simulink library "outp"  (R2021b)
(part 9 of 10)

  VOUTP_EDriveSysErrShifterErr_flg : Outport  Port=497
  VOUTP_LVSysErrPwrOutErr_flg : Outport  Port=498
  VOUTP_HVRlyOpFail_flg : Outport  Port=499
  VOUTP_MCUActDisFail_flg : Outport  Port=500
  VOUTP_VCUBrkSWSta_enum : Outport  Port=501
  VOUTP_VCUFLDoorSta_flg : Outport  Port=502
  VOUTP_VCUFRDoorSta_flg : Outport  Port=503
  VOUTP_VCURLDoorSta_flg : Outport  Port=504
  VOUTP_VCURRDoorSta_flg : Outport  Port=505
  VOUTP_SysAllowReadySta_flg : Outport  Port=506
  VOUTP_VCUHoodSWSta_flg : Outport  Port=507
  VOUTP_VCUTailgateSWSta_flg : Outport  Port=508
  VOUTP_CAN1BusErrorDTC_raw32 : Outport  Port=509
  VOUTP_CAN2BusErrorDTC_raw32 : Outport  Port=510
  VOUTP_CAN3BusErrorDTC_raw32 : Outport  Port=511
  VOUTP_CAN4BusErrorDTC_raw32 : Outport  Port=512
  VOUTP_CAN5BusErrorDTC_raw32 : Outport  Port=513
  VOUTP_CAN6BusErrorDTC_raw32 : Outport  Port=514
  VOUTP_ActAPSPosn_pct : Outport  Port=515
  VOUTP_EAPS1MIN_pct : Outport  Port=516
  VOUTP_EAPS2MIN_pct : Outport  Port=517
  VOUTP_ResetPedalZeroPosStart_flg : Outport  Port=518
  VOUTP_EAPS1NRM_pct : Outport  Port=519
  VOUTP_EAPS2NRM_pct : Outport  Port=520
  VOUTP_DKCTimeSN_cnt : Outport  Port=521
  VOUTP_DKCAuthSta_enum : Outport  Port=522
  VOUTP_TimeSNDKCFbk_cnt : Outport  Port=523
  VOUTP_KeyMissSta_flg : Outport  Port=524
  VOUTP_KeyModeSta_enum : Outport  Port=525
  VOUTP_DkeyShowIVISta_enum : Outport  Port=526
  VOUTP_KeyAreaPS_enum : Outport  Port=527
  VOUTP_KeyAreaLockUnlock_enum : Outport  Port=528
  VOUTP_PCommandToBCM_enum : Outport  Port=529
  VOUTP_DKeyWelcomeSta_enum : Outport  Port=530
  VOUTP_KeyAreaPTG_enum : Outport  Port=531
  VOUTP_KeyAreaSPTGSta_enum : Outport  Port=532
  VOUTP_UIDLowPowerSta_enum : Outport  Port=533
  VOUTP_DkeyAreaRAPSSta_enum : Outport  Port=534
  VOUTP_ParkingModeCmd_enum : Outport  Port=535
  VOUTP_KeyNumSta_enum : Outport  Port=536
  VOUTP_KeyTypeSta_enum : Outport  Port=537
  VOUTP_FDCDKCAllowSleep_flg : Outport  Port=538
  VOUTP_DISCTurn_flg : Outport  Port=539
  VOUTP_DISCTargetSpd_kph : Outport  Port=540
  VOUTP_DISCSta_enum : Outport  Port=541
  VOUTP_DISCButtSta_flg : Outport  Port=542
  VOUTP_AllCANTxReq_flg : Outport  Port=543
  VOUTP_NMmTxReq_flg : Outport  Port=544
  VOUTP_Awake_enum : Outport  Port=545
  VOUTP_CSB_flg : Outport  Port=546
  VOUTP_ErrorState_enum : Outport  Port=547
  VOUTP_NodeID_enum : Outport  Port=548
  VOUTP_PNI_flg : Outport  Port=549
  VOUTP_RptMsgReq_flg : Outport  Port=550
  VOUTP_WakeUp_enum : Outport  Port=551
  VOUTP_ActiveWU_flg : Outport  Port=552
  VOUTP_SysNMmSta_enum : Outport  Port=553
  VOUTP_NetworkReq_flg : Outport  Port=554
  VOUTP_PowerUpState_enum : Outport  Port=555
  VOUTP_PowerDownState_enum : Outport  Port=556
  VOUTP_PowerUpFault_enum : Outport  Port=557
  VOUTP_PowerDownFault_enum : Outport  Port=558
  VOUTP_ActiveDischargeReq_flg : Outport  Port=559
  VOUTP_DCDCEnaReq_flg : Outport  Port=560
  VOUTP_DCDCVoltSetpoint_V : Outport  Port=561
  VOUTP_HVBatCnctReq_flg : Outport  Port=562
  VOUTP_HVSysReadyToCharge_enum : Outport  Port=563
  VOUTP_PowerSta_enum : Outport  Port=564
  VOUTP_LVPwrSta_flg : Outport  Port=565
  VOUTP_HVPwrSta_flg : Outport  Port=566
  VOUTP_SysPowerMode_enum : Outport  Port=567
  VOUTP_FrMCUEnaReq_flg : Outport  Port=568
  VOUTP_RrMCUEnaReq_flg : Outport  Port=569
  VOUTP_DrivetrainSelect_enum : Outport  Port=570
  VOUTP_DrSeatSta_enum : Outport  Port=571
  VOUTP_PwrStaSelect_enum : Outport  Port=572
  VOUTP_PwrStaConstraint_enum : Outport  Port=573
  VOUTP_TCountSta_enum : Outport  Port=574
  VOUTP_PwrUpReq_enum : Outport  Port=575
  VOUTP_PwrDownReq_enum : Outport  Port=576
  VOUTP_LowSOCWarn_enum : Outport  Port=577
  VOUTP_ReVehThdChkSta_enum : Outport  Port=578
  VOUTP_EvccAplusPwrUpReq_flg : Outport  Port=579
  VOUTP_PwrStaONTOPopReq_flg : Outport  Port=580
  VOUTP_IVIPwrStaONTOPopT_s : Outport  Port=581
  VOUTP_LVChrgHoldTtimer_s : Outport  Port=582
  VOUTP_LVBattChrgTimeCnt_s : Outport  Port=583
  VOUTP_SilentChkAllowSleep_flg : Outport  Port=584
  VOUTP_TimerAllowSleep_flg : Outport  Port=585
  VOUTP_FDADC12VDetAvg_mV : Outport  Port=586
  VOUTP_PMMAllowECUSleep_flg : Outport  Port=587
  VOUTP_LVSilentChrgSta_enum : Outport  Port=588
  VOUTP_LVSilentChrgReq_flg : Outport  Port=589
  VOUTP_LVSilentChrgLv_enum : Outport  Port=590
  VOUTP_CtrlFrPwrStbA1P_flg : Outport  Port=591
  VOUTP_CtrlFrRC1_flg : Outport  Port=592
  VOUTP_CtrlFrBMSCCUCIR_flg : Outport  Port=593
  VOUTP_CtrlFrEDUINVERTER_flg : Outport  Port=594
  VOUTP_HWResetSta_enum : Outport  Port=595
  VOUTP_CtrlDrPwrStbA2_flg : Outport  Port=596
  VOUTP_PwrStaTOSta_enum : Outport  Port=597
  VOUTP_Sched_ChgTOSta_enum : Outport  Port=598
  VOUTP_PwrReq_OTA_enum : Outport  Port=599
  VOUTP_OTAPwrReqOFFChkSta_enum : Outport  Port=600
  VOUTP_OTAPwrReqStdChkSta_enum : Outport  Port=601
  VOUTP_PwrReqRAPSAvail_flg : Outport  Port=602
  VOUTP_HWVer1_cnt : Outport  Port=603
  VOUTP_HWVer2_cnt : Outport  Port=604
  VOUTP_HWVer3_cnt : Outport  Port=605
  VOUTP_CarModel1_cnt : Outport  Port=606
  VOUTP_CarModel2_cnt : Outport  Port=607
  VOUTP_CarModel3_cnt : Outport  Port=608
  VOUTP_ECU1_cnt : Outport  Port=609
  VOUTP_ECU2_cnt : Outport  Port=610
  VOUTP_Major1_cnt : Outport  Port=611
  VOUTP_Major2_cnt : Outport  Port=612
  VOUTP_Minor1_cnt : Outport  Port=613
  VOUTP_Minor2_cnt : Outport  Port=614
  VOUTP_Patch1_cnt : Outport  Port=615
  VOUTP_Patch2_cnt : Outport  Port=616
  VOUTP_Country1_cnt : Outport  Port=617
  VOUTP_Country2_cnt : Outport  Port=618
  VOUTP_Variation_cnt : Outport  Port=619
  VOUTP_Dash1_cnt : Outport  Port=620
  VOUTP_Change1_cnt : Outport  Port=621
  VOUTP_Change2_cnt : Outport  Port=622
  VOUTP_Dash2_cnt : Outport  Port=623
  VOUTP_SHA1_cnt : Outport  Port=624
  VOUTP_SHA2_cnt : Outport  Port=625
  VOUTP_SHA3_cnt : Outport  Port=626
  VOUTP_SHA4_cnt : Outport  Port=627
  VOUTP_SHA5_cnt : Outport  Port=628
  VOUTP_SHA6_cnt : Outport  Port=629
  VOUTP_SHA7_cnt : Outport  Port=630
  VOUTP_SHA8_cnt : Outport  Port=631
  VOUTP_NvWriteReqRisingEdge_flg : Outport  Port=632
  VOUTP_FdcSlpReqRisingEdge_flg : Outport  Port=633
  VOUTP_FdcSlpTime_sec : Outport  Port=634
  VOUTP_PmicBootReason_enum : Outport  Port=635
  VOUTP_WisrBootReason_raw32 : Outport  Port=636
  VOUTP_AcoreRebootCmdACK_flg : Outport  Port=637
  VOUTP_CurrentNmState_enum : Outport  Port=638
  VOUTP_ECUGen1_cnt : Outport  Port=639
  VOUTP_ECUGen2_cnt : Outport  Port=640
  VOUTP_PmicBootPath_raw32 : Outport  Port=641
  VOUTP_DrivingMode_cnt : Outport  Port=642
  VOUTP_ModelYear_cnt : Outport  Port=643
  VOUTP_Var4_cnt : Outport  Port=644
  VOUTP_Var5_cnt : Outport  Port=645
  VOUTP_FDCompCmd_rpm : Outport  Port=646
  VOUTP_FDSOV1Cmd_flg : Outport  Port=647
  VOUTP_FDSOV2Cmd_flg : Outport  Port=648
  VOUTP_FDSOV3Cmd_flg : Outport  Port=649
  VOUTP_FDEXV1Cmd_step : Outport  Port=650
  VOUTP_FDEXV2Cmd_step : Outport  Port=651
  VOUTP_FDSOTXVCmd_flg : Outport  Port=652
  VOUTP_FDFWVCmd_flg : Outport  Port=653
  VOUTP_FDTWVCmd_pct : Outport  Port=654
  VOUTP_FDFrWPTCHeatPwrCmd_W : Outport  Port=655
  VOUTP_CoolgFanActDuty_pct : Outport  Port=656
  VOUTP_FDAGSCmd_enum : Outport  Port=657
  VOUTP_FDEWP1Cmd_enum : Outport  Port=658
  VOUTP_FDEWP2Cmd_enum : Outport  Port=659
  VOUTP_FDEWP3Cmd_enum : Outport  Port=660
  VOUTP_FDFrLeAPTCHeatPwrCmd_W : Outport  Port=661
  VOUTP_FDFrRiAPTCHeatPwrCmd_W : Outport  Port=662
  VOUTP_FDRrAPTCHeatPwrCmd_W : Outport  Port=663
  VOUTP_FDBlowerCmd_pct : Outport  Port=664
  VOUTP_BatteryMode_enum : Outport  Port=665
  VOUTP_EDriveMode_enum : Outport  Port=666
  VOUTP_CabinMode_enum : Outport  Port=667
  VOUTP_CCUACLampSts_flg : Outport  Port=668
  VOUTP_CCUAutoLampSts_flg : Outport  Port=669
  VOUTP_CCUACMaxLampSts_flg : Outport  Port=670
  VOUTP_CCUSyncLampSts_flg : Outport  Port=671
  VOUTP_sigAirIntenZon1St_enum : Outport  Port=672
  VOUTP_sigWindDirZon1St_enum : Outport  Port=673
  VOUTP_sigRecircSt_flg : Outport  Port=674
  VOUTP_sigSetTempZon1St_C : Outport  Port=675
  VOUTP_sigSetTempZon2St_C : Outport  Port=676
  VOUTP_sigClntTHvBattOut_C : Outport  Port=677
  VOUTP_sigCbnSolarLeft_W : Outport  Port=678
  VOUTP_sigClntTHvBattIn_C : Outport  Port=679
  VOUTP_sigCbnSolarRight_W : Outport  Port=680
  VOUTP_sigAmbAirT_C : Outport  Port=681
  VOUTP_sigCbnAirT_C : Outport  Port=682
  VOUTP_ACSubMode_enum : Outport  Port=683
  VOUTP_FDRecyAutoCmd_enum : Outport  Port=684
  VOUTP_ACModeMem_enum : Outport  Port=685
  VOUTP_Face_flg : Outport  Port=686
  VOUTP_Foot_flg : Outport  Port=687
  VOUTP_Frost_flg : Outport  Port=688
  VOUTP_FaceM_flg : Outport  Port=689
  VOUTP_FootM_flg : Outport  Port=690
  VOUTP_CCUSyncSts_flg : Outport  Port=691
  VOUTP_ACForceOFF_flg : Outport  Port=692
  VOUTP_RecAutoFlg_flg : Outport  Port=693
  VOUTP_AirIntenZone1M_enum : Outport  Port=694
  VOUTP_fdefog_flg : Outport  Port=695
  VOUTP_sigSetTempZon2StM_C : Outport  Port=696
  VOUTP_sigDfrstSt_flg : Outport  Port=697
  VOUTP_FDCTHCAirIntZ3Sta_enum : Outport  Port=698
  VOUTP_FDCTHCDrEVentModeSta_enum : Outport  Port=699
  VOUTP_FDCTHCPsEVentModeSta_enum : Outport  Port=700
  VOUTP_FDCTHCDrEVentZSta_enum : Outport  Port=701
  VOUTP_FDCTHCCLEVentZSta_enum : Outport  Port=702
  VOUTP_FDCTHCPsEVentZSta_enum : Outport  Port=703
  VOUTP_FDCTHCCREVentZSta_enum : Outport  Port=704
  VOUTP_FDCTHCDrEVentYSta_enum : Outport  Port=705
  VOUTP_FDCTHCDrVentENSta_flg : Outport  Port=706
  VOUTP_FDCTHCCLEVentYSta_enum : Outport  Port=707
  VOUTP_FDCTHCCLVentENSta_flg : Outport  Port=708
  VOUTP_FDCTHCPsEVentYSta_enum : Outport  Port=709
  VOUTP_FDCTHCPsVentENSta_flg : Outport  Port=710
  VOUTP_FDCTHCCREVentYSta_enum : Outport  Port=711
  VOUTP_FDCTHCCRVentENSta_flg : Outport  Port=712
  VOUTP_FDCTHCMAPTCForceOFFSta_flg : Outport  Port=713
  VOUTP_DrVentEN_flg : Outport  Port=714
  VOUTP_CLVentEN_flg : Outport  Port=715
  VOUTP_PsVentEN_flg : Outport  Port=716
  VOUTP_CRVentEN_flg : Outport  Port=717
  VOUTP_FDCFGSAirIntSta_enum : Outport  Port=718
  VOUTP_FDCFGSChSta_enum : Outport  Port=719
  VOUTP_FDCFGSAirIntCmd_enum : Outport  Port=720
  VOUTP_FDCFGSFuncSta_flg : Outport  Port=721
  VOUTP_FDCFGSChCmd_enum : Outport  Port=722
  VOUTP_FDCFGSIONSWSta_flg : Outport  Port=723
  VOUTP_FDCFGSIONCmd_flg : Outport  Port=724
  VOUTP_FDCFGSLearnCmd_enum : Outport  Port=725
  VOUTP_FDCTHCMPreWPTCHeatSta_enum : Outport  Port=726
  VOUTP_EWPBUflag1_flg : Outport  Port=727
  VOUTP_EWPBUflag2_flg : Outport  Port=728
  VOUTP_EWPBUflag3_flg : Outport  Port=729
  VOUTP_LFBatWarn_flg : Outport  Port=730
  VOUTP_RFBatWarn_flg : Outport  Port=731
  VOUTP_LRBatWarn_flg : Outport  Port=732
  VOUTP_RRBatWarn_flg : Outport  Port=733
  VOUTP_LFWheelPress_raw8 : Outport  Port=734
  VOUTP_RFWheelPress_raw8 : Outport  Port=735
  VOUTP_LRWheelPress_raw8 : Outport  Port=736
  VOUTP_RRWheelPress_raw8 : Outport  Port=737
  VOUTP_LFWheelTemp_C : Outport  Port=738
  VOUTP_RFWheelTemp_C : Outport  Port=739
  VOUTP_LRWheelTemp_C : Outport  Port=740
  VOUTP_RRWheelTemp_C : Outport  Port=741
  VOUTP_LFSensorFail_flg : Outport  Port=742
  VOUTP_RFSensorFail_flg : Outport  Port=743
  VOUTP_LRSensorFail_flg : Outport  Port=744
  VOUTP_RRSensorFail_flg : Outport  Port=745
  VOUTP_LFWheelDebug_flg : Outport  Port=746
  VOUTP_LRWheelDebug_flg : Outport  Port=747
  VOUTP_RFWheelDebug_flg : Outport  Port=748
  VOUTP_RRWheelDebug_flg : Outport  Port=749
  VOUTP_TPMSResButtAllow_flg : Outport  Port=750
  VOUTP_TPMSCaliButtAllow_flg : Outport  Port=751
  VOUTP_LFPressIndi_enum : Outport  Port=752
  VOUTP_RFPressIndi_enum : Outport  Port=753
  VOUTP_LRPressIndi_enum : Outport  Port=754
  VOUTP_RRPressIndi_enum : Outport  Port=755
  VOUTP_TPMSWarnIndi_enum : Outport  Port=756
  VOUTP_LFWheelTmpIndi_flg : Outport  Port=757
  VOUTP_RFWheelTmpIndi_flg : Outport  Port=758
  VOUTP_LRWheelTmpIndi_flg : Outport  Port=759
  VOUTP_RRWheelTmpIndi_flg : Outport  Port=760
  VOUTP_LFWheelPSW_raw8 : Outport  Port=761
  VOUTP_LRWheelPSW_raw8 : Outport  Port=762
  VOUTP_RFWheelPSW_raw8 : Outport  Port=763
  VOUTP_RRWheelPSW_raw8 : Outport  Port=764
  VOUTP_CWheelTips_enum : Outport  Port=765
  VOUTP_AutoLTips_enum : Outport  Port=766
  VOUTP_LFSensorMode_flg : Outport  Port=767
  VOUTP_RFSensorMode_flg : Outport  Port=768
  VOUTP_LRSensorMode_flg : Outport  Port=769
  VOUTP_RRSensorMode_flg : Outport  Port=770
  VOUTP_S1ID_raw32 : Outport  Port=771
  VOUTP_S2ID_raw32 : Outport  Port=772
  VOUTP_S3ID_raw32 : Outport  Port=773
  VOUTP_S4ID_raw32 : Outport  Port=774
  VOUTP_S1L_enum : Outport  Port=775
  VOUTP_S2L_enum : Outport  Port=776
  VOUTP_S3L_enum : Outport  Port=777
  VOUTP_S4L_enum : Outport  Port=778
  VOUTP_ALFin_flg : Outport  Port=779
  VOUTP_LFP20_raw8 : Outport  Port=780
  VOUTP_RFP20_raw8 : Outport  Port=781
  VOUTP_LRP20_raw8 : Outport  Port=782
  VOUTP_RRP20_raw8 : Outport  Port=783
  VOUTP_FAT_flg : Outport  Port=784
  VOUTP_IDin_raw32 : Outport  Port=785
  VOUTP_S1WheelDebugALTU_pct : Outport  Port=786
  VOUTP_S2WheelDebugALTU_pct : Outport  Port=787
  VOUTP_S3WheelDebugALTU_pct : Outport  Port=788
  VOUTP_S4WheelDebugALTU_pct : Outport  Port=789
  VOUTP_ID1messageALTU_raw8 : Outport  Port=790
  VOUTP_ID2messageALTU_raw8 : Outport  Port=791
  VOUTP_ID3messageALTU_raw8 : Outport  Port=792
  VOUTP_ID4messageALTU_raw8 : Outport  Port=793
  VOUTP_Chkfin_flg : Outport  Port=794
  VOUTP_SetIDLoc_flg : Outport  Port=795
  VOUTP_TPMSStorge_flg : Outport  Port=796
  VOUTP_ChkStorge_flg : Outport  Port=797
  VOUTP_TPMSResButt_flg : Outport  Port=798
  VOUTP_LFPindi_enum : Outport  Port=799
  VOUTP_RFPind_enum : Outport  Port=800
  VOUTP_LRPindi_enum : Outport  Port=801
  VOUTP_RRPindi_enum : Outport  Port=802
  VOUTP_WriteChkLFID_raw : Outport  Port=803
  VOUTP_WriteChkRFID_raw : Outport  Port=804
  VOUTP_WriteChkLRID_raw : Outport  Port=805
  VOUTP_WriteChkRRID_raw : Outport  Port=806
  VOUTP_WriteChkfinLFID_raw : Outport  Port=807
  VOUTP_WriteChkfinRFID_raw : Outport  Port=808
  VOUTP_WriteChkfinLRID_raw : Outport  Port=809
  VOUTP_WriteChkfinRRID_raw : Outport  Port=810
  VOUTP_Flashchkdatavalid_enum : Outport  Port=811
  VOUTP_Flashdatavalid_enum : Outport  Port=812
  VOUTP_unlearnSfali_flg : Outport  Port=813
  VOUTP_unlearnSfailvalid_enum : Outport  Port=814
  VOUTP_Prepresstempvalid_enum : Outport  Port=815
  VOUTP_FlashS1ID_raw : Outport  Port=816
  VOUTP_FlashS2ID_raw : Outport  Port=817
  VOUTP_FlashS3ID_raw : Outport  Port=818
  VOUTP_FlashS4ID_raw : Outport  Port=819
  VOUTP_FlashIDvalid_enum : Outport  Port=820
  VOUTP_WritingCnt_enum : Outport  Port=821
  VOUTP_TPMSTLCmd_flg : Outport  Port=822
  VOUTP_LProgress_enum : Outport  Port=823
  VOUTP_TPMSSensorIDRegStart_flg : Outport  Port=824
  VOUTP_ModelVersion_raw : Outport  Port=825
  VOUTP_ModelVersionChksum_raw : Outport  Port=826
  VOUTP_ParkRequest_flg : Outport  Port=827
  VOUTP_TqSourceFr_enum : Outport  Port=828
  VOUTP_TqSourceRr_enum : Outport  Port=829
  VOUTP_FrEDUAvailBrkRgnTq_Nm : Outport  Port=830
  VOUTP_RrEDUAvailBrkRgnTq_Nm : Outport  Port=831
  VOUTP_EVDriveMode_enum : Outport  Port=832
  VOUTP_ShiftGearPosn_enum : Outport  Port=833
  VOUTP_PButtonSta_enum : Outport  Port=834
  VOUTP_FrActvDmpDisabReq_flg : Outport  Port=835
  VOUTP_RrActvDmpDisabReq_flg : Outport  Port=836
  VOUTP_FrRgnDecrSta_flg : Outport  Port=837
  VOUTP_RrRgnDecrSta_flg : Outport  Port=838
  VOUTP_DriverWhlTqDemFr_Nm : Outport  Port=839
  VOUTP_DriverWhlTqDemRr_Nm : Outport  Port=840
  VOUTP_FrEDUActTq_Nm : Outport  Port=841
  VOUTP_RrEDUActTq_Nm : Outport  Port=842
  VOUTP_FrEDURolRgnTq_Nm : Outport  Port=843
  VOUTP_RrEDURolRgnTq_Nm : Outport  Port=844
  VOUTP_FrEDUSpd_rpm : Outport  Port=845
  VOUTP_RrEDUSpd_rpm : Outport  Port=846
  VOUTP_FrEDUSpdValid_flg : Outport  Port=847
  VOUTP_FrEDUAvailBrkRgnTqV_flg : Outport  Port=848
  VOUTP_RrEDUSpdValid_flg : Outport  Port=849
  VOUTP_RrEDUAvailBrkRgnTqV_flg : Outport  Port=850
  VOUTP_RgnAbnorSta_flg : Outport  Port=851
  VOUTP_PTCSPermSta_flg : Outport  Port=852
  VOUTP_FrRgnPermSta_flg : Outport  Port=853
  VOUTP_RrRgnPermSta_flg : Outport  Port=854
  VOUTP_ExternalTqAllow_flg : Outport  Port=855
  VOUTP_FrIdcMin_A : Outport  Port=856
  VOUTP_FrIdcMax_A : Outport  Port=857
  VOUTP_FrUdcMin_V : Outport  Port=858
  VOUTP_FrUdcMax_V : Outport  Port=859
  VOUTP_RrIdcMin_A : Outport  Port=860
  VOUTP_RrIdcMax_A : Outport  Port=861
  VOUTP_RrUdcMin_V : Outport  Port=862
  VOUTP_RrUdcMax_V : Outport  Port=863
  VOUTP_ReBrakeLPReq_flg : Outport  Port=864
  VOUTP_ExtShftAllow_flg : Outport  Port=865
  VOUTP_CreepON_flg : Outport  Port=866
  VOUTP_EquivAccPedalSWSta_flg : Outport  Port=867
  VOUTP_DriveProtEn_flg : Outport  Port=868
  VOUTP_ActParkRequest_flg : Outport  Port=869
  VOUTP_IVIPwrLockSta_enum : Outport  Port=870
  VOUTP_ExtDoorAllow_flg : Outport  Port=871
  VOUTP_OPDHoldLamp_flg : Outport  Port=872
  VOUTP_SaveRegenMode_enum : Outport  Port=873
  VOUTP_FDCVCURegenMode_enum : Outport  Port=874
  VOUTP_SpdCtrlMode_enum : Outport  Port=875
  VOUTP_SpdCtrlSta_flg : Outport  Port=876
  VOUTP_SetSpd_kph : Outport  Port=877
  VOUTP_VehActSpd_kph : Outport  Port=878
  VOUTP_RegenLimIndSta_flg : Outport  Port=879
  VOUTP_SetSpdLimWarn_flg : Outport  Port=880
  VOUTP_FrTMTqReq_Nm : Outport  Port=881
  VOUTP_RrTMTqReq_Nm : Outport  Port=882
  VOUTP_ReqOBCV2LEna_enum : Outport  Port=883
  VOUTP_ReqV2LIVIPopup_enum : Outport  Port=884
  VOUTP_ReqV2LIVIDisChrg_enum : Outport  Port=885
  VOUTP_ReqOBCExtrV2LEna_enum : Outport  Port=886
  VOUTP_ReqOBCIntrV2LEna_enum : Outport  Port=887
  VOUTP_HVPO120VGrpALDSt_enum : Outport  Port=888
  VOUTP_HVPO120VGrpBLDSt_enum : Outport  Port=889
  VOUTP_FeatSetSpdFinal_raw32 : Outport  Port=890
  VOUTP_VehicleSpeed_mph : Outport  Port=891
  VOUTP_VehicleSpeed_kph : Outport  Port=892
  VOUTP_MeterIndSpeed_raw32 : Outport  Port=893
  VOUTP_VMCAEBCtrlAvail_flg : Outport  Port=894
  VOUTP_VMCACCCtrlAvail_flg : Outport  Port=895
  VOUTP_VMCCCCtrlAvail_flg : Outport  Port=896
  VOUTP_VMCMSACtrlAvail_flg : Outport  Port=897
  VOUTP_FeatArbitrSta_enum : Outport  Port=898
  VOUTP_FeatReqSpd_kph : Outport  Port=899
  VOUTP_JerkPCT_pct : Outport  Port=900
  VOUTP_LimitPCT_pct : Outport  Port=901
  VOUTP_FrontRearSlipRatioCtrl_flg : Outport  Port=902
  VOUTP_RearWhlSlipRatioCtrl_flg : Outport  Port=903
  VOUTP_SingleWhlSlipRatioCtrl_flg : Outport  Port=904
  VOUTP_LatAccCtrl_flg : Outport  Port=905
  VOUTP_SafetyCtrl_flg : Outport  Port=906
  VOUTP_SPD2ACCAct_flg : Outport  Port=907
  VOUTP_AccCalcuPID_mps2 : Outport  Port=908
  VOUTP_ISOAccLimit_mps2 : Outport  Port=909
  VOUTP_ISODecLimit_mps2 : Outport  Port=910
  VOUTP_ISOJerkLimit_mps3 : Outport  Port=911
  VOUTP_ACCRequiredAccel_mps2 : Outport  Port=912
  VOUTP_DISCReqAcc_mps2 : Outport  Port=913
  VOUTP_FeatArbitrFinal_enum : Outport  Port=914
  VOUTP_ActACCRequiredAccel_mps2 : Outport  Port=915
  VOUTP_LateralCtrl_flg : Outport  Port=916
  VOUTP_ADASLKASta_enum : Outport  Port=917
  VOUTP_LKAStrToqReq_Nm : Outport  Port=918
  VOUTP_LKATOIFault_flg : Outport  Port=919
  VOUTP_LKATOIAct_enum : Outport  Port=920
  VOUTP_ADASAEBReq_enum : Outport  Port=921
  VOUTP_ADASFaultSta_flg : Outport  Port=922
  VOUTP_AEBVehHoldReq_flg : Outport  Port=923
  VOUTP_ACCVehHoldReq_flg : Outport  Port=924
  VOUTP_ADASDBSReq_enum : Outport  Port=925
  VOUTP_ADASACCSta_enum : Outport  Port=926
  VOUTP_ACCObjDist_m : Outport  Port=927
  VOUTP_ACCObjRelSpd_mps : Outport  Port=928
  VOUTP_TimeGapLevel_enum : Outport  Port=929
  VOUTP_ACCJerkUpperLimit_mps3 : Outport  Port=930
  VOUTP_ACCComfortBandUpper_mps2 : Outport  Port=931
  VOUTP_ACCJerkLowerLimit_mps3 : Outport  Port=932
  VOUTP_ACCComfortBandLower_mps2 : Outport  Port=933
  VOUTP_ADASVehSpdLim_raw32 : Outport  Port=934
  VOUTP_ADASShftPosnReqA_flg : Outport  Port=935
  VOUTP_ADASShftPosnReq_enum : Outport  Port=936
  VOUTP_ADASForceIdle_flg : Outport  Port=937
  VOUTP_HazardWarningReq_flg : Outport  Port=938
  VOUTP_RightTurnLightReq_flg : Outport  Port=939
  VOUTP_LeftTurnLightReq_flg : Outport  Port=940
  VOUTP_ADASFCWSta_enum : Outport  Port=941
  VOUTP_ADASLDWSta_enum : Outport  Port=942
  VOUTP_ADASFltWrnReq_flg : Outport  Port=943
  VOUTP_ACCObjDstLvl_enum : Outport  Port=944
  VOUTP_ForceLowBeam_enum : Outport  Port=945
  VOUTP_ACCTakeoverReq_flg : Outport  Port=946
  VOUTP_ADASWarningMsg_enum : Outport  Port=947
  VOUTP_ADASCAMSpdLim_enum : Outport  Port=948
  VOUTP_TargetType_enum : Outport  Port=949
  VOUTP_ADASSLIFSpdLim_enum : Outport  Port=950
  VOUTP_LKAHODDisplayWarning_flg : Outport  Port=951
  VOUTP_LKAHODSoundWarning_flg : Outport  Port=952
  VOUTP_ADASLFCSta_enum : Outport  Port=953
  VOUTP_ADASLaneModeL_enum : Outport  Port=954
  VOUTP_ADASLaneModeR_enum : Outport  Port=955
  VOUTP_ADASSLIFSta_enum : Outport  Port=956
  VOUTP_ADASISASta_enum : Outport  Port=957
  VOUTP_ADASLDWMute_flg : Outport  Port=958
  VOUTP_ADASFCWMute_flg : Outport  Port=959
  VOUTP_ADASLFCHandsOffWarning_enum : Outport  Port=960
  VOUTP_LVDADisabled_flg : Outport  Port=961
  VOUTP_LVDAMuteSta_enum : Outport  Port=962
  VOUTP_LVDAFailinfo_flg : Outport  Port=963
  VOUTP_LVDAWarning_flg : Outport  Port=964
  VOUTP_LVDAACCStatusInformation_flg : Outport  Port=965
  VOUTP_ADASLFCWarnSound_enum : Outport  Port=966
  VOUTP_FCMACCmode_enum : Outport  Port=967
  VOUTP_ADASLanetypeR_enum : Outport  Port=968
  VOUTP_ADASLanetypeL_enum : Outport  Port=969
  VOUTP_ADASLanecurveL_raw32 : Outport  Port=970
  VOUTP_ADASLanecurveR_raw32 : Outport  Port=971
  VOUTP_ADASAEBSta_enum : Outport  Port=972
  VOUTP_FCMLDWRequest_enum : Outport  Port=973
  VOUTP_FCMLDWFault_flg : Outport  Port=974
  VOUTP_ACCCtrlAvail_flg : Outport  Port=975
  VOUTP_ACCPedalOvrd_flg : Outport  Port=976
  VOUTP_TimeGapCalcu_s : Outport  Port=977
  VOUTP_CCCtrlSta_enum : Outport  Port=978
  VOUTP_MSACtrlSta_enum : Outport  Port=979
  VOUTP_APSCtrlAvail_flg : Outport  Port=980
  VOUTP_APSActive_flg : Outport  Port=981
  VOUTP_APSStaSys_enum : Outport  Port=982
  VOUTP_APSDecReqA_flg : Outport  Port=983
  VOUTP_APSDecReq_mps2 : Outport  Port=984
  VOUTP_APSReq_enum : Outport  Port=985
  VOUTP_LongAcc_Gps : Outport  Port=986
  VOUTP_CCMSASpdWar_flg : Outport  Port=987
  VOUTP_IMUEnaCmd_flg : Outport  Port=988
  VOUTP_CAASCtrlAvail_flg : Outport  Port=989
  VOUTP_CAASActive_flg : Outport  Port=990
  VOUTP_ExtraMSACtrlSta_enum : Outport  Port=991
  VOUTP_CalibratedAccX_G : Outport  Port=992
  VOUTP_CalibratedAccY_G : Outport  Port=993
  VOUTP_CalibratedAccZ_G : Outport  Port=994
  VOUTP_CalibratedGyroX_Dps : Outport  Port=995
  VOUTP_CalibratedGyroY_Dps : Outport  Port=996
  VOUTP_CalibratedGyroZ_Dps : Outport  Port=997
  VOUTP_FDCVMCAPSVRqEPSCtrl_flg : Outport  Port=998
  VOUTP_FDCVMCAPSAngleTarget_deg : Outport  Port=999
  VOUTP_FDCVMCAPSRqEPSCtrl_flg : Outport  Port=1000
  VOUTP_FDCVMCAngCtrlTqWtGn_pct : Outport  Port=1001
  VOUTP_FDCVMCDrInpTqBstAct_flg : Outport  Port=1002
  VOUTP_FDCVMCMaxAngCtrlOutTqLim_Nm : Outport  Port=1003
  VOUTP_FDCVMCDrInpTqBstGn_pct : Outport  Port=1004
  wires:
  VACC_HVTHCMSysAvail_enum/1 -> VACC_HVTHCMSysAvail_enum_Inproc/1  "VACC_HVTHCMSysAvail_enum"
  VACC_HVTHCMSysAvail_enum_Inproc/1 -> UnitConverter1/1
  UnitConverter1/1 -> VOUTP_HVTHCMSysAvail_enum/1  "VOUTP_HVTHCMSysAvail_enum"
  VACC_LVBattVoltSta_enum/1 -> VACC_LVBattVoltSta_enum_Inproc/1  "VACC_LVBattVoltSta_enum"
  VACC_LVBattVoltSta_enum_Inproc/1 -> UnitConverter2/1
  UnitConverter2/1 -> VOUTP_LVBattVoltSta_enum/1  "VOUTP_LVBattVoltSta_enum"
  VACC_VehHVPwrAvail4THCM_W/1 -> VACC_VehHVPwrAvail4THCM_W_Inproc/1  "VACC_VehHVPwrAvail4THCM_W"
  VACC_VehHVPwrAvail4THCM_W_Inproc/1 -> UnitConverter3/1
  UnitConverter3/1 -> VOUTP_VehHVPwrAvail4THCM_W/1  "VOUTP_VehHVPwrAvail4THCM_W"
  VAPM_VehSpeed_kph/1 -> VAPM_VehSpeed_kph_Inproc/1  "VAPM_VehSpeed_kph"
  VAPM_VehSpeed_kph_Inproc/1 -> UnitConverter4/1
  UnitConverter4/1 -> VOUTP_VehSpeed_kph/1  "VOUTP_VehSpeed_kph"
  VAPM_VehSpeedTimeOut_flg/1 -> VAPM_VehSpeedTimeOut_flg_Inproc/1  "VAPM_VehSpeedTimeOut_flg"
  VAPM_VehSpeedTimeOut_flg_Inproc/1 -> UnitConverter5/1
  UnitConverter5/1 -> VOUTP_VehSpeedTimeOut_flg/1  "VOUTP_VehSpeedTimeOut_flg"
  VAPM_FSOffSw_enum/1 -> VAPM_FSOffSw_enum_Inproc/1  "VAPM_FSOffSw_enum"
  VAPM_FSOffSw_enum_Inproc/1 -> UnitConverter6/1
  UnitConverter6/1 -> VOUTP_FSOffSw_enum/1  "VOUTP_FSOffSw_enum"
  VAPM_FSOffSwTimeOut_flg/1 -> VAPM_FSOffSwTimeOut_flg_Inproc/1  "VAPM_FSOffSwTimeOut_flg"
  VAPM_FSOffSwTimeOut_flg_Inproc/1 -> UnitConverter7/1
  UnitConverter7/1 -> VOUTP_FSOffSwTimeOut_flg/1  "VOUTP_FSOffSwTimeOut_flg"
  VAPM_ChrgPlugSta_enum/1 -> VAPM_ChrgPlugSta_enum_Inproc/1  "VAPM_ChrgPlugSta_enum"
  VAPM_ChrgPlugSta_enum_Inproc/1 -> UnitConverter8/1
  UnitConverter8/1 -> VOUTP_ChrgPlugSta_enum/1  "VOUTP_ChrgPlugSta_enum"
  VAPM_PASDRMR_cm/1 -> VAPM_PASDRMR_cm_Inproc/1  "VAPM_PASDRMR_cm"
  VAPM_PASDRMR_cm_Inproc/1 -> UnitConverter9/1
  UnitConverter9/1 -> VOUTP_PASDRMR_cm/1  "VOUTP_PASDRMR_cm"
  VAPM_PASDRML_cm/1 -> VAPM_PASDRML_cm_Inproc/1  "VAPM_PASDRML_cm"
  VAPM_PASDRML_cm_Inproc/1 -> UnitConverter10/1
  UnitConverter10/1 -> VOUTP_PASDRML_cm/1  "VOUTP_PASDRML_cm"
  VAPM_PASDRCR_cm/1 -> VAPM_PASDRCR_cm_Inproc/1  "VAPM_PASDRCR_cm"
  VAPM_PASDRCR_cm_Inproc/1 -> UnitConverter11/1
  UnitConverter11/1 -> VOUTP_PASDRCR_cm/1  "VOUTP_PASDRCR_cm"
  VAPM_PASDRCL_cm/1 -> VAPM_PASDRCL_cm_Inproc/1  "VAPM_PASDRCL_cm"
  VAPM_PASDRCL_cm_Inproc/1 -> UnitConverter12/1
  UnitConverter12/1 -> VOUTP_PASDRCL_cm/1  "VOUTP_PASDRCL_cm"
  VAPM_PASDFMR_cm/1 -> VAPM_PASDFMR_cm_Inproc/1  "VAPM_PASDFMR_cm"
  VAPM_PASDFMR_cm_Inproc/1 -> UnitConverter13/1
  UnitConverter13/1 -> VOUTP_PASDFMR_cm/1  "VOUTP_PASDFMR_cm"
  VAPM_PASDFML_cm/1 -> VAPM_PASDFML_cm_Inproc/1  "VAPM_PASDFML_cm"
  VAPM_PASDFML_cm_Inproc/1 -> UnitConverter14/1
  UnitConverter14/1 -> VOUTP_PASDFML_cm/1  "VOUTP_PASDFML_cm"
  VAPM_PASDFCR_cm/1 -> VAPM_PASDFCR_cm_Inproc/1  "VAPM_PASDFCR_cm"
  VAPM_PASDFCR_cm_Inproc/1 -> UnitConverter15/1
  UnitConverter15/1 -> VOUTP_PASDFCR_cm/1  "VOUTP_PASDFCR_cm"
  VAPM_PASDFCL_cm/1 -> VAPM_PASDFCL_cm_Inproc/1  "VAPM_PASDFCL_cm"
  VAPM_PASDFCL_cm_Inproc/1 -> UnitConverter16/1
  UnitConverter16/1 -> VOUTP_PASDFCL_cm/1  "VOUTP_PASDFCL_cm"
  VAPM_APSDRLR_cm/1 -> VAPM_APSDRLR_cm_Inproc/1  "VAPM_APSDRLR_cm"
  VAPM_APSDRLR_cm_Inproc/1 -> UnitConverter17/1
  UnitConverter17/1 -> VOUTP_APSDRLR_cm/1  "VOUTP_APSDRLR_cm"
  VAPM_APSDRLL_cm/1 -> VAPM_APSDRLL_cm_Inproc/1  "VAPM_APSDRLL_cm"
  VAPM_APSDRLL_cm_Inproc/1 -> UnitConverter18/1
  UnitConverter18/1 -> VOUTP_APSDRLL_cm/1  "VOUTP_APSDRLL_cm"
  VAPM_APSDFLR_cm/1 -> VAPM_APSDFLR_cm_Inproc/1  "VAPM_APSDFLR_cm"
  VAPM_APSDFLR_cm_Inproc/1 -> UnitConverter19/1
  UnitConverter19/1 -> VOUTP_APSDFLR_cm/1  "VOUTP_APSDFLR_cm"
  VAPM_APSDFLL_cm/1 -> VAPM_APSDFLL_cm_Inproc/1  "VAPM_APSDFLL_cm"
  VAPM_APSDFLL_cm_Inproc/1 -> UnitConverter20/1
  UnitConverter20/1 -> VOUTP_APSDFLL_cm/1  "VOUTP_APSDFLL_cm"
  VAPM_PASAFCL_enum/1 -> VAPM_PASAFCL_enum_Inproc/1  "VAPM_PASAFCL_enum"
  VAPM_PASAFCL_enum_Inproc/1 -> UnitConverter21/1
  UnitConverter21/1 -> VOUTP_PASAFCL_enum/1  "VOUTP_PASAFCL_enum"
  VAPM_PASARMR_enum/1 -> VAPM_PASARMR_enum_Inproc/1  "VAPM_PASARMR_enum"
  VAPM_PASARMR_enum_Inproc/1 -> UnitConverter22/1
  UnitConverter22/1 -> VOUTP_PASARMR_enum/1  "VOUTP_PASARMR_enum"
  VAPM_PASARML_enum/1 -> VAPM_PASARML_enum_Inproc/1  "VAPM_PASARML_enum"
  VAPM_PASARML_enum_Inproc/1 -> UnitConverter23/1
  UnitConverter23/1 -> VOUTP_PASARML_enum/1  "VOUTP_PASARML_enum"
  VAPM_PASARCR_enum/1 -> VAPM_PASARCR_enum_Inproc/1  "VAPM_PASARCR_enum"
  VAPM_PASARCR_enum_Inproc/1 -> UnitConverter24/1
  UnitConverter24/1 -> VOUTP_PASARCR_enum/1  "VOUTP_PASARCR_enum"
  VAPM_PASARCL_enum/1 -> VAPM_PASARCL_enum_Inproc/1  "VAPM_PASARCL_enum"
  VAPM_PASARCL_enum_Inproc/1 -> UnitConverter25/1
  UnitConverter25/1 -> VOUTP_PASARCL_enum/1  "VOUTP_PASARCL_enum"
  VAPM_PASAFMR_enum/1 -> VAPM_PASAFMR_enum_Inproc/1  "VAPM_PASAFMR_enum"
  VAPM_PASAFMR_enum_Inproc/1 -> UnitConverter26/1
  UnitConverter26/1 -> VOUTP_PASAFMR_enum/1  "VOUTP_PASAFMR_enum"
  VAPM_PASAFML_enum/1 -> VAPM_PASAFML_enum_Inproc/1  "VAPM_PASAFML_enum"
  VAPM_PASAFML_enum_Inproc/1 -> UnitConverter27/1
  UnitConverter27/1 -> VOUTP_PASAFML_enum/1  "VOUTP_PASAFML_enum"
  VAPM_PASAFCR_enum/1 -> VAPM_PASAFCR_enum_Inproc/1  "VAPM_PASAFCR_enum"
  VAPM_PASAFCR_enum_Inproc/1 -> UnitConverter28/1
  UnitConverter28/1 -> VOUTP_PASAFCR_enum/1  "VOUTP_PASAFCR_enum"
  VAPM_USSStaRMR_flg/1 -> VAPM_USSStaRMR_flg_Inproc/1  "VAPM_USSStaRMR_flg"
  VAPM_USSStaRMR_flg_Inproc/1 -> UnitConverter29/1
  UnitConverter29/1 -> VOUTP_USSStaRMR_flg/1  "VOUTP_USSStaRMR_flg"
  VAPM_USSStaRML_flg/1 -> VAPM_USSStaRML_flg_Inproc/1  "VAPM_USSStaRML_flg"
  VAPM_USSStaRML_flg_Inproc/1 -> UnitConverter30/1
  UnitConverter30/1 -> VOUTP_USSStaRML_flg/1  "VOUTP_USSStaRML_flg"
  VAPM_USSStaRLR_flg/1 -> VAPM_USSStaRLR_flg_Inproc/1  "VAPM_USSStaRLR_flg"
  VAPM_USSStaRLR_flg_Inproc/1 -> UnitConverter31/1
  UnitConverter31/1 -> VOUTP_USSStaRLR_flg/1  "VOUTP_USSStaRLR_flg"
  VAPM_USSStaRLL_flg/1 -> VAPM_USSStaRLL_flg_Inproc/1  "VAPM_USSStaRLL_flg"
  VAPM_USSStaRLL_flg_Inproc/1 -> UnitConverter32/1
  UnitConverter32/1 -> VOUTP_USSStaRLL_flg/1  "VOUTP_USSStaRLL_flg"
  VAPM_USSStaRCR_flg/1 -> VAPM_USSStaRCR_flg_Inproc/1  "VAPM_USSStaRCR_flg"
  VAPM_USSStaRCR_flg_Inproc/1 -> UnitConverter33/1
  UnitConverter33/1 -> VOUTP_USSStaRCR_flg/1  "VOUTP_USSStaRCR_flg"
  VAPM_USSStaRCL_flg/1 -> VAPM_USSStaRCL_flg_Inproc/1  "VAPM_USSStaRCL_flg"
  VAPM_USSStaRCL_flg_Inproc/1 -> UnitConverter34/1
  UnitConverter34/1 -> VOUTP_USSStaRCL_flg/1  "VOUTP_USSStaRCL_flg"
  VAPM_USSStaFMR_flg/1 -> VAPM_USSStaFMR_flg_Inproc/1  "VAPM_USSStaFMR_flg"
  VAPM_USSStaFMR_flg_Inproc/1 -> UnitConverter35/1
  UnitConverter35/1 -> VOUTP_USSStaFMR_flg/1  "VOUTP_USSStaFMR_flg"
  VAPM_USSStaFML_flg/1 -> VAPM_USSStaFML_flg_Inproc/1  "VAPM_USSStaFML_flg"
  VAPM_USSStaFML_flg_Inproc/1 -> UnitConverter36/1
  UnitConverter36/1 -> VOUTP_USSStaFML_flg/1  "VOUTP_USSStaFML_flg"
  VAPM_USSStaFLR_flg/1 -> VAPM_USSStaFLR_flg_Inproc/1  "VAPM_USSStaFLR_flg"
  VAPM_USSStaFLR_flg_Inproc/1 -> UnitConverter37/1
  UnitConverter37/1 -> VOUTP_USSStaFLR_flg/1  "VOUTP_USSStaFLR_flg"
  VAPM_USSStaFLL_flg/1 -> VAPM_USSStaFLL_flg_Inproc/1  "VAPM_USSStaFLL_flg"
  VAPM_USSStaFLL_flg_Inproc/1 -> UnitConverter38/1
  UnitConverter38/1 -> VOUTP_USSStaFLL_flg/1  "VOUTP_USSStaFLL_flg"
  VAPM_USSStaFCR_flg/1 -> VAPM_USSStaFCR_flg_Inproc/1  "VAPM_USSStaFCR_flg"
  VAPM_USSStaFCR_flg_Inproc/1 -> UnitConverter39/1
  UnitConverter39/1 -> VOUTP_USSStaFCR_flg/1  "VOUTP_USSStaFCR_flg"
  VAPM_USSStaFCL_flg/1 -> VAPM_USSStaFCL_flg_Inproc/1  "VAPM_USSStaFCL_flg"
  VAPM_USSStaFCL_flg_Inproc/1 -> UnitConverter40/1
  UnitConverter40/1 -> VOUTP_USSStaFCL_flg/1  "VOUTP_USSStaFCL_flg"
  VAPM_Chime_enum/1 -> VAPM_Chime_enum_Inproc/1  "VAPM_Chime_enum"
  VAPM_Chime_enum_Inproc/1 -> UnitConverter41/1
  UnitConverter41/1 -> VOUTP_Chime_enum/1  "VOUTP_Chime_enum"
  VAPM_SNSRLayout_enum/1 -> VAPM_SNSRLayout_enum_Inproc/1  "VAPM_SNSRLayout_enum"
  VAPM_SNSRLayout_enum_Inproc/1 -> UnitConverter42/1
  UnitConverter42/1 -> VOUTP_SNSRLayout_enum/1  "VOUTP_SNSRLayout_enum"
  VAPM_StaFSya_flg/1 -> VAPM_StaFSya_flg_Inproc/1  "VAPM_StaFSya_flg"
  VAPM_StaFSya_flg_Inproc/1 -> UnitConverter43/1
  UnitConverter43/1 -> VOUTP_StaFSya_flg/1  "VOUTP_StaFSya_flg"
  VAPM_ModOperation_enum/1 -> VAPM_ModOperation_enum_Inproc/1  "VAPM_ModOperation_enum"
  VAPM_ModOperation_enum_Inproc/1 -> UnitConverter44/1
  UnitConverter44/1 -> VOUTP_ModOperation_enum/1  "VOUTP_ModOperation_enum"
  VAPM_BrkPedalPos_pct/1 -> VAPM_BrkPedalPos_pct_Inproc/1  "VAPM_BrkPedalPos_pct"
  VAPM_BrkPedalPos_pct_Inproc/1 -> UnitConverter45/1
  UnitConverter45/1 -> VOUTP_BrkPedalPos_pct/1  "VOUTP_BrkPedalPos_pct"
  VAPM_BrkPedalPosTimeOut_flg/1 -> VAPM_BrkPedalPosTimeOut_flg_Inproc/1  "VAPM_BrkPedalPosTimeOut_flg"
  VAPM_BrkPedalPosTimeOut_flg_Inproc/1 -> UnitConverter46/1
  UnitConverter46/1 -> VOUTP_BrkPedalPosTimeOut_flg/1  "VOUTP_BrkPedalPosTimeOut_flg"
  VAPM_LFRawWhlSpeed_kph/1 -> VAPM_LFRawWhlSpeed_kph_Inproc/1  "VAPM_LFRawWhlSpeed_kph"
  VAPM_LFRawWhlSpeed_kph_Inproc/1 -> UnitConverter47/1
  UnitConverter47/1 -> VOUTP_LFRawWhlSpeed_kph/1  "VOUTP_LFRawWhlSpeed_kph"
  VAPM_LFRawWhlSpeedTimeOut_flg/1 -> VAPM_LFRawWhlSpeedTimeOut_flg_Inproc/1  "VAPM_LFRawWhlSpeedTimeOut_flg"
  VAPM_LFRawWhlSpeedTimeOut_flg_Inproc/1 -> UnitConverter48/1
  UnitConverter48/1 -> VOUTP_LFRawWhlSpeedTimeOut_flg/1  "VOUTP_LFRawWhlSpeedTimeOut_flg"
  VAPM_RFRawWhlSpeed_kph/1 -> VAPM_RFRawWhlSpeed_kph_Inproc/1  "VAPM_RFRawWhlSpeed_kph"
  VAPM_RFRawWhlSpeed_kph_Inproc/1 -> UnitConverter49/1
  UnitConverter49/1 -> VOUTP_RFRawWhlSpeed_kph/1  "VOUTP_RFRawWhlSpeed_kph"
  VAPM_RFRawWhlSpeedTimeOut_flg/1 -> VAPM_RFRawWhlSpeedTimeOut_flg_Inproc/1  "VAPM_RFRawWhlSpeedTimeOut_flg"
  VAPM_RFRawWhlSpeedTimeOut_flg_Inproc/1 -> UnitConverter50/1
  UnitConverter50/1 -> VOUTP_RFRawWhlSpeedTimeOut_flg/1  "VOUTP_RFRawWhlSpeedTimeOut_flg"
  VAPM_LRRawWhlSpeed_kph/1 -> VAPM_LRRawWhlSpeed_kph_Inproc/1  "VAPM_LRRawWhlSpeed_kph"
  VAPM_LRRawWhlSpeed_kph_Inproc/1 -> UnitConverter51/1
  UnitConverter51/1 -> VOUTP_LRRawWhlSpeed_kph/1  "VOUTP_LRRawWhlSpeed_kph"
  VAPM_LRRawWhlSpeedTimeOut_flg/1 -> VAPM_LRRawWhlSpeedTimeOut_flg_Inproc/1  "VAPM_LRRawWhlSpeedTimeOut_flg"
  VAPM_LRRawWhlSpeedTimeOut_flg_Inproc/1 -> UnitConverter52/1
  UnitConverter52/1 -> VOUTP_LRRawWhlSpeedTimeOut_flg/1  "VOUTP_LRRawWhlSpeedTimeOut_flg"
  VAPM_RRRawWhlSpeed_kph/1 -> VAPM_RRRawWhlSpeed_kph_Inproc/1  "VAPM_RRRawWhlSpeed_kph"
  VAPM_RRRawWhlSpeed_kph_Inproc/1 -> UnitConverter53/1
  UnitConverter53/1 -> VOUTP_RRRawWhlSpeed_kph/1  "VOUTP_RRRawWhlSpeed_kph"
  VAPM_RRRawWhlSpeedTimeOut_flg/1 -> VAPM_RRRawWhlSpeedTimeOut_flg_Inproc/1  "VAPM_RRRawWhlSpeedTimeOut_flg"
  VAPM_RRRawWhlSpeedTimeOut_flg_Inproc/1 -> UnitConverter54/1
  UnitConverter54/1 -> VOUTP_RRRawWhlSpeedTimeOut_flg/1  "VOUTP_RRRawWhlSpeedTimeOut_flg"
  VAPM_LFRawWhlSpeedV_flg/1 -> VAPM_LFRawWhlSpeedV_flg_Inproc/1  "VAPM_LFRawWhlSpeedV_flg"
  VAPM_LFRawWhlSpeedV_flg_Inproc/1 -> UnitConverter55/1
  UnitConverter55/1 -> VOUTP_LFRawWhlSpeedV_flg/1  "VOUTP_LFRawWhlSpeedV_flg"
  VAPM_LFRawWhlSpeedVTimeOut_flg/1 -> VAPM_LFRawWhlSpeedVTimeOut_flg_Inproc/1  "VAPM_LFRawWhlSpeedVTimeOut_flg"
  VAPM_LFRawWhlSpeedVTimeOut_flg_Inproc/1 -> UnitConverter56/1
  UnitConverter56/1 -> VOUTP_LFRawWhlSpeedVTimeOut_flg/1  "VOUTP_LFRawWhlSpeedVTimeOut_flg"
  VAPM_RFRawWhlSpeedV_flg/1 -> VAPM_RFRawWhlSpeedV_flg_Inproc/1  "VAPM_RFRawWhlSpeedV_flg"
  VAPM_RFRawWhlSpeedV_flg_Inproc/1 -> UnitConverter57/1
  UnitConverter57/1 -> VOUTP_RFRawWhlSpeedV_flg/1  "VOUTP_RFRawWhlSpeedV_flg"
  VAPM_RFRawWhlSpeedVTimeOut_flg/1 -> VAPM_RFRawWhlSpeedVTimeOut_flg_Inproc/1  "VAPM_RFRawWhlSpeedVTimeOut_flg"
  VAPM_RFRawWhlSpeedVTimeOut_flg_Inproc/1 -> UnitConverter58/1
  UnitConverter58/1 -> VOUTP_RFRawWhlSpeedVTimeOut_flg/1  "VOUTP_RFRawWhlSpeedVTimeOut_flg"
  VAPM_LRRawWhlSpeedV_flg/1 -> VAPM_LRRawWhlSpeedV_flg_Inproc/1  "VAPM_LRRawWhlSpeedV_flg"
  VAPM_LRRawWhlSpeedV_flg_Inproc/1 -> UnitConverter59/1
  UnitConverter59/1 -> VOUTP_LRRawWhlSpeedV_flg/1  "VOUTP_LRRawWhlSpeedV_flg"
  VAPM_LRRawWhlSpeedVTimeOut_flg/1 -> VAPM_LRRawWhlSpeedVTimeOut_flg_Inproc/1  "VAPM_LRRawWhlSpeedVTimeOut_flg"
  VAPM_LRRawWhlSpeedVTimeOut_flg_Inproc/1 -> UnitConverter60/1
  UnitConverter60/1 -> VOUTP_LRRawWhlSpeedVTimeOut_flg/1  "VOUTP_LRRawWhlSpeedVTimeOut_flg"
  VAPM_RRRawWhlSpeedV_flg/1 -> VAPM_RRRawWhlSpeedV_flg_Inproc/1  "VAPM_RRRawWhlSpeedV_flg"
  VAPM_RRRawWhlSpeedV_flg_Inproc/1 -> UnitConverter61/1
  UnitConverter61/1 -> VOUTP_RRRawWhlSpeedV_flg/1  "VOUTP_RRRawWhlSpeedV_flg"
  VAPM_RRRawWhlSpeedVTimeOut_flg/1 -> VAPM_RRRawWhlSpeedVTimeOut_flg_Inproc/1  "VAPM_RRRawWhlSpeedVTimeOut_flg"
  VAPM_RRRawWhlSpeedVTimeOut_flg_Inproc/1 -> UnitConverter62/1
  UnitConverter62/1 -> VOUTP_RRRawWhlSpeedVTimeOut_flg/1  "VOUTP_RRRawWhlSpeedVTimeOut_flg"
  VAPM_LFWhlRotDir_enum/1 -> VAPM_LFWhlRotDir_enum_Inproc/1  "VAPM_LFWhlRotDir_enum"
  VAPM_LFWhlRotDir_enum_Inproc/1 -> UnitConverter63/1
  UnitConverter63/1 -> VOUTP_LFWhlRotDir_enum/1  "VOUTP_LFWhlRotDir_enum"
  VAPM_LFWhlRotDirTimeOut_flg/1 -> VAPM_LFWhlRotDirTimeOut_flg_Inproc/1  "VAPM_LFWhlRotDirTimeOut_flg"
  VAPM_LFWhlRotDirTimeOut_flg_Inproc/1 -> UnitConverter64/1
  UnitConverter64/1 -> VOUTP_LFWhlRotDirTimeOut_flg/1  "VOUTP_LFWhlRotDirTimeOut_flg"
  VAPM_RFWhlRotDir_enum/1 -> VAPM_RFWhlRotDir_enum_Inproc/1  "VAPM_RFWhlRotDir_enum"
  VAPM_RFWhlRotDir_enum_Inproc/1 -> UnitConverter65/1
  UnitConverter65/1 -> VOUTP_RFWhlRotDir_enum/1  "VOUTP_RFWhlRotDir_enum"
  VAPM_RFWhlRotDirTimeOut_flg/1 -> VAPM_RFWhlRotDirTimeOut_flg_Inproc/1  "VAPM_RFWhlRotDirTimeOut_flg"
  VAPM_RFWhlRotDirTimeOut_flg_Inproc/1 -> UnitConverter66/1
  UnitConverter66/1 -> VOUTP_RFWhlRotDirTimeOut_flg/1  "VOUTP_RFWhlRotDirTimeOut_flg"
  VAPM_LRWhlRotDir_enum/1 -> VAPM_LRWhlRotDir_enum_Inproc/1  "VAPM_LRWhlRotDir_enum"
  VAPM_LRWhlRotDir_enum_Inproc/1 -> UnitConverter67/1
  UnitConverter67/1 -> VOUTP_LRWhlRotDir_enum/1  "VOUTP_LRWhlRotDir_enum"
  VAPM_LRWhlRotDirTimeOut_flg/1 -> VAPM_LRWhlRotDirTimeOut_flg_Inproc/1  "VAPM_LRWhlRotDirTimeOut_flg"
  VAPM_LRWhlRotDirTimeOut_flg_Inproc/1 -> UnitConverter68/1
  UnitConverter68/1 -> VOUTP_LRWhlRotDirTimeOut_flg/1  "VOUTP_LRWhlRotDirTimeOut_flg"
  VAPM_RRWhlRotDir_enum/1 -> VAPM_RRWhlRotDir_enum_Inproc/1  "VAPM_RRWhlRotDir_enum"
  VAPM_RRWhlRotDir_enum_Inproc/1 -> UnitConverter69/1
  UnitConverter69/1 -> VOUTP_RRWhlRotDir_enum/1  "VOUTP_RRWhlRotDir_enum"
  VAPM_RRWhlRotDirTimeOut_flg/1 -> VAPM_RRWhlRotDirTimeOut_flg_Inproc/1  "VAPM_RRWhlRotDirTimeOut_flg"
  VAPM_RRWhlRotDirTimeOut_flg_Inproc/1 -> UnitConverter70/1
  UnitConverter70/1 -> VOUTP_RRWhlRotDirTimeOut_flg/1  "VOUTP_RRWhlRotDirTimeOut_flg"
  VAPM_LFPulseCountV_flg/1 -> VAPM_LFPulseCountV_flg_Inproc/1  "VAPM_LFPulseCountV_flg"
  VAPM_LFPulseCountV_flg_Inproc/1 -> UnitConverter71/1
  UnitConverter71/1 -> VOUTP_LFPulseCountV_flg/1  "VOUTP_LFPulseCountV_flg"
  VAPM_LFPulseCountVTimeOut_flg/1 -> VAPM_LFPulseCountVTimeOut_flg_Inproc/1  "VAPM_LFPulseCountVTimeOut_flg"
  VAPM_LFPulseCountVTimeOut_flg_Inproc/1 -> UnitConverter72/1
  UnitConverter72/1 -> VOUTP_LFPulseCountVTimeOut_flg/1  "VOUTP_LFPulseCountVTimeOut_flg"
  VAPM_RFPulseCountV_flg/1 -> VAPM_RFPulseCountV_flg_Inproc/1  "VAPM_RFPulseCountV_flg"
  VAPM_RFPulseCountV_flg_Inproc/1 -> UnitConverter73/1
  UnitConverter73/1 -> VOUTP_RFPulseCountV_flg/1  "VOUTP_RFPulseCountV_flg"
  VAPM_RFPulseCountVTimeOut_flg/1 -> VAPM_RFPulseCountVTimeOut_flg_Inproc/1  "VAPM_RFPulseCountVTimeOut_flg"
  VAPM_RFPulseCountVTimeOut_flg_Inproc/1 -> UnitConverter74/1
  UnitConverter74/1 -> VOUTP_RFPulseCountVTimeOut_flg/1  "VOUTP_RFPulseCountVTimeOut_flg"
  VAPM_LRPulseCountV_flg/1 -> VAPM_LRPulseCountV_flg_Inproc/1  "VAPM_LRPulseCountV_flg"
  VAPM_LRPulseCountV_flg_Inproc/1 -> UnitConverter75/1
  UnitConverter75/1 -> VOUTP_LRPulseCountV_flg/1  "VOUTP_LRPulseCountV_flg"
  VAPM_LRPulseCountVTimeOut_flg/1 -> VAPM_LRPulseCountVTimeOut_flg_Inproc/1  "VAPM_LRPulseCountVTimeOut_flg"
  VAPM_LRPulseCountVTimeOut_flg_Inproc/1 -> UnitConverter76/1
  UnitConverter76/1 -> VOUTP_LRPulseCountVTimeOut_flg/1  "VOUTP_LRPulseCountVTimeOut_flg"
  VAPM_RRPulseCountV_flg/1 -> VAPM_RRPulseCountV_flg_Inproc/1  "VAPM_RRPulseCountV_flg"
  VAPM_RRPulseCountV_flg_Inproc/1 -> UnitConverter77/1
  UnitConverter77/1 -> VOUTP_RRPulseCountV_flg/1  "VOUTP_RRPulseCountV_flg"
  VAPM_RRPulseCountVTimeOut_flg/1 -> VAPM_RRPulseCountVTimeOut_flg_Inproc/1  "VAPM_RRPulseCountVTimeOut_flg"
  VAPM_RRPulseCountVTimeOut_flg_Inproc/1 -> UnitConverter78/1
  UnitConverter78/1 -> VOUTP_RRPulseCountVTimeOut_flg/1  "VOUTP_RRPulseCountVTimeOut_flg"
  VAPM_LFPulseCount_enum/1 -> VAPM_LFPulseCount_enum_Inproc/1  "VAPM_LFPulseCount_enum"
  VAPM_LFPulseCount_enum_Inproc/1 -> UnitConverter79/1
  UnitConverter79/1 -> VOUTP_LFPulseCount_enum/1  "VOUTP_LFPulseCount_enum"
  VAPM_LFPulseCountTimeOut_flg/1 -> VAPM_LFPulseCountTimeOut_flg_Inproc/1  "VAPM_LFPulseCountTimeOut_flg"
  VAPM_LFPulseCountTimeOut_flg_Inproc/1 -> UnitConverter80/1
  UnitConverter80/1 -> VOUTP_LFPulseCountTimeOut_flg/1  "VOUTP_LFPulseCountTimeOut_flg"
  VAPM_RFPulseCount_enum/1 -> VAPM_RFPulseCount_enum_Inproc/1  "VAPM_RFPulseCount_enum"
  VAPM_RFPulseCount_enum_Inproc/1 -> UnitConverter81/1
  UnitConverter81/1 -> VOUTP_RFPulseCount_enum/1  "VOUTP_RFPulseCount_enum"
  VAPM_RFPulseCountTimeOut_flg/1 -> VAPM_RFPulseCountTimeOut_flg_Inproc/1  "VAPM_RFPulseCountTimeOut_flg"
  VAPM_RFPulseCountTimeOut_flg_Inproc/1 -> UnitConverter82/1
  UnitConverter82/1 -> VOUTP_RFPulseCountTimeOut_flg/1  "VOUTP_RFPulseCountTimeOut_flg"
  VAPM_LRPulseCount_enum/1 -> VAPM_LRPulseCount_enum_Inproc/1  "VAPM_LRPulseCount_enum"
  VAPM_LRPulseCount_enum_Inproc/1 -> UnitConverter83/1
  UnitConverter83/1 -> VOUTP_LRPulseCount_enum/1  "VOUTP_LRPulseCount_enum"
  VAPM_LRPulseCountTimeOut_flg/1 -> VAPM_LRPulseCountTimeOut_flg_Inproc/1  "VAPM_LRPulseCountTimeOut_flg"
  VAPM_LRPulseCountTimeOut_flg_Inproc/1 -> UnitConverter84/1
  UnitConverter84/1 -> VOUTP_LRPulseCountTimeOut_flg/1  "VOUTP_LRPulseCountTimeOut_flg"
  VAPM_RRPulseCount_enum/1 -> VAPM_RRPulseCount_enum_Inproc/1  "VAPM_RRPulseCount_enum"
  VAPM_RRPulseCount_enum_Inproc/1 -> UnitConverter85/1
  UnitConverter85/1 -> VOUTP_RRPulseCount_enum/1  "VOUTP_RRPulseCount_enum"
  VAPM_RRPulseCountTimeOut_flg/1 -> VAPM_RRPulseCountTimeOut_flg_Inproc/1  "VAPM_RRPulseCountTimeOut_flg"
  VAPM_RRPulseCountTimeOut_flg_Inproc/1 -> UnitConverter86/1
  UnitConverter86/1 -> VOUTP_RRPulseCountTimeOut_flg/1  "VOUTP_RRPulseCountTimeOut_flg"
  VAPM_ShifterHandleCmd_enum/1 -> VAPM_ShifterHandleCmd_enum_Inproc/1  "VAPM_ShifterHandleCmd_enum"
  VAPM_ShifterHandleCmd_enum_Inproc/1 -> UnitConverter87/1
  UnitConverter87/1 -> VOUTP_ShifterHandleCmd_enum/1  "VOUTP_ShifterHandleCmd_enum"
  VAPM_ShifterHandleCmdTimeOut_flg/1 -> VAPM_ShifterHandleCmdTimeOut_flg_Inproc/1  "VAPM_ShifterHandleCmdTimeOut_flg"
  VAPM_ShifterHandleCmdTimeOut_flg_Inproc/1 -> UnitConverter88/1
  UnitConverter88/1 -> VOUTP_ShifterHandleCmdTimeOut_flg/1  "VOUTP_ShifterHandleCmdTimeOut_flg"
  VAPM_DriIntend_enum/1 -> VAPM_DriIntend_enum_Inproc/1  "VAPM_DriIntend_enum"
  VAPM_DriIntend_enum_Inproc/1 -> UnitConverter89/1
  UnitConverter89/1 -> VOUTP_DriIntend_enum/1  "VOUTP_DriIntend_enum"
  VAPM_DriIntendTimeOut_flg/1 -> VAPM_DriIntendTimeOut_flg_Inproc/1  "VAPM_DriIntendTimeOut_flg"
  VAPM_DriIntendTimeOut_flg_Inproc/1 -> UnitConverter90/1
  UnitConverter90/1 -> VOUTP_DriIntendTimeOut_flg/1  "VOUTP_DriIntendTimeOut_flg"
  VAPM_EPSAOIControl_enum/1 -> VAPM_EPSAOIControl_enum_Inproc/1  "VAPM_EPSAOIControl_enum"
  VAPM_EPSAOIControl_enum_Inproc/1 -> UnitConverter91/1
  UnitConverter91/1 -> VOUTP_EPSAOIControl_enum/1  "VOUTP_EPSAOIControl_enum"
  VAPM_EPSAOIControlTimeOut_flg/1 -> VAPM_EPSAOIControlTimeOut_flg_Inproc/1  "VAPM_EPSAOIControlTimeOut_flg"
  VAPM_EPSAOIControlTimeOut_flg_Inproc/1 -> UnitConverter92/1
  UnitConverter92/1 -> VOUTP_EPSAOIControlTimeOut_flg/1  "VOUTP_EPSAOIControlTimeOut_flg"
  VAPM_SASAngle_Deg/1 -> VAPM_SASAngle_Deg_Inproc/1  "VAPM_SASAngle_Deg"
  VAPM_SASAngle_Deg_Inproc/1 -> UnitConverter93/1
  UnitConverter93/1 -> VOUTP_SASAngle_Deg/1  "VOUTP_SASAngle_Deg"
  VAPM_SASAngleTimeOut_flg/1 -> VAPM_SASAngleTimeOut_flg_Inproc/1  "VAPM_SASAngleTimeOut_flg"
  VAPM_SASAngleTimeOut_flg_Inproc/1 -> UnitConverter94/1
  UnitConverter94/1 -> VOUTP_SASAngleTimeOut_flg/1  "VOUTP_SASAngleTimeOut_flg"
  VAPM_SASSpeed_degps/1 -> VAPM_SASSpeed_degps_Inproc/1  "VAPM_SASSpeed_degps"
  VAPM_SASSpeed_degps_Inproc/1 -> UnitConverter95/1
  UnitConverter95/1 -> VOUTP_SASSpeed_degps/1  "VOUTP_SASSpeed_degps"
  VAPM_SASSpeedTimeOut_flg/1 -> VAPM_SASSpeedTimeOut_flg_Inproc/1  "VAPM_SASSpeedTimeOut_flg"
  VAPM_SASSpeedTimeOut_flg_Inproc/1 -> UnitConverter96/1
  UnitConverter96/1 -> VOUTP_SASSpeedTimeOut_flg/1  "VOUTP_SASSpeedTimeOut_flg"
  VAPM_SASSpeedValid_flg/1 -> VAPM_SASSpeedValid_flg_Inproc/1  "VAPM_SASSpeedValid_flg"
  VAPM_SASSpeedValid_flg_Inproc/1 -> UnitConverter97/1
  UnitConverter97/1 -> VOUTP_SASSpeedValid_flg/1  "VOUTP_SASSpeedValid_flg"
  VAPM_SASSpeedValidTimeOut_flg/1 -> VAPM_SASSpeedValidTimeOut_flg_Inproc/1  "VAPM_SASSpeedValidTimeOut_flg"
  VAPM_SASSpeedValidTimeOut_flg_Inproc/1 -> UnitConverter98/1
  UnitConverter98/1 -> VOUTP_SASSpeedValidTimeOut_flg/1  "VOUTP_SASSpeedValidTimeOut_flg"
  VAPM_SASCAL_flg/1 -> VAPM_SASCAL_flg_Inproc/1  "VAPM_SASCAL_flg"
  VAPM_SASCAL_flg_Inproc/1 -> UnitConverter99/1
  UnitConverter99/1 -> VOUTP_SASCAL_flg/1  "VOUTP_SASCAL_flg"
  VAPM_SASCALTimeOut_flg/1 -> VAPM_SASCALTimeOut_flg_Inproc/1  "VAPM_SASCALTimeOut_flg"
  VAPM_SASCALTimeOut_flg_Inproc/1 -> UnitConverter100/1
  UnitConverter100/1 -> VOUTP_SASCALTimeOut_flg/1  "VOUTP_SASCALTimeOut_flg"
  VAPM_SASV_flg/1 -> VAPM_SASV_flg_Inproc/1  "VAPM_SASV_flg"
  VAPM_SASV_flg_Inproc/1 -> UnitConverter101/1
  UnitConverter101/1 -> VOUTP_SASV_flg/1  "VOUTP_SASV_flg"
  VAPM_SASVTimeOut_flg/1 -> VAPM_SASVTimeOut_flg_Inproc/1  "VAPM_SASVTimeOut_flg"
  VAPM_SASVTimeOut_flg_Inproc/1 -> UnitConverter102/1
  UnitConverter102/1 -> VOUTP_SASVTimeOut_flg/1  "VOUTP_SASVTimeOut_flg"
  VAPM_GRADE_Deg/1 -> VAPM_GRADE_Deg_Inproc/1  "VAPM_GRADE_Deg"
  VAPM_GRADE_Deg_Inproc/1 -> UnitConverter103/1
  UnitConverter103/1 -> VOUTP_GRADE_Deg/1  "VOUTP_GRADE_Deg"
  VAPM_GRADETimeOut_flg/1 -> VAPM_GRADETimeOut_flg_Inproc/1  "VAPM_GRADETimeOut_flg"
  VAPM_GRADETimeOut_flg_Inproc/1 -> UnitConverter104/1
  UnitConverter104/1 -> VOUTP_GRADETimeOut_flg/1  "VOUTP_GRADETimeOut_flg"
  VAPM_YawRate_degps/1 -> VAPM_YawRate_degps_Inproc/1  "VAPM_YawRate_degps"
  VAPM_YawRate_degps_Inproc/1 -> UnitConverter105/1
  UnitConverter105/1 -> VOUTP_YawRate_degps/1  "VOUTP_YawRate_degps"
  VAPM_YawRateTimeOut_flg/1 -> VAPM_YawRateTimeOut_flg_Inproc/1  "VAPM_YawRateTimeOut_flg"
  VAPM_YawRateTimeOut_flg_Inproc/1 -> UnitConverter106/1
  UnitConverter106/1 -> VOUTP_YawRateTimeOut_flg/1  "VOUTP_YawRateTimeOut_flg"
  VAPM_LatAccel_Gps/1 -> VAPM_LatAccel_Gps_Inproc/1  "VAPM_LatAccel_Gps"
  VAPM_LatAccel_Gps_Inproc/1 -> UnitConverter107/1
  UnitConverter107/1 -> VOUTP_LatAccel_Gps/1  "VOUTP_LatAccel_Gps"
  VAPM_LatAccelTimeOut_flg/1 -> VAPM_LatAccelTimeOut_flg_Inproc/1  "VAPM_LatAccelTimeOut_flg"
  VAPM_LatAccelTimeOut_flg_Inproc/1 -> UnitConverter108/1
  UnitConverter108/1 -> VOUTP_LatAccelTimeOut_flg/1  "VOUTP_LatAccelTimeOut_flg"
  VAPM_LongAccel_Gps/1 -> VAPM_LongAccel_Gps_Inproc/1  "VAPM_LongAccel_Gps"
  VAPM_LongAccel_Gps_Inproc/1 -> UnitConverter109/1
  UnitConverter109/1 -> VOUTP_LongAccel_Gps/1  "VOUTP_LongAccel_Gps"
  VAPM_LongAccelTimeOut_flg/1 -> VAPM_LongAccelTimeOut_flg_Inproc/1  "VAPM_LongAccelTimeOut_flg"
  VAPM_LongAccelTimeOut_flg_Inproc/1 -> UnitConverter110/1
  UnitConverter110/1 -> VOUTP_LongAccelTimeOut_flg/1  "VOUTP_LongAccelTimeOut_flg"
  VAPM_MCPressure_bar/1 -> VAPM_MCPressure_bar_Inproc/1  "VAPM_MCPressure_bar"
  VAPM_MCPressure_bar_Inproc/1 -> UnitConverter111/1
  UnitConverter111/1 -> VOUTP_MCPressure_bar/1  "VOUTP_MCPressure_bar"
  VAPM_MCPressureTimeOut_flg/1 -> VAPM_MCPressureTimeOut_flg_Inproc/1  "VAPM_MCPressureTimeOut_flg"
  VAPM_MCPressureTimeOut_flg_Inproc/1 -> UnitConverter112/1
  UnitConverter112/1 -> VOUTP_MCPressureTimeOut_flg/1  "VOUTP_MCPressureTimeOut_flg"
  VAPM_YawRateV_flg/1 -> VAPM_YawRateV_flg_Inproc/1  "VAPM_YawRateV_flg"
  VAPM_YawRateV_flg_Inproc/1 -> UnitConverter113/1
  UnitConverter113/1 -> VOUTP_YawRateV_flg/1  "VOUTP_YawRateV_flg"
  VAPM_YawRateVTimeOut_flg/1 -> VAPM_YawRateVTimeOut_flg_Inproc/1  "VAPM_YawRateVTimeOut_flg"
  VAPM_YawRateVTimeOut_flg_Inproc/1 -> UnitConverter114/1
  UnitConverter114/1 -> VOUTP_YawRateVTimeOut_flg/1  "VOUTP_YawRateVTimeOut_flg"
  VAPM_LatAccelV_flg/1 -> VAPM_LatAccelV_flg_Inproc/1  "VAPM_LatAccelV_flg"
  VAPM_LatAccelV_flg_Inproc/1 -> UnitConverter115/1
  UnitConverter115/1 -> VOUTP_LatAccelV_flg/1  "VOUTP_LatAccelV_flg"
  VAPM_LatAccelVTimeOut_flg/1 -> VAPM_LatAccelVTimeOut_flg_Inproc/1  "VAPM_LatAccelVTimeOut_flg"
  VAPM_LatAccelVTimeOut_flg_Inproc/1 -> UnitConverter116/1
  UnitConverter116/1 -> VOUTP_LatAccelVTimeOut_flg/1  "VOUTP_LatAccelVTimeOut_flg"
  VAPM_LongAccelV_flg/1 -> VAPM_LongAccelV_flg_Inproc/1  "VAPM_LongAccelV_flg"
  VAPM_LongAccelV_flg_Inproc/1 -> UnitConverter117/1
  UnitConverter117/1 -> VOUTP_LongAccelV_flg/1  "VOUTP_LongAccelV_flg"
  VAPM_LongAccelVTimeOut_flg/1 -> VAPM_LongAccelVTimeOut_flg_Inproc/1  "VAPM_LongAccelVTimeOut_flg"
  VAPM_LongAccelVTimeOut_flg_Inproc/1 -> UnitConverter118/1
  UnitConverter118/1 -> VOUTP_LongAccelVTimeOut_flg/1  "VOUTP_LongAccelVTimeOut_flg"
  VAPM_MCPressureV_bar/1 -> VAPM_MCPressureV_bar_Inproc/1  "VAPM_MCPressureV_bar"
  VAPM_MCPressureV_bar_Inproc/1 -> UnitConverter119/1
  UnitConverter119/1 -> VOUTP_MCPressureV_bar/1  "VOUTP_MCPressureV_bar"
  VAPM_MCPressureVTimeOut_flg/1 -> VAPM_MCPressureVTimeOut_flg_Inproc/1  "VAPM_MCPressureVTimeOut_flg"
  VAPM_MCPressureVTimeOut_flg_Inproc/1 -> UnitConverter120/1
  UnitConverter120/1 -> VOUTP_MCPressureVTimeOut_flg/1  "VOUTP_MCPressureVTimeOut_flg"
  VAPM_BrkSwSta_flg/1 -> VAPM_BrkSwSta_flg_Inproc/1  "VAPM_BrkSwSta_flg"
  VAPM_BrkSwSta_flg_Inproc/1 -> UnitConverter121/1
  UnitConverter121/1 -> VOUTP_BrkSwSta_flg/1  "VOUTP_BrkSwSta_flg"
  VAPM_BrkSwStaTimeOut_flg/1 -> VAPM_BrkSwStaTimeOut_flg_Inproc/1  "VAPM_BrkSwStaTimeOut_flg"
  VAPM_BrkSwStaTimeOut_flg_Inproc/1 -> UnitConverter122/1
  UnitConverter122/1 -> VOUTP_BrkSwStaTimeOut_flg/1  "VOUTP_BrkSwStaTimeOut_flg"
  VAPM_BrkSwV_flg/1 -> VAPM_BrkSwV_flg_Inproc/1  "VAPM_BrkSwV_flg"
  VAPM_BrkSwV_flg_Inproc/1 -> UnitConverter123/1
  UnitConverter123/1 -> VOUTP_BrkSwV_flg/1  "VOUTP_BrkSwV_flg"
  VAPM_BrkSwVTimeOut_flg/1 -> VAPM_BrkSwVTimeOut_flg_Inproc/1  "VAPM_BrkSwVTimeOut_flg"
  VAPM_BrkSwVTimeOut_flg_Inproc/1 -> UnitConverter124/1
  UnitConverter124/1 -> VOUTP_BrkSwVTimeOut_flg/1  "VOUTP_BrkSwVTimeOut_flg"
  VAPM_ESCStandstill_flg/1 -> VAPM_ESCStandstill_flg_Inproc/1  "VAPM_ESCStandstill_flg"
  VAPM_ESCStandstill_flg_Inproc/1 -> UnitConverter125/1
  UnitConverter125/1 -> VOUTP_ESCStandstill_flg/1  "VOUTP_ESCStandstill_flg"
  VAPM_ESCStandstillTimeOut_flg/1 -> VAPM_ESCStandstillTimeOut_flg_Inproc/1  "VAPM_ESCStandstillTimeOut_flg"
  VAPM_ESCStandstillTimeOut_flg_Inproc/1 -> UnitConverter126/1
  UnitConverter126/1 -> VOUTP_ESCStandstillTimeOut_flg/1  "VOUTP_ESCStandstillTimeOut_flg"
  VAPM_ESCAPSSta_enum/1 -> VAPM_ESCAPSSta_enum_Inproc/1  "VAPM_ESCAPSSta_enum"
  VAPM_ESCAPSSta_enum_Inproc/1 -> UnitConverter127/1
  UnitConverter127/1 -> VOUTP_ESCAPSSta_enum/1  "VOUTP_ESCAPSSta_enum"
  VAPM_ESCAPSStaTimeOut_flg/1 -> VAPM_ESCAPSStaTimeOut_flg_Inproc/1  "VAPM_ESCAPSStaTimeOut_flg"
  VAPM_ESCAPSStaTimeOut_flg_Inproc/1 -> UnitConverter128/1
  UnitConverter128/1 -> VOUTP_ESCAPSStaTimeOut_flg/1  "VOUTP_ESCAPSStaTimeOut_flg"
  VAPM_EPBExtReleaseAvail_flg/1 -> VAPM_EPBExtReleaseAvail_flg_Inproc/1  "VAPM_EPBExtReleaseAvail_flg"
  VAPM_EPBExtReleaseAvail_flg_Inproc/1 -> UnitConverter129/1
  UnitConverter129/1 -> VOUTP_EPBExtReleaseAvail_flg/1  "VOUTP_EPBExtReleaseAvail_flg"
  VAPM_EPBExtReleaseAvailTimeOut_flg/1 -> VAPM_EPBExtReleaseAvailTimeOut_flg_Inproc/1  "VAPM_EPBExtReleaseAvailTimeOut_flg"
  VAPM_EPBExtReleaseAvailTimeOut_flg_Inproc/1 -> UnitConverter130/1
  UnitConverter130/1 -> VOUTP_EPBExtReleaseAvailTimeOut_flg/1  "VOUTP_EPBExtReleaseAvailTimeOut_flg"
  VAPM_EPBExtApplyAvail_flg/1 -> VAPM_EPBExtApplyAvail_flg_Inproc/1  "VAPM_EPBExtApplyAvail_flg"
  VAPM_EPBExtApplyAvail_flg_Inproc/1 -> UnitConverter131/1
  UnitConverter131/1 -> VOUTP_EPBExtApplyAvail_flg/1  "VOUTP_EPBExtApplyAvail_flg"
  VAPM_EPBExtApplyAvailTimeOut_flg/1 -> VAPM_EPBExtApplyAvailTimeOut_flg_Inproc/1  "VAPM_EPBExtApplyAvailTimeOut_flg"
  VAPM_EPBExtApplyAvailTimeOut_flg_Inproc/1 -> UnitConverter132/1
  UnitConverter132/1 -> VOUTP_EPBExtApplyAvailTimeOut_flg/1  "VOUTP_EPBExtApplyAvailTimeOut_flg"
  VAPM_EPBErrSta_enum/1 -> VAPM_EPBErrSta_enum_Inproc/1  "VAPM_EPBErrSta_enum"
  VAPM_EPBErrSta_enum_Inproc/1 -> UnitConverter133/1
  UnitConverter133/1 -> VOUTP_EPBErrSta_enum/1  "VOUTP_EPBErrSta_enum"
  VAPM_EPBErrStaTimeOut_flg/1 -> VAPM_EPBErrStaTimeOut_flg_Inproc/1  "VAPM_EPBErrStaTimeOut_flg"
  VAPM_EPBErrStaTimeOut_flg_Inproc/1 -> UnitConverter134/1
  UnitConverter134/1 -> VOUTP_EPBErrStaTimeOut_flg/1  "VOUTP_EPBErrStaTimeOut_flg"
  VAPM_EPBSta_enum/1 -> VAPM_EPBSta_enum_Inproc/1  "VAPM_EPBSta_enum"
  VAPM_EPBSta_enum_Inproc/1 -> UnitConverter135/1
  UnitConverter135/1 -> VOUTP_EPBSta_enum/1  "VOUTP_EPBSta_enum"
  VAPM_EPBStaTimeOut_flg/1 -> VAPM_EPBStaTimeOut_flg_Inproc/1  "VAPM_EPBStaTimeOut_flg"
  VAPM_EPBStaTimeOut_flg_Inproc/1 -> UnitConverter136/1
  UnitConverter136/1 -> VOUTP_EPBStaTimeOut_flg/1  "VOUTP_EPBStaTimeOut_flg"
  VAPM_AVMparkingcancel_enum/1 -> VAPM_AVMparkingcancel_enum_Inproc/1  "VAPM_AVMparkingcancel_enum"
  VAPM_AVMparkingcancel_enum_Inproc/1 -> UnitConverter137/1
  UnitConverter137/1 -> VOUTP_AVMparkingcancel_enum/1  "VOUTP_AVMparkingcancel_enum"
  VAPM_AVMparkingcancelTimeOut_flg/1 -> VAPM_AVMparkingcancelTimeOut_flg_Inproc/1  "VAPM_AVMparkingcancelTimeOut_flg"
  VAPM_AVMparkingcancelTimeOut_flg_Inproc/1 -> UnitConverter138/1
  UnitConverter138/1 -> VOUTP_AVMparkingcancelTimeOut_flg/1  "VOUTP_AVMparkingcancelTimeOut_flg"
  VAPM_AVMparkingexcute_enum/1 -> VAPM_AVMparkingexcute_enum_Inproc/1  "VAPM_AVMparkingexcute_enum"
  VAPM_AVMparkingexcute_enum_Inproc/1 -> UnitConverter139/1
  UnitConverter139/1 -> VOUTP_AVMparkingexcute_enum/1  "VOUTP_AVMparkingexcute_enum"
  VAPM_AVMparkingexcuteTimeOut_flg/1 -> VAPM_AVMparkingexcuteTimeOut_flg_Inproc/1  "VAPM_AVMparkingexcuteTimeOut_flg"
  VAPM_AVMparkingexcuteTimeOut_flg_Inproc/1 -> UnitConverter140/1
  UnitConverter140/1 -> VOUTP_AVMparkingexcuteTimeOut_flg/1  "VOUTP_AVMparkingexcuteTimeOut_flg"
  VAPM_AVMParkingmode_enum/1 -> VAPM_AVMParkingmode_enum_Inproc/1  "VAPM_AVMParkingmode_enum"
  VAPM_AVMParkingmode_enum_Inproc/1 -> UnitConverter141/1
  UnitConverter141/1 -> VOUTP_AVMParkingmode_enum/1  "VOUTP_AVMParkingmode_enum"
  VAPM_AVMParkingmodeTimeOut_flg/1 -> VAPM_AVMParkingmodeTimeOut_flg_Inproc/1  "VAPM_AVMParkingmodeTimeOut_flg"
  VAPM_AVMParkingmodeTimeOut_flg_Inproc/1 -> UnitConverter142/1
  UnitConverter142/1 -> VOUTP_AVMParkingmodeTimeOut_flg/1  "VOUTP_AVMParkingmodeTimeOut_flg"
  VAPM_AVMErrSTA_flg/1 -> VAPM_AVMErrSTA_flg_Inproc/1  "VAPM_AVMErrSTA_flg"
  VAPM_AVMErrSTA_flg_Inproc/1 -> UnitConverter143/1
  UnitConverter143/1 -> VOUTP_AVMErrSTA_flg/1  "VOUTP_AVMErrSTA_flg"
  VAPM_AVMErrSTATimeOut_flg/1 -> VAPM_AVMErrSTATimeOut_flg_Inproc/1  "VAPM_AVMErrSTATimeOut_flg"
  VAPM_AVMErrSTATimeOut_flg_Inproc/1 -> UnitConverter144/1
  UnitConverter144/1 -> VOUTP_AVMErrSTATimeOut_flg/1  "VOUTP_AVMErrSTATimeOut_flg"
  VAPM_IVIStatus_flg/1 -> VAPM_IVIStatus_flg_Inproc/1  "VAPM_IVIStatus_flg"
  VAPM_IVIStatus_flg_Inproc/1 -> UnitConverter145/1
  UnitConverter145/1 -> VOUTP_IVIStatus_flg/1  "VOUTP_IVIStatus_flg"
  VAPM_IVIStatusTimeOut_flg/1 -> VAPM_IVIStatusTimeOut_flg_Inproc/1  "VAPM_IVIStatusTimeOut_flg"
  VAPM_IVIStatusTimeOut_flg_Inproc/1 -> UnitConverter146/1
  UnitConverter146/1 -> VOUTP_IVIStatusTimeOut_flg/1  "VOUTP_IVIStatusTimeOut_flg"
  VAPM_CAASSw_enum/1 -> VAPM_CAASSw_enum_Inproc/1  "VAPM_CAASSw_enum"
  VAPM_CAASSw_enum_Inproc/1 -> UnitConverter147/1
  UnitConverter147/1 -> VOUTP_CAASSw_enum/1  "VOUTP_CAASSw_enum"
  VAPM_CAASSwTimeOut_flg/1 -> VAPM_CAASSwTimeOut_flg_Inproc/1  "VAPM_CAASSwTimeOut_flg"
  VAPM_CAASSwTimeOut_flg_Inproc/1 -> UnitConverter148/1
  UnitConverter148/1 -> VOUTP_CAASSwTimeOut_flg/1  "VOUTP_CAASSwTimeOut_flg"
  VAPM_IVIScreen_enum/1 -> VAPM_IVIScreen_enum_Inproc/1  "VAPM_IVIScreen_enum"
  VAPM_IVIScreen_enum_Inproc/1 -> UnitConverter149/1
  UnitConverter149/1 -> VOUTP_IVIScreen_enum/1  "VOUTP_IVIScreen_enum"
  VAPM_IVIScreenTimeOut_flg/1 -> VAPM_IVIScreenTimeOut_flg_Inproc/1  "VAPM_IVIScreenTimeOut_flg"
  VAPM_IVIScreenTimeOut_flg_Inproc/1 -> UnitConverter150/1
  UnitConverter150/1 -> VOUTP_IVIScreenTimeOut_flg/1  "VOUTP_IVIScreenTimeOut_flg"
  VAPM_ABSActive_flg/1 -> VAPM_ABSActive_flg_Inproc/1  "VAPM_ABSActive_flg"
  VAPM_ABSActive_flg_Inproc/1 -> UnitConverter151/1
  UnitConverter151/1 -> VOUTP_ABSActive_flg/1  "VOUTP_ABSActive_flg"
  VAPM_ABSActiveTimeOut_flg/1 -> VAPM_ABSActiveTimeOut_flg_Inproc/1  "VAPM_ABSActiveTimeOut_flg"
  VAPM_ABSActiveTimeOut_flg_Inproc/1 -> UnitConverter152/1
  UnitConverter152/1 -> VOUTP_ABSActiveTimeOut_flg/1  "VOUTP_ABSActiveTimeOut_flg"
  VAPM_TCSActive_flg/1 -> VAPM_TCSActive_flg_Inproc/1  "VAPM_TCSActive_flg"
  VAPM_TCSActive_flg_Inproc/1 -> UnitConverter153/1
  UnitConverter153/1 -> VOUTP_TCSActive_flg/1  "VOUTP_TCSActive_flg"
  VAPM_TCSActiveTimeOut_flg/1 -> VAPM_TCSActiveTimeOut_flg_Inproc/1  "VAPM_TCSActiveTimeOut_flg"
  VAPM_TCSActiveTimeOut_flg_Inproc/1 -> UnitConverter154/1
  UnitConverter154/1 -> VOUTP_TCSActiveTimeOut_flg/1  "VOUTP_TCSActiveTimeOut_flg"
  VAPM_DriverSeatBeltCmd_flg/1 -> VAPM_DriverSeatBeltCmd_flg_Inproc/1  "VAPM_DriverSeatBeltCmd_flg"
  VAPM_DriverSeatBeltCmd_flg_Inproc/1 -> UnitConverter155/1
  UnitConverter155/1 -> VOUTP_DriverSeatBeltCmd_flg/1  "VOUTP_DriverSeatBeltCmd_flg"
  VAPM_DriverSeatBeltCmdTimeOut_flg/1 -> VAPM_DriverSeatBeltCmdTimeOut_flg_Inproc/1  "VAPM_DriverSeatBeltCmdTimeOut_flg"
  VAPM_DriverSeatBeltCmdTimeOut_flg_Inproc/1 -> UnitConverter156/1
  UnitConverter156/1 -> VOUTP_DriverSeatBeltCmdTimeOut_flg/1  "VOUTP_DriverSeatBeltCmdTimeOut_flg"
  VAPM_APSProgressPCT_pct/1 -> VAPM_APSProgressPCT_pct_Inproc/1  "VAPM_APSProgressPCT_pct"
  VAPM_APSProgressPCT_pct_Inproc/1 -> UnitConverter157/1
  UnitConverter157/1 -> VOUTP_APSProgressPCT_pct/1  "VOUTP_APSProgressPCT_pct"
  VAPM_APSRQDisplay_enum/1 -> VAPM_APSRQDisplay_enum_Inproc/1  "VAPM_APSRQDisplay_enum"
  VAPM_APSRQDisplay_enum_Inproc/1 -> UnitConverter158/1
  UnitConverter158/1 -> VOUTP_APSRQDisplay_enum/1  "VOUTP_APSRQDisplay_enum"
  VAPM_APSSWVer_enum/1 -> VAPM_APSSWVer_enum_Inproc/1  "VAPM_APSSWVer_enum"
  VAPM_APSSWVer_enum_Inproc/1 -> UnitConverter159/1
  UnitConverter159/1 -> VOUTP_APSSWVer_enum/1  "VOUTP_APSSWVer_enum"
  VAPM_APSHWVer_enum/1 -> VAPM_APSHWVer_enum_Inproc/1  "VAPM_APSHWVer_enum"
  VAPM_APSHWVer_enum_Inproc/1 -> UnitConverter160/1
  UnitConverter160/1 -> VOUTP_APSHWVer_enum/1  "VOUTP_APSHWVer_enum"
  VAPM_APSExitCondition_enum/1 -> VAPM_APSExitCondition_enum_Inproc/1  "VAPM_APSExitCondition_enum"
  VAPM_APSExitCondition_enum_Inproc/1 -> UnitConverter161/1
  UnitConverter161/1 -> VOUTP_APSExitCondition_enum/1  "VOUTP_APSExitCondition_enum"
  VAPM_APSAngleTarget_Deg/1 -> VAPM_APSAngleTarget_Deg_Inproc/1  "VAPM_APSAngleTarget_Deg"
  VAPM_APSAngleTarget_Deg_Inproc/1 -> UnitConverter162/1
  UnitConverter162/1 -> VOUTP_APSAngleTarget_Deg/1  "VOUTP_APSAngleTarget_Deg"
  VAPM_APSVRqEPASCtrl_flg/1 -> VAPM_APSVRqEPASCtrl_flg_Inproc/1  "VAPM_APSVRqEPASCtrl_flg"
  VAPM_APSVRqEPASCtrl_flg_Inproc/1 -> UnitConverter163/1
  UnitConverter163/1 -> VOUTP_APSVRqEPASCtrl_flg/1  "VOUTP_APSVRqEPASCtrl_flg"
  VAPM_APSRqEPASCtrl_flg/1 -> VAPM_APSRqEPASCtrl_flg_Inproc/1  "VAPM_APSRqEPASCtrl_flg"
  VAPM_APSRqEPASCtrl_flg_Inproc/1 -> UnitConverter164/1
  UnitConverter164/1 -> VOUTP_APSRqEPASCtrl_flg/1  "VOUTP_APSRqEPASCtrl_flg"
  VAPM_CAASSta_enum/1 -> VAPM_CAASSta_enum_Inproc/1  "VAPM_CAASSta_enum"
  VAPM_CAASSta_enum_Inproc/1 -> UnitConverter165/1
  UnitConverter165/1 -> VOUTP_CAASSta_enum/1  "VOUTP_CAASSta_enum"
  VAPM_DKCPDkeyAreaRAPSSta_enum/1 -> VAPM_DKCPDkeyAreaRAPSSta_enum_Inproc/1  "VAPM_DKCPDkeyAreaRAPSSta_enum"
  VAPM_DKCPDkeyAreaRAPSSta_enum_Inproc/1 -> UnitConverter166/1
  UnitConverter166/1 -> VOUTP_DKCPDkeyAreaRAPSSta_enum/1  "VOUTP_DKCPDkeyAreaRAPSSta_enum"
  VAPM_DKCParkingModeCmd_enum/1 -> VAPM_DKCParkingModeCmd_enum_Inproc/1  "VAPM_DKCParkingModeCmd_enum"
  VAPM_DKCParkingModeCmd_enum_Inproc/1 -> UnitConverter167/1
  UnitConverter167/1 -> VOUTP_DKCParkingModeCmd_enum/1  "VOUTP_DKCParkingModeCmd_enum"
  VAPM_PUIDLowPower_flg/1 -> VAPM_PUIDLowPower_flg_Inproc/1  "VAPM_PUIDLowPower_flg"
  VAPM_PUIDLowPower_flg_Inproc/1 -> UnitConverter168/1
  UnitConverter168/1 -> VOUTP_PUIDLowPower_flg/1  "VOUTP_PUIDLowPower_flg"
  VAPM_CAASVMCReqA_flg/1 -> VAPM_CAASVMCReqA_flg_Inproc/1  "VAPM_CAASVMCReqA_flg"
  VAPM_CAASVMCReqA_flg_Inproc/1 -> UnitConverter169/1
  UnitConverter169/1 -> VOUTP_CAASVMCReqA_flg/1  "VOUTP_CAASVMCReqA_flg"
  VAPM_APSShiftPosnReq_enum/1 -> VAPM_APSShiftPosnReq_enum_Inproc/1  "VAPM_APSShiftPosnReq_enum"
  VAPM_APSShiftPosnReq_enum_Inproc/1 -> UnitConverter170/1
  UnitConverter170/1 -> VOUTP_APSShiftPosnReq_enum/1  "VOUTP_APSShiftPosnReq_enum"
  VAPM_APSSpeedCMD_kph/1 -> VAPM_APSSpeedCMD_kph_Inproc/1  "VAPM_APSSpeedCMD_kph"
  VAPM_APSSpeedCMD_kph_Inproc/1 -> UnitConverter171/1
  UnitConverter171/1 -> VOUTP_APSSpeedCMD_kph/1  "VOUTP_APSSpeedCMD_kph"
  VAPM_APSVMCReqA_flg/1 -> VAPM_APSVMCReqA_flg_Inproc/1  "VAPM_APSVMCReqA_flg"
  VAPM_APSVMCReqA_flg_Inproc/1 -> UnitConverter172/1
  UnitConverter172/1 -> VOUTP_APSVMCReqA_flg/1  "VOUTP_APSVMCReqA_flg"
  VAPM_RAPSBCMLamp_enum/1 -> VAPM_RAPSBCMLamp_enum_Inproc/1  "VAPM_RAPSBCMLamp_enum"
  VAPM_RAPSBCMLamp_enum_Inproc/1 -> UnitConverter173/1
  UnitConverter173/1 -> VOUTP_RAPSBCMLamp_enum/1  "VOUTP_RAPSBCMLamp_enum"
  VAPM_RAPSBCMLockReq_flg/1 -> VAPM_RAPSBCMLockReq_flg_Inproc/1  "VAPM_RAPSBCMLockReq_flg"
  VAPM_RAPSBCMLockReq_flg_Inproc/1 -> UnitConverter174/1
  UnitConverter174/1 -> VOUTP_RAPSBCMLockReq_flg/1  "VOUTP_RAPSBCMLockReq_flg"
  VAPM_APSPwrReq_enum/1 -> VAPM_APSPwrReq_enum_Inproc/1  "VAPM_APSPwrReq_enum"
  VAPM_APSPwrReq_enum_Inproc/1 -> UnitConverter175/1
  UnitConverter175/1 -> VOUTP_APSPwrReq_enum/1  "VOUTP_APSPwrReq_enum"
  VAPM_RAPSErrWarnSta_enum/1 -> VAPM_RAPSErrWarnSta_enum_Inproc/1  "VAPM_RAPSErrWarnSta_enum"
  VAPM_RAPSErrWarnSta_enum_Inproc/1 -> UnitConverter176/1
  UnitConverter176/1 -> VOUTP_RAPSErrWarnSta_enum/1  "VOUTP_RAPSErrWarnSta_enum"
  VAPM_RAPSErrLv1_flg/1 -> VAPM_RAPSErrLv1_flg_Inproc/1  "VAPM_RAPSErrLv1_flg"
  VAPM_RAPSErrLv1_flg_Inproc/1 -> UnitConverter177/1
  UnitConverter177/1 -> VOUTP_RAPSErrLv1_flg/1  "VOUTP_RAPSErrLv1_flg"
  VAPM_IVIUserTakeOverAPSSta_flg/1 -> VAPM_IVIUserTakeOverAPSSta_flg_Inproc/1  "VAPM_IVIUserTakeOverAPSSta_flg"
  VAPM_IVIUserTakeOverAPSSta_flg_Inproc/1 -> UnitConverter178/1
  UnitConverter178/1 -> VOUTP_IVIUserTakeOverAPSSta_flg/1  "VOUTP_IVIUserTakeOverAPSSta_flg"
  VBCM_AntitheftSta_enum/1 -> VBCM_AntitheftSta_enum_Inproc/1  "VBCM_AntitheftSta_enum"
  VBCM_AntitheftSta_enum_Inproc/1 -> UnitConverter179/1
  UnitConverter179/1 -> VOUTP_AntitheftSta_enum/1  "VOUTP_AntitheftSta_enum"
  VBCM_TailgateRemote_enum/1 -> VBCM_TailgateRemote_enum_Inproc/1  "VBCM_TailgateRemote_enum"
  VBCM_TailgateRemote_enum_Inproc/1 -> UnitConverter180/1
  UnitConverter180/1 -> VOUTP_TailgateRemote_enum/1  "VOUTP_TailgateRemote_enum"
  VBCM_HornCtrl_flg/1 -> VBCM_HornCtrl_flg_Inproc/1  "VBCM_HornCtrl_flg"
  VBCM_HornCtrl_flg_Inproc/1 -> UnitConverter181/1
  UnitConverter181/1 -> VOUTP_HornCtrl_flg/1  "VOUTP_HornCtrl_flg"
  VBCM_AllDoorSW_flg/1 -> VBCM_AllDoorSW_flg_Inproc/1  "VBCM_AllDoorSW_flg"
  VBCM_AllDoorSW_flg_Inproc/1 -> UnitConverter182/1
  UnitConverter182/1 -> VOUTP_AllDoorSW_flg/1  "VOUTP_AllDoorSW_flg"
  VBCM_BCMDoorLockSta_flg/1 -> VBCM_BCMDoorLockSta_flg_Inproc/1  "VBCM_BCMDoorLockSta_flg"
  VBCM_BCMDoorLockSta_flg_Inproc/1 -> UnitConverter183/1
  UnitConverter183/1 -> VOUTP_BCMDoorLockSta_flg/1  "VOUTP_BCMDoorLockSta_flg"
  VBCM_AntitheftSeatFlod_flg/1 -> VBCM_AntitheftSeatFlod_flg_Inproc/1  "VBCM_AntitheftSeatFlod_flg"
  VBCM_AntitheftSeatFlod_flg_Inproc/1 -> UnitConverter184/1
  UnitConverter184/1 -> VOUTP_AntitheftSeatFlod_flg/1  "VOUTP_AntitheftSeatFlod_flg"
  VBCM_HoodSW_flg/1 -> VBCM_HoodSW_flg_Inproc/1  "VBCM_HoodSW_flg"
  VBCM_HoodSW_flg_Inproc/1 -> UnitConverter185/1
  UnitConverter185/1 -> VOUTP_HoodSW_flg/1  "VOUTP_HoodSW_flg"
  VBCM_TailgateSW_flg/1 -> VBCM_TailgateSW_flg_Inproc/1  "VBCM_TailgateSW_flg"
  VBCM_TailgateSW_flg_Inproc/1 -> UnitConverter186/1
  UnitConverter186/1 -> VOUTP_TailgateSW_flg/1  "VOUTP_TailgateSW_flg"
  VBCM_DrDoorSW_flg/1 -> VBCM_DrDoorSW_flg_Inproc/1  "VBCM_DrDoorSW_flg"
  VBCM_DrDoorSW_flg_Inproc/1 -> UnitConverter187/1
  UnitConverter187/1 -> VOUTP_DrDoorSW_flg/1  "VOUTP_DrDoorSW_flg"
  VBCM_PsDoorSW_flg/1 -> VBCM_PsDoorSW_flg_Inproc/1  "VBCM_PsDoorSW_flg"
  VBCM_PsDoorSW_flg_Inproc/1 -> UnitConverter188/1
  UnitConverter188/1 -> VOUTP_PsDoorSW_flg/1  "VOUTP_PsDoorSW_flg"
  VBCM_RLDoorSW_flg/1 -> VBCM_RLDoorSW_flg_Inproc/1  "VBCM_RLDoorSW_flg"
  VBCM_RLDoorSW_flg_Inproc/1 -> UnitConverter189/1
  UnitConverter189/1 -> VOUTP_RLDoorSW_flg/1  "VOUTP_RLDoorSW_flg"
  VBCM_RRDoorSW_flg/1 -> VBCM_RRDoorSW_flg_Inproc/1  "VBCM_RRDoorSW_flg"
  VBCM_RRDoorSW_flg_Inproc/1 -> UnitConverter190/1
  UnitConverter190/1 -> VOUTP_RRDoorSW_flg/1  "VOUTP_RRDoorSW_flg"
  VBCM_LockSetting_flg/1 -> VBCM_LockSetting_flg_Inproc/1  "VBCM_LockSetting_flg"
  VBCM_LockSetting_flg_Inproc/1 -> UnitConverter191/1
  UnitConverter191/1 -> VOUTP_LockSetting_flg/1  "VOUTP_LockSetting_flg"
  VBCM_FrChargingDoorCtrl_enum/1 -> VBCM_FrChargingDoorCtrl_enum_Inproc/1  "VBCM_FrChargingDoorCtrl_enum"
  VBCM_FrChargingDoorCtrl_enum_Inproc/1 -> UnitConverter192/1
  UnitConverter192/1 -> VOUTP_FrChargingDoorCtrl_enum/1  "VOUTP_FrChargingDoorCtrl_enum"
  VBCM_RrChargingDoorCtrl_enum/1 -> VBCM_RrChargingDoorCtrl_enum_Inproc/1  "VBCM_RrChargingDoorCtrl_enum"
  VBCM_RrChargingDoorCtrl_enum_Inproc/1 -> UnitConverter193/1
  UnitConverter193/1 -> VOUTP_RrChargingDoorCtrl_enum/1  "VOUTP_RrChargingDoorCtrl_enum"
  VBCM_CrashDetd_flg/1 -> VBCM_CrashDetd_flg_Inproc/1  "VBCM_CrashDetd_flg"
  VBCM_CrashDetd_flg_Inproc/1 -> UnitConverter194/1
  UnitConverter194/1 -> VOUTP_CrashDetd_flg/1  "VOUTP_CrashDetd_flg"
  VBCM_CTDCtrl_enum/1 -> VBCM_CTDCtrl_enum_Inproc/1  "VBCM_CTDCtrl_enum"
  VBCM_CTDCtrl_enum_Inproc/1 -> UnitConverter195/1
  UnitConverter195/1 -> VOUTP_CTDCtrl_enum/1  "VOUTP_CTDCtrl_enum"
  VBCM_DoorLockIND_flg/1 -> VBCM_DoorLockIND_flg_Inproc/1  "VBCM_DoorLockIND_flg"
  VBCM_DoorLockIND_flg_Inproc/1 -> UnitConverter196/1
  UnitConverter196/1 -> VOUTP_DoorLockIND_flg/1  "VOUTP_DoorLockIND_flg"
  VBCM_CTDLockSW_flg/1 -> VBCM_CTDLockSW_flg_Inproc/1  "VBCM_CTDLockSW_flg"
  VBCM_CTDLockSW_flg_Inproc/1 -> UnitConverter197/1
  UnitConverter197/1 -> VOUTP_CTDLockSW_flg/1  "VOUTP_CTDLockSW_flg"
  VBCM_Dimmer_pct/1 -> VBCM_Dimmer_pct_Inproc/1  "VBCM_Dimmer_pct"
  VBCM_Dimmer_pct_Inproc/1 -> UnitConverter198/1
  UnitConverter198/1 -> VOUTP_Dimmer_pct/1  "VOUTP_Dimmer_pct"
  VBCM_DimmerEN_flg/1 -> VBCM_DimmerEN_flg_Inproc/1  "VBCM_DimmerEN_flg"
  VBCM_DimmerEN_flg_Inproc/1 -> UnitConverter199/1
  UnitConverter199/1 -> VOUTP_DimmerEN_flg/1  "VOUTP_DimmerEN_flg"
  VBCM_PosLamp_flg/1 -> VBCM_PosLamp_flg_Inproc/1  "VBCM_PosLamp_flg"
  VBCM_PosLamp_flg_Inproc/1 -> UnitConverter200/1
  UnitConverter200/1 -> VOUTP_PosLamp_flg/1  "VOUTP_PosLamp_flg"
  VBCM_LBeam_flg/1 -> VBCM_LBeam_flg_Inproc/1  "VBCM_LBeam_flg"
  VBCM_LBeam_flg_Inproc/1 -> UnitConverter201/1
  UnitConverter201/1 -> VOUTP_LBeam_flg/1  "VOUTP_LBeam_flg"
  VBCM_HBeam_flg/1 -> VBCM_HBeam_flg_Inproc/1  "VBCM_HBeam_flg"
  VBCM_HBeam_flg_Inproc/1 -> UnitConverter202/1
  UnitConverter202/1 -> VOUTP_HBeam_flg/1  "VOUTP_HBeam_flg"
  VBCM_RrFogLamp_flg/1 -> VBCM_RrFogLamp_flg_Inproc/1  "VBCM_RrFogLamp_flg"
  VBCM_RrFogLamp_flg_Inproc/1 -> UnitConverter203/1
  UnitConverter203/1 -> VOUTP_RrFogLamp_flg/1  "VOUTP_RrFogLamp_flg"
  VBCM_BrakeLamp_flg/1 -> VBCM_BrakeLamp_flg_Inproc/1  "VBCM_BrakeLamp_flg"
  VBCM_BrakeLamp_flg_Inproc/1 -> UnitConverter204/1
  UnitConverter204/1 -> VOUTP_BrakeLamp_flg/1  "VOUTP_BrakeLamp_flg"
  VBCM_ReverseLamp_flg/1 -> VBCM_ReverseLamp_flg_Inproc/1  "VBCM_ReverseLamp_flg"
  VBCM_ReverseLamp_flg_Inproc/1 -> UnitConverter205/1
  UnitConverter205/1 -> VOUTP_ReverseLamp_flg/1  "VOUTP_ReverseLamp_flg"
  VBCM_LDRL_flg/1 -> VBCM_LDRL_flg_Inproc/1  "VBCM_LDRL_flg"
  VBCM_LDRL_flg_Inproc/1 -> UnitConverter206/1
  UnitConverter206/1 -> VOUTP_LDRL_flg/1  "VOUTP_LDRL_flg"
  VBCM_RDRL_flg/1 -> VBCM_RDRL_flg_Inproc/1  "VBCM_RDRL_flg"
  VBCM_RDRL_flg_Inproc/1 -> UnitConverter207/1
  UnitConverter207/1 -> VOUTP_RDRL_flg/1  "VOUTP_RDRL_flg"
  VBCM_LBSD_flg/1 -> VBCM_LBSD_flg_Inproc/1  "VBCM_LBSD_flg"
  VBCM_LBSD_flg_Inproc/1 -> UnitConverter208/1
  UnitConverter208/1 -> VOUTP_LBSD_flg/1  "VOUTP_LBSD_flg"
  VBCM_RBSD_flg/1 -> VBCM_RBSD_flg_Inproc/1  "VBCM_RBSD_flg"
  VBCM_RBSD_flg_Inproc/1 -> UnitConverter209/1
  UnitConverter209/1 -> VOUTP_RBSD_flg/1  "VOUTP_RBSD_flg"
  VBCM_HazardSW_flg/1 -> VBCM_HazardSW_flg_Inproc/1  "VBCM_HazardSW_flg"
  VBCM_HazardSW_flg_Inproc/1 -> UnitConverter210/1
  UnitConverter210/1 -> VOUTP_HazardSW_flg/1  "VOUTP_HazardSW_flg"
  VBCM_LTurnLP_flg/1 -> VBCM_LTurnLP_flg_Inproc/1  "VBCM_LTurnLP_flg"
  VBCM_LTurnLP_flg_Inproc/1 -> UnitConverter211/1
  UnitConverter211/1 -> VOUTP_LTurnLP_flg/1  "VOUTP_LTurnLP_flg"
  VBCM_RTurnLP_flg/1 -> VBCM_RTurnLP_flg_Inproc/1  "VBCM_RTurnLP_flg"
  VBCM_RTurnLP_flg_Inproc/1 -> UnitConverter212/1
  UnitConverter212/1 -> VOUTP_RTurnLP_flg/1  "VOUTP_RTurnLP_flg"
  VBCM_BCMBuzzerReq_flg/1 -> VBCM_BCMBuzzerReq_flg_Inproc/1  "VBCM_BCMBuzzerReq_flg"
  VBCM_BCMBuzzerReq_flg_Inproc/1 -> UnitConverter213/1
  UnitConverter213/1 -> VOUTP_BCMBuzzerReq_flg/1  "VOUTP_BCMBuzzerReq_flg"
  VBCM_MirrorCtrl_enum/1 -> VBCM_MirrorCtrl_enum_Inproc/1  "VBCM_MirrorCtrl_enum"
  VBCM_MirrorCtrl_enum_Inproc/1 -> UnitConverter214/1
  UnitConverter214/1 -> VOUTP_MirrorCtrl_enum/1  "VOUTP_MirrorCtrl_enum"
  VBCM_MirrorDefog_flg/1 -> VBCM_MirrorDefog_flg_Inproc/1  "VBCM_MirrorDefog_flg"
  VBCM_MirrorDefog_flg_Inproc/1 -> UnitConverter215/1
  UnitConverter215/1 -> VOUTP_MirrorDefog_flg/1  "VOUTP_MirrorDefog_flg"
  VBCM_RrDefog_flg/1 -> VBCM_RrDefog_flg_Inproc/1  "VBCM_RrDefog_flg"
  VBCM_RrDefog_flg_Inproc/1 -> UnitConverter216/1
  UnitConverter216/1 -> VOUTP_RrDefog_flg/1  "VOUTP_RrDefog_flg"
  VBCM_RoomLampH_flg/1 -> VBCM_RoomLampH_flg_Inproc/1  "VBCM_RoomLampH_flg"
  VBCM_RoomLampH_flg_Inproc/1 -> UnitConverter217/1
  UnitConverter217/1 -> VOUTP_RoomLampH_flg/1  "VOUTP_RoomLampH_flg"
  VBCM_RoomLampL_flg/1 -> VBCM_RoomLampL_flg_Inproc/1  "VBCM_RoomLampL_flg"
  VBCM_RoomLampL_flg_Inproc/1 -> UnitConverter218/1
  UnitConverter218/1 -> VOUTP_RoomLampL_flg/1  "VOUTP_RoomLampL_flg"
  VBCM_TrunkRel_flg/1 -> VBCM_TrunkRel_flg_Inproc/1  "VBCM_TrunkRel_flg"
  VBCM_TrunkRel_flg_Inproc/1 -> UnitConverter219/1
  UnitConverter219/1 -> VOUTP_TrunkRel_flg/1  "VOUTP_TrunkRel_flg"
  VBCM_TailgateHDSW_flg/1 -> VBCM_TailgateHDSW_flg_Inproc/1  "VBCM_TailgateHDSW_flg"
  VBCM_TailgateHDSW_flg_Inproc/1 -> UnitConverter220/1
  UnitConverter220/1 -> VOUTP_TailgateHDSW_flg/1  "VOUTP_TailgateHDSW_flg"
  VBCM_FrWiperL_flg/1 -> VBCM_FrWiperL_flg_Inproc/1  "VBCM_FrWiperL_flg"
  VBCM_FrWiperL_flg_Inproc/1 -> UnitConverter221/1
  UnitConverter221/1 -> VOUTP_FrWiperL_flg/1  "VOUTP_FrWiperL_flg"
  VBCM_FrWiperH_flg/1 -> VBCM_FrWiperH_flg_Inproc/1  "VBCM_FrWiperH_flg"
  VBCM_FrWiperH_flg_Inproc/1 -> UnitConverter222/1
  UnitConverter222/1 -> VOUTP_FrWiperH_flg/1  "VOUTP_FrWiperH_flg"
  VBCM_RrWiper_flg/1 -> VBCM_RrWiper_flg_Inproc/1  "VBCM_RrWiper_flg"
  VBCM_RrWiper_flg_Inproc/1 -> UnitConverter223/1
  UnitConverter223/1 -> VOUTP_RrWiper_flg/1  "VOUTP_RrWiper_flg"
  VBCM_WasherCtrl_enum/1 -> VBCM_WasherCtrl_enum_Inproc/1  "VBCM_WasherCtrl_enum"
  VBCM_WasherCtrl_enum_Inproc/1 -> UnitConverter224/1
  UnitConverter224/1 -> VOUTP_WasherCtrl_enum/1  "VOUTP_WasherCtrl_enum"
  VBCM_WiperFixMode_flg/1 -> VBCM_WiperFixMode_flg_Inproc/1  "VBCM_WiperFixMode_flg"
  VBCM_WiperFixMode_flg_Inproc/1 -> UnitConverter225/1
  UnitConverter225/1 -> VOUTP_WiperFixMode_flg/1  "VOUTP_WiperFixMode_flg"
  VBCM_AmbLightBreath1_enum/1 -> VBCM_AmbLightBreath1_enum_Inproc/1  "VBCM_AmbLightBreath1_enum"
  VBCM_AmbLightBreath1_enum_Inproc/1 -> UnitConverter226/1
  UnitConverter226/1 -> VOUTP_AmbLightBreath1_enum/1  "VOUTP_AmbLightBreath1_enum"
  VBCM_AmbLightBreath2_enum/1 -> VBCM_AmbLightBreath2_enum_Inproc/1  "VBCM_AmbLightBreath2_enum"
  VBCM_AmbLightBreath2_enum_Inproc/1 -> UnitConverter227/1
  UnitConverter227/1 -> VOUTP_AmbLightBreath2_enum/1  "VOUTP_AmbLightBreath2_enum"
  VBCM_AmbLightBreath3_enum/1 -> VBCM_AmbLightBreath3_enum_Inproc/1  "VBCM_AmbLightBreath3_enum"
  VBCM_AmbLightBreath3_enum_Inproc/1 -> UnitConverter228/1
  UnitConverter228/1 -> VOUTP_AmbLightBreath3_enum/1  "VOUTP_AmbLightBreath3_enum"
  VBCM_AmbLightBreath4_enum/1 -> VBCM_AmbLightBreath4_enum_Inproc/1  "VBCM_AmbLightBreath4_enum"
  VBCM_AmbLightBreath4_enum_Inproc/1 -> UnitConverter229/1
  UnitConverter229/1 -> VOUTP_AmbLightBreath4_enum/1  "VOUTP_AmbLightBreath4_enum"
  VBCM_AmbLightBreath5_enum/1 -> VBCM_AmbLightBreath5_enum_Inproc/1  "VBCM_AmbLightBreath5_enum"
  VBCM_AmbLightBreath5_enum_Inproc/1 -> UnitConverter230/1
  UnitConverter230/1 -> VOUTP_AmbLightBreath5_enum/1  "VOUTP_AmbLightBreath5_enum"
  VBCM_AmbLightBreath6_enum/1 -> VBCM_AmbLightBreath6_enum_Inproc/1  "VBCM_AmbLightBreath6_enum"
  VBCM_AmbLightBreath6_enum_Inproc/1 -> UnitConverter231/1
  UnitConverter231/1 -> VOUTP_AmbLightBreath6_enum/1  "VOUTP_AmbLightBreath6_enum"
  VBCM_AmbLightBrightness1_enum/1 -> VBCM_AmbLightBrightness1_enum_Inproc/1  "VBCM_AmbLightBrightness1_enum"
  VBCM_AmbLightBrightness1_enum_Inproc/1 -> UnitConverter232/1
  UnitConverter232/1 -> VOUTP_AmbLightBrightness1_enum/1  "VOUTP_AmbLightBrightness1_enum"
  VBCM_AmbLightBrightness2_enum/1 -> VBCM_AmbLightBrightness2_enum_Inproc/1  "VBCM_AmbLightBrightness2_enum"
  VBCM_AmbLightBrightness2_enum_Inproc/1 -> UnitConverter233/1
  UnitConverter233/1 -> VOUTP_AmbLightBrightness2_enum/1  "VOUTP_AmbLightBrightness2_enum"
  VBCM_AmbLightBrightness3_enum/1 -> VBCM_AmbLightBrightness3_enum_Inproc/1  "VBCM_AmbLightBrightness3_enum"
  VBCM_AmbLightBrightness3_enum_Inproc/1 -> UnitConverter234/1
  UnitConverter234/1 -> VOUTP_AmbLightBrightness3_enum/1  "VOUTP_AmbLightBrightness3_enum"
  VBCM_AmbLightBrightness4_enum/1 -> VBCM_AmbLightBrightness4_enum_Inproc/1  "VBCM_AmbLightBrightness4_enum"
  VBCM_AmbLightBrightness4_enum_Inproc/1 -> UnitConverter235/1
  UnitConverter235/1 -> VOUTP_AmbLightBrightness4_enum/1  "VOUTP_AmbLightBrightness4_enum"
  VBCM_AmbLightBrightness5_enum/1 -> VBCM_AmbLightBrightness5_enum_Inproc/1  "VBCM_AmbLightBrightness5_enum"
  VBCM_AmbLightBrightness5_enum_Inproc/1 -> UnitConverter236/1
  UnitConverter236/1 -> VOUTP_AmbLightBrightness5_enum/1  "VOUTP_AmbLightBrightness5_enum"
  VBCM_AmbLightBrightness6_enum/1 -> VBCM_AmbLightBrightness6_enum_Inproc/1  "VBCM_AmbLightBrightness6_enum"
  VBCM_AmbLightBrightness6_enum_Inproc/1 -> UnitConverter237/1
  UnitConverter237/1 -> VOUTP_AmbLightBrightness6_enum/1  "VOUTP_AmbLightBrightness6_enum"
  VBCM_AmbLightColor1_enum/1 -> VBCM_AmbLightColor1_enum_Inproc/1  "VBCM_AmbLightColor1_enum"
  VBCM_AmbLightColor1_enum_Inproc/1 -> UnitConverter238/1
  UnitConverter238/1 -> VOUTP_AmbLightColor1_enum/1  "VOUTP_AmbLightColor1_enum"
  VBCM_AmbLightColor2_enum/1 -> VBCM_AmbLightColor2_enum_Inproc/1  "VBCM_AmbLightColor2_enum"
  VBCM_AmbLightColor2_enum_Inproc/1 -> UnitConverter239/1
  UnitConverter239/1 -> VOUTP_AmbLightColor2_enum/1  "VOUTP_AmbLightColor2_enum"
  VBCM_AmbLightColor3_enum/1 -> VBCM_AmbLightColor3_enum_Inproc/1  "VBCM_AmbLightColor3_enum"
  VBCM_AmbLightColor3_enum_Inproc/1 -> UnitConverter240/1
  UnitConverter240/1 -> VOUTP_AmbLightColor3_enum/1  "VOUTP_AmbLightColor3_enum"
  VBCM_AmbLightColor4_enum/1 -> VBCM_AmbLightColor4_enum_Inproc/1  "VBCM_AmbLightColor4_enum"
  VBCM_AmbLightColor4_enum_Inproc/1 -> UnitConverter241/1
  UnitConverter241/1 -> VOUTP_AmbLightColor4_enum/1  "VOUTP_AmbLightColor4_enum"
  VBCM_AmbLightColor5_enum/1 -> VBCM_AmbLightColor5_enum_Inproc/1  "VBCM_AmbLightColor5_enum"
  VBCM_AmbLightColor5_enum_Inproc/1 -> UnitConverter242/1
  UnitConverter242/1 -> VOUTP_AmbLightColor5_enum/1  "VOUTP_AmbLightColor5_enum"
  VBCM_AmbLightColor6_enum/1 -> VBCM_AmbLightColor6_enum_Inproc/1  "VBCM_AmbLightColor6_enum"
  VBCM_AmbLightColor6_enum_Inproc/1 -> UnitConverter243/1
  UnitConverter243/1 -> VOUTP_AmbLightColor6_enum/1  "VOUTP_AmbLightColor6_enum"
  VBCM_LampPwr_flg/1 -> VBCM_LampPwr_flg_Inproc/1  "VBCM_LampPwr_flg"
  VBCM_LampPwr_flg_Inproc/1 -> UnitConverter244/1
  UnitConverter244/1 -> VOUTP_LampPwr_flg/1  "VOUTP_LampPwr_flg"
  VBCM_SPTGDet_flg/1 -> VBCM_SPTGDet_flg_Inproc/1  "VBCM_SPTGDet_flg"
  VBCM_SPTGDet_flg_Inproc/1 -> UnitConverter245/1
  UnitConverter245/1 -> VOUTP_SPTGDet_flg/1  "VOUTP_SPTGDet_flg"
  VBCM_APSOpenPTG_flg/1 -> VBCM_APSOpenPTG_flg_Inproc/1  "VBCM_APSOpenPTG_flg"
  VBCM_APSOpenPTG_flg_Inproc/1 -> UnitConverter246/1
  UnitConverter246/1 -> VOUTP_APSOpenPTG_flg/1  "VOUTP_APSOpenPTG_flg"
  VBCM_FollowMe_flg/1 -> VBCM_FollowMe_flg_Inproc/1  "VBCM_FollowMe_flg"
  VBCM_FollowMe_flg_Inproc/1 -> UnitConverter247/1
  UnitConverter247/1 -> VOUTP_FollowMe_flg/1  "VOUTP_FollowMe_flg"
  VBCM_IVIRST_flg/1 -> VBCM_IVIRST_flg_Inproc/1  "VBCM_IVIRST_flg"
  VBCM_IVIRST_flg_Inproc/1 -> UnitConverter248/1
  UnitConverter248/1 -> VOUTP_IVIRST_flg/1  "VOUTP_IVIRST_flg"
  VBCM_CountAlarm_enum/1 -> VBCM_CountAlarm_enum_Inproc/1  "VBCM_CountAlarm_enum"
  VBCM_CountAlarm_enum_Inproc/1 -> UnitConverter249/1
  UnitConverter249/1 -> VOUTP_CountAlarm_enum/1  "VOUTP_CountAlarm_enum"
  VBCM_MFSWTri_flg/1 -> VBCM_MFSWTri_flg_Inproc/1  "VBCM_MFSWTri_flg"
  VBCM_MFSWTri_flg_Inproc/1 -> UnitConverter250/1
  UnitConverter250/1 -> VOUTP_MFSWTri_flg/1  "VOUTP_MFSWTri_flg"
  VBCM_MirrorFlodPos_flg/1 -> VBCM_MirrorFlodPos_flg_Inproc/1  "VBCM_MirrorFlodPos_flg"
  VBCM_MirrorFlodPos_flg_Inproc/1 -> UnitConverter251/1
  UnitConverter251/1 -> VOUTP_MirrorFlodPos_flg/1  "VOUTP_MirrorFlodPos_flg"
  VBCM_FuelDoorPos_flg/1 -> VBCM_FuelDoorPos_flg_Inproc/1  "VBCM_FuelDoorPos_flg"
  VBCM_FuelDoorPos_flg_Inproc/1 -> UnitConverter252/1
  UnitConverter252/1 -> VOUTP_FuelDoorPos_flg/1  "VOUTP_FuelDoorPos_flg"
  VBCM_MFRDNBrightReq_pct/1 -> VBCM_MFRDNBrightReq_pct_Inproc/1  "VBCM_MFRDNBrightReq_pct"
  VBCM_MFRDNBrightReq_pct_Inproc/1 -> UnitConverter253/1
  UnitConverter253/1 -> VOUTP_MFRDNBrightReq_pct/1  "VOUTP_MFRDNBrightReq_pct"
  VBCM_PTGInnerSW2_enum/1 -> VBCM_PTGInnerSW2_enum_Inproc/1  "VBCM_PTGInnerSW2_enum"
  VBCM_PTGInnerSW2_enum_Inproc/1 -> UnitConverter254/1
  UnitConverter254/1 -> VOUTP_PTGInnerSW2_enum/1  "VOUTP_PTGInnerSW2_enum"
  VBCM_DrvWdwCtrlCmd_pct/1 -> VBCM_DrvWdwCtrlCmd_pct_Inproc/1  "VBCM_DrvWdwCtrlCmd_pct"
  VBCM_DrvWdwCtrlCmd_pct_Inproc/1 -> UnitConverter255/1
  UnitConverter255/1 -> VOUTP_DrvWdwCtrlCmd_pct/1  "VOUTP_DrvWdwCtrlCmd_pct"
  VBCM_PasWdwCtrlCmd_pct/1 -> VBCM_PasWdwCtrlCmd_pct_Inproc/1  "VBCM_PasWdwCtrlCmd_pct"
  VBCM_PasWdwCtrlCmd_pct_Inproc/1 -> UnitConverter256/1
  UnitConverter256/1 -> VOUTP_PasWdwCtrlCmd_pct/1  "VOUTP_PasWdwCtrlCmd_pct"
  VBCM_DrRWdwCtrlCmd_pct/1 -> VBCM_DrRWdwCtrlCmd_pct_Inproc/1  "VBCM_DrRWdwCtrlCmd_pct"
  VBCM_DrRWdwCtrlCmd_pct_Inproc/1 -> UnitConverter257/1
  UnitConverter257/1 -> VOUTP_DrRWdwCtrlCmd_pct/1  "VOUTP_DrRWdwCtrlCmd_pct"
  VBCM_PsRWdwCtrlCmd_pct/1 -> VBCM_PsRWdwCtrlCmd_pct_Inproc/1  "VBCM_PsRWdwCtrlCmd_pct"
  VBCM_PsRWdwCtrlCmd_pct_Inproc/1 -> UnitConverter258/1
  UnitConverter258/1 -> VOUTP_PsRWdwCtrlCmd_pct/1  "VOUTP_PsRWdwCtrlCmd_pct"
  VBCM_APMDoorControlSta_flg/1 -> VBCM_APMDoorControlSta_flg_Inproc/1  "VBCM_APMDoorControlSta_flg"
  VBCM_APMDoorControlSta_flg_Inproc/1 -> UnitConverter259/1
  UnitConverter259/1 -> VOUTP_APMDoorControlSta_flg/1  "VOUTP_APMDoorControlSta_flg"
  VBCM_AmbFunEN_flg/1 -> VBCM_AmbFunEN_flg_Inproc/1  "VBCM_AmbFunEN_flg"
  VBCM_AmbFunEN_flg_Inproc/1 -> UnitConverter260/1
  UnitConverter260/1 -> VOUTP_AmbFunEN_flg/1  "VOUTP_AmbFunEN_flg"
  VBCM_AmbWelEN_flg/1 -> VBCM_AmbWelEN_flg_Inproc/1  "VBCM_AmbWelEN_flg"
  VBCM_AmbWelEN_flg_Inproc/1 -> UnitConverter261/1
  UnitConverter261/1 -> VOUTP_AmbWelEN_flg/1  "VOUTP_AmbWelEN_flg"
  VBCM_AmbDimEN_flg/1 -> VBCM_AmbDimEN_flg_Inproc/1  "VBCM_AmbDimEN_flg"
  VBCM_AmbDimEN_flg_Inproc/1 -> UnitConverter262/1
  UnitConverter262/1 -> VOUTP_AmbDimEN_flg/1  "VOUTP_AmbDimEN_flg"
  VBCM_AmbLinkDriSta_flg/1 -> VBCM_AmbLinkDriSta_flg_Inproc/1  "VBCM_AmbLinkDriSta_flg"
  VBCM_AmbLinkDriSta_flg_Inproc/1 -> UnitConverter263/1
  UnitConverter263/1 -> VOUTP_AmbLinkDriSta_flg/1  "VOUTP_AmbLinkDriSta_flg"
  VBCM_AmbPwrWarnEN_flg/1 -> VBCM_AmbPwrWarnEN_flg_Inproc/1  "VBCM_AmbPwrWarnEN_flg"
  VBCM_AmbPwrWarnEN_flg_Inproc/1 -> UnitConverter264/1
  UnitConverter264/1 -> VOUTP_AmbPwrWarnEN_flg/1  "VOUTP_AmbPwrWarnEN_flg"
  VBCM_AmbODAEN_flg/1 -> VBCM_AmbODAEN_flg_Inproc/1  "VBCM_AmbODAEN_flg"
  VBCM_AmbODAEN_flg_Inproc/1 -> UnitConverter265/1
  UnitConverter265/1 -> VOUTP_AmbODAEN_flg/1  "VOUTP_AmbODAEN_flg"
  VBCM_AmbColorSta_enum/1 -> VBCM_AmbColorSta_enum_Inproc/1  "VBCM_AmbColorSta_enum"
  VBCM_AmbColorSta_enum_Inproc/1 -> UnitConverter266/1
  UnitConverter266/1 -> VOUTP_AmbColorSta_enum/1  "VOUTP_AmbColorSta_enum"
  VBCM_AmbBrightSta_enum/1 -> VBCM_AmbBrightSta_enum_Inproc/1  "VBCM_AmbBrightSta_enum"
  VBCM_AmbBrightSta_enum_Inproc/1 -> UnitConverter267/1
  UnitConverter267/1 -> VOUTP_AmbBrightSta_enum/1  "VOUTP_AmbBrightSta_enum"
  VBCM_LockAlarm_enum/1 -> VBCM_LockAlarm_enum_Inproc/1  "VBCM_LockAlarm_enum"
  VBCM_LockAlarm_enum_Inproc/1 -> UnitConverter268/1
  UnitConverter268/1 -> VOUTP_LockAlarm_enum/1  "VOUTP_LockAlarm_enum"
  VBCM_ATCtrl_enum/1 -> VBCM_ATCtrl_enum_Inproc/1  "VBCM_ATCtrl_enum"
  VBCM_ATCtrl_enum_Inproc/1 -> UnitConverter269/1
  UnitConverter269/1 -> VOUTP_ATCtrl_enum/1  "VOUTP_ATCtrl_enum"
  VBCM_fUnlockSingle_flg/1 -> VBCM_fUnlockSingle_flg_Inproc/1  "VBCM_fUnlockSingle_flg"
  VBCM_fUnlockSingle_flg_Inproc/1 -> UnitConverter270/1
  UnitConverter270/1 -> VOUTP_fUnlockSingle_flg/1  "VOUTP_fUnlockSingle_flg"
  VBCM_UserNow_enum/1 -> VBCM_UserNow_enum_Inproc/1  "VBCM_UserNow_enum"
  VBCM_UserNow_enum_Inproc/1 -> UnitConverter271/1
  UnitConverter271/1 -> VOUTP_UserNow_enum/1  "VOUTP_UserNow_enum"
  VBCM_AmbFunENFlash_enum/1 -> VBCM_AmbFunENFlash_enum_Inproc/1  "VBCM_AmbFunENFlash_enum"
  VBCM_AmbFunENFlash_enum_Inproc/1 -> UnitConverter272/1
  UnitConverter272/1 -> VOUTP_AmbFunENFlash_enum/1  "VOUTP_AmbFunENFlash_enum"
  VBCM_AmbWelENFlash_enum/1 -> VBCM_AmbWelENFlash_enum_Inproc/1  "VBCM_AmbWelENFlash_enum"
  VBCM_AmbWelENFlash_enum_Inproc/1 -> UnitConverter273/1
  UnitConverter273/1 -> VOUTP_AmbWelENFlash_enum/1  "VOUTP_AmbWelENFlash_enum"
  VBCM_AmbDimENFlash_enum/1 -> VBCM_AmbDimENFlash_enum_Inproc/1  "VBCM_AmbDimENFlash_enum"
  VBCM_AmbDimENFlash_enum_Inproc/1 -> UnitConverter274/1
  UnitConverter274/1 -> VOUTP_AmbDimENFlash_enum/1  "VOUTP_AmbDimENFlash_enum"
  VBCM_AmbLinkDriStaFlash_enum/1 -> VBCM_AmbLinkDriStaFlash_enum_Inproc/1  "VBCM_AmbLinkDriStaFlash_enum"
  VBCM_AmbLinkDriStaFlash_enum_Inproc/1 -> UnitConverter275/1
  UnitConverter275/1 -> VOUTP_AmbLinkDriStaFlash_enum/1  "VOUTP_AmbLinkDriStaFlash_enum"
  VBCM_AmbPwrWarnENFlash_enum/1 -> VBCM_AmbPwrWarnENFlash_enum_Inproc/1  "VBCM_AmbPwrWarnENFlash_enum"
  VBCM_AmbPwrWarnENFlash_enum_Inproc/1 -> UnitConverter276/1
  UnitConverter276/1 -> VOUTP_AmbPwrWarnENFlash_enum/1  "VOUTP_AmbPwrWarnENFlash_enum"
  VBCM_AmbODAENFlash_enum/1 -> VBCM_AmbODAENFlash_enum_Inproc/1  "VBCM_AmbODAENFlash_enum"
  VBCM_AmbODAENFlash_enum_Inproc/1 -> UnitConverter277/1
  UnitConverter277/1 -> VOUTP_AmbODAENFlash_enum/1  "VOUTP_AmbODAENFlash_enum"
  VBCM_AmbColorSta1_enum/1 -> VBCM_AmbColorSta1_enum_Inproc/1  "VBCM_AmbColorSta1_enum"
  VBCM_AmbColorSta1_enum_Inproc/1 -> UnitConverter278/1
  UnitConverter278/1 -> VOUTP_AmbColorSta1_enum/1  "VOUTP_AmbColorSta1_enum"
  VBCM_AmbColorSta2_enum/1 -> VBCM_AmbColorSta2_enum_Inproc/1  "VBCM_AmbColorSta2_enum"
  VBCM_AmbColorSta2_enum_Inproc/1 -> UnitConverter279/1
  UnitConverter279/1 -> VOUTP_AmbColorSta2_enum/1  "VOUTP_AmbColorSta2_enum"
  VBCM_AmbColorSta3_enum/1 -> VBCM_AmbColorSta3_enum_Inproc/1  "VBCM_AmbColorSta3_enum"
  VBCM_AmbColorSta3_enum_Inproc/1 -> UnitConverter280/1
  UnitConverter280/1 -> VOUTP_AmbColorSta3_enum/1  "VOUTP_AmbColorSta3_enum"
  VBCM_AmbColorSta4_enum/1 -> VBCM_AmbColorSta4_enum_Inproc/1  "VBCM_AmbColorSta4_enum"
  VBCM_AmbColorSta4_enum_Inproc/1 -> UnitConverter281/1
  UnitConverter281/1 -> VOUTP_AmbColorSta4_enum/1  "VOUTP_AmbColorSta4_enum"
  VBCM_AmbColorSta5_enum/1 -> VBCM_AmbColorSta5_enum_Inproc/1  "VBCM_AmbColorSta5_enum"
  VBCM_AmbColorSta5_enum_Inproc/1 -> UnitConverter282/1
  UnitConverter282/1 -> VOUTP_AmbColorSta5_enum/1  "VOUTP_AmbColorSta5_enum"
  VBCM_AmbColorSta7_enum/1 -> VBCM_AmbColorSta7_enum_Inproc/1  "VBCM_AmbColorSta7_enum"
  VBCM_AmbColorSta7_enum_Inproc/1 -> UnitConverter283/1
  UnitConverter283/1 -> VOUTP_AmbColorSta7_enum/1  "VOUTP_AmbColorSta7_enum"
  VBCM_AmbBrightnessSta1_enum/1 -> VBCM_AmbBrightnessSta1_enum_Inproc/1  "VBCM_AmbBrightnessSta1_enum"
  VBCM_AmbBrightnessSta1_enum_Inproc/1 -> UnitConverter284/1
  UnitConverter284/1 -> VOUTP_AmbBrightnessSta1_enum/1  "VOUTP_AmbBrightnessSta1_enum"
  VBCM_AmbBrightnessSta2_enum/1 -> VBCM_AmbBrightnessSta2_enum_Inproc/1  "VBCM_AmbBrightnessSta2_enum"
  VBCM_AmbBrightnessSta2_enum_Inproc/1 -> UnitConverter285/1
  UnitConverter285/1 -> VOUTP_AmbBrightnessSta2_enum/1  "VOUTP_AmbBrightnessSta2_enum"
  VBCM_AmbBrightnessSta3_enum/1 -> VBCM_AmbBrightnessSta3_enum_Inproc/1  "VBCM_AmbBrightnessSta3_enum"
  VBCM_AmbBrightnessSta3_enum_Inproc/1 -> UnitConverter286/1
  UnitConverter286/1 -> VOUTP_AmbBrightnessSta3_enum/1  "VOUTP_AmbBrightnessSta3_enum"
  VBCM_AmbBrightnessSta4_enum/1 -> VBCM_AmbBrightnessSta4_enum_Inproc/1  "VBCM_AmbBrightnessSta4_enum"
  VBCM_AmbBrightnessSta4_enum_Inproc/1 -> UnitConverter287/1
  UnitConverter287/1 -> VOUTP_AmbBrightnessSta4_enum/1  "VOUTP_AmbBrightnessSta4_enum"
  VBCM_AmbBrightnessSta5_enum/1 -> VBCM_AmbBrightnessSta5_enum_Inproc/1  "VBCM_AmbBrightnessSta5_enum"
  VBCM_AmbBrightnessSta5_enum_Inproc/1 -> UnitConverter288/1
  UnitConverter288/1 -> VOUTP_AmbBrightnessSta5_enum/1  "VOUTP_AmbBrightnessSta5_enum"
  VBCM_AmbBrightnessSta7_enum/1 -> VBCM_AmbBrightnessSta7_enum_Inproc/1  "VBCM_AmbBrightnessSta7_enum"
  VBCM_AmbBrightnessSta7_enum_Inproc/1 -> UnitConverter289/1
  UnitConverter289/1 -> VOUTP_AmbBrightnessSta7_enum/1  "VOUTP_AmbBrightnessSta7_enum"
  VBCM_HazardIND_flg/1 -> VBCM_HazardIND_flg_Inproc/1  "VBCM_HazardIND_flg"
  VBCM_HazardIND_flg_Inproc/1 -> UnitConverter290/1
  UnitConverter290/1 -> VOUTP_HazardIND_flg/1  "VOUTP_HazardIND_flg"
  VBCM_DimSwSta_flg/1 -> VBCM_DimSwSta_flg_Inproc/1  "VBCM_DimSwSta_flg"
  VBCM_DimSwSta_flg_Inproc/1 -> UnitConverter291/1
  UnitConverter291/1 -> VOUTP_DimSwSta_flg/1  "VOUTP_DimSwSta_flg"
  VBCM_PassSWSta_flg/1 -> VBCM_PassSWSta_flg_Inproc/1  "VBCM_PassSWSta_flg"
  VBCM_PassSWSta_flg_Inproc/1 -> UnitConverter292/1
  UnitConverter292/1 -> VOUTP_PassSWSta_flg/1  "VOUTP_PassSWSta_flg"
  VBCM_FWipSwSta_enum/1 -> VBCM_FWipSwSta_enum_Inproc/1  "VBCM_FWipSwSta_enum"
  VBCM_FWipSwSta_enum_Inproc/1 -> UnitConverter293/1
  UnitConverter293/1 -> VOUTP_FWipSwSta_enum/1  "VOUTP_FWipSwSta_enum"
  VBCM_FWasSwSta_enum/1 -> VBCM_FWasSwSta_enum_Inproc/1  "VBCM_FWasSwSta_enum"
  VBCM_FWasSwSta_enum_Inproc/1 -> UnitConverter294/1
  UnitConverter294/1 -> VOUTP_FWasSwSta_enum/1  "VOUTP_FWasSwSta_enum"
  VBCM_TurnSwSta_enum/1 -> VBCM_TurnSwSta_enum_Inproc/1  "VBCM_TurnSwSta_enum"
  VBCM_TurnSwSta_enum_Inproc/1 -> UnitConverter295/1
  UnitConverter295/1 -> VOUTP_TurnSwSta_enum/1  "VOUTP_TurnSwSta_enum"
  VBCM_TurnSwTSetSta_enum/1 -> VBCM_TurnSwTSetSta_enum_Inproc/1  "VBCM_TurnSwTSetSta_enum"
  VBCM_TurnSwTSetSta_enum_Inproc/1 -> UnitConverter296/1
  UnitConverter296/1 -> VOUTP_TurnSwTSetSta_enum/1  "VOUTP_TurnSwTSetSta_enum"
  VBCM_SPTGENFun_flg/1 -> VBCM_SPTGENFun_flg_Inproc/1  "VBCM_SPTGENFun_flg"
  VBCM_SPTGENFun_flg_Inproc/1 -> UnitConverter297/1
  UnitConverter297/1 -> VOUTP_SPTGENFun_flg/1  "VOUTP_SPTGENFun_flg"
  VBCM_SPTGENFunMem_enum/1 -> VBCM_SPTGENFunMem_enum_Inproc/1  "VBCM_SPTGENFunMem_enum"
  VBCM_SPTGENFunMem_enum_Inproc/1 -> UnitConverter298/1
  UnitConverter298/1 -> VOUTP_SPTGENFunMem_enum/1  "VOUTP_SPTGENFunMem_enum"
  VBCM_OutMode_enum/1 -> VBCM_OutMode_enum_Inproc/1  "VBCM_OutMode_enum"
  VBCM_OutMode_enum_Inproc/1 -> UnitConverter299/1
  UnitConverter299/1 -> VOUTP_OutMode_enum/1  "VOUTP_OutMode_enum"
  VBCM_TurnSwTimeSetSta123_enum/1 -> VBCM_TurnSwTimeSetSta123_enum_Inproc/1  "VBCM_TurnSwTimeSetSta123_enum"
  VBCM_TurnSwTimeSetSta123_enum_Inproc/1 -> UnitConverter300/1
  UnitConverter300/1 -> VOUTP_TurnSwTimeSetSta123_enum/1  "VOUTP_TurnSwTimeSetSta123_enum"
  VBCM_TurnSwTimeSetSta457_enum/1 -> VBCM_TurnSwTimeSetSta457_enum_Inproc/1  "VBCM_TurnSwTimeSetSta457_enum"
  VBCM_TurnSwTimeSetSta457_enum_Inproc/1 -> UnitConverter301/1
  UnitConverter301/1 -> VOUTP_TurnSwTimeSetSta457_enum/1  "VOUTP_TurnSwTimeSetSta457_enum"
  VBCM_FDLHandleLampCmd_flg/1 -> VBCM_FDLHandleLampCmd_flg_Inproc/1  "VBCM_FDLHandleLampCmd_flg"
  VBCM_FDLHandleLampCmd_flg_Inproc/1 -> UnitConverter302/1
  UnitConverter302/1 -> VOUTP_FDLHandleLampCmd_flg/1  "VOUTP_FDLHandleLampCmd_flg"
  VBCM_FDRHandleLampCmd_flg/1 -> VBCM_FDRHandleLampCmd_flg_Inproc/1  "VBCM_FDRHandleLampCmd_flg"
  VBCM_FDRHandleLampCmd_flg_Inproc/1 -> UnitConverter303/1
  UnitConverter303/1 -> VOUTP_FDRHandleLampCmd_flg/1  "VOUTP_FDRHandleLampCmd_flg"
  VBCM_FDHandleCmd_enum/1 -> VBCM_FDHandleCmd_enum_Inproc/1  "VBCM_FDHandleCmd_enum"
  VBCM_FDHandleCmd_enum_Inproc/1 -> UnitConverter304/1
  UnitConverter304/1 -> VOUTP_FDHandleCmd_enum/1  "VOUTP_FDHandleCmd_enum"
  VBCM_HBeamADB_flg/1 -> VBCM_HBeamADB_flg_Inproc/1  "VBCM_HBeamADB_flg"
  VBCM_HBeamADB_flg_Inproc/1 -> UnitConverter305/1
  UnitConverter305/1 -> VOUTP_HBeamADB_flg/1  "VOUTP_HBeamADB_flg"
  VBCM_WalkInUnLkENMem_enum/1 -> VBCM_WalkInUnLkENMem_enum_Inproc/1  "VBCM_WalkInUnLkENMem_enum"
  VBCM_WalkInUnLkENMem_enum_Inproc/1 -> UnitConverter306/1
  UnitConverter306/1 -> VOUTP_WalkInUnLkENMem_enum/1  "VOUTP_WalkInUnLkENMem_enum"
  VBCM_WalkOutLkENMem_enum/1 -> VBCM_WalkOutLkENMem_enum_Inproc/1  "VBCM_WalkOutLkENMem_enum"
  VBCM_WalkOutLkENMem_enum_Inproc/1 -> UnitConverter307/1
  UnitConverter307/1 -> VOUTP_WalkOutLkENMem_enum/1  "VOUTP_WalkOutLkENMem_enum"
  VBCM_RmLpModeENMem_enum/1 -> VBCM_RmLpModeENMem_enum_Inproc/1  "VBCM_RmLpModeENMem_enum"
  VBCM_RmLpModeENMem_enum_Inproc/1 -> UnitConverter308/1
  UnitConverter308/1 -> VOUTP_RmLpModeENMem_enum/1  "VOUTP_RmLpModeENMem_enum"
  VBCM_LockSettingStaMem_enum/1 -> VBCM_LockSettingStaMem_enum_Inproc/1  "VBCM_LockSettingStaMem_enum"
  VBCM_LockSettingStaMem_enum_Inproc/1 -> UnitConverter309/1
  UnitConverter309/1 -> VOUTP_LockSettingStaMem_enum/1  "VOUTP_LockSettingStaMem_enum"
  VBCM_FollowMeENMem_enum/1 -> VBCM_FollowMeENMem_enum_Inproc/1  "VBCM_FollowMeENMem_enum"
  VBCM_FollowMeENMem_enum_Inproc/1 -> UnitConverter310/1
  UnitConverter310/1 -> VOUTP_FollowMeENMem_enum/1  "VOUTP_FollowMeENMem_enum"
  VBCM_WalkInUnLkENFunSta_flg/1 -> VBCM_WalkInUnLkENFunSta_flg_Inproc/1  "VBCM_WalkInUnLkENFunSta_flg"
  VBCM_WalkInUnLkENFunSta_flg_Inproc/1 -> UnitConverter311/1
  UnitConverter311/1 -> VOUTP_WalkInUnLkENFunSta_flg/1  "VOUTP_WalkInUnLkENFunSta_flg"
  VBCM_WalkOutLkENFunSta_flg/1 -> VBCM_WalkOutLkENFunSta_flg_Inproc/1  "VBCM_WalkOutLkENFunSta_flg"
  VBCM_WalkOutLkENFunSta_flg_Inproc/1 -> UnitConverter312/1
  UnitConverter312/1 -> VOUTP_WalkOutLkENFunSta_flg/1  "VOUTP_WalkOutLkENFunSta_flg"
  VBCM_RmLpModeENFunSta_flg/1 -> VBCM_RmLpModeENFunSta_flg_Inproc/1  "VBCM_RmLpModeENFunSta_flg"
  VBCM_RmLpModeENFunSta_flg_Inproc/1 -> UnitConverter313/1
  UnitConverter313/1 -> VOUTP_RmLpModeENFunSta_flg/1  "VOUTP_RmLpModeENFunSta_flg"
  VBCM_FollowMeENFunSta_flg/1 -> VBCM_FollowMeENFunSta_flg_Inproc/1  "VBCM_FollowMeENFunSta_flg"
  VBCM_FollowMeENFunSta_flg_Inproc/1 -> UnitConverter314/1
  UnitConverter314/1 -> VOUTP_FollowMeENFunSta_flg/1  "VOUTP_FollowMeENFunSta_flg"
  VBCM_HoodRelCmd_flg/1 -> VBCM_HoodRelCmd_flg_Inproc/1  "VBCM_HoodRelCmd_flg"
  VBCM_HoodRelCmd_flg_Inproc/1 -> UnitConverter315/1
  UnitConverter315/1 -> VOUTP_HoodRelCmd_flg/1  "VOUTP_HoodRelCmd_flg"
  VBCM_WelcomeLight_enum/1 -> VBCM_WelcomeLight_enum_Inproc/1  "VBCM_WelcomeLight_enum"
  VBCM_WelcomeLight_enum_Inproc/1 -> UnitConverter316/1
  UnitConverter316/1 -> VOUTP_WelcomeLight_enum/1  "VOUTP_WelcomeLight_enum"
  VBCM_PTGOpenHeightSta_enum/1 -> VBCM_PTGOpenHeightSta_enum_Inproc/1  "VBCM_PTGOpenHeightSta_enum"
  VBCM_PTGOpenHeightSta_enum_Inproc/1 -> UnitConverter317/1
  UnitConverter317/1 -> VOUTP_PTGOpenHeightSta_enum/1  "VOUTP_PTGOpenHeightSta_enum"
  VBCM_UserHeightSet_cnt/1 -> VBCM_UserHeightSet_cnt_Inproc/1  "VBCM_UserHeightSet_cnt"
  VBCM_UserHeightSet_cnt_Inproc/1 -> UnitConverter318/1
  UnitConverter318/1 -> VOUTP_UserHeightSet_cnt/1  "VOUTP_UserHeightSet_cnt"
  VBCM_PTGUserHeight1_cnt/1 -> VBCM_PTGUserHeight1_cnt_Inproc/1  "VBCM_PTGUserHeight1_cnt"
  VBCM_PTGUserHeight1_cnt_Inproc/1 -> UnitConverter319/1
  UnitConverter319/1 -> VOUTP_PTGUserHeight1_cnt/1  "VOUTP_PTGUserHeight1_cnt"
  VBCM_PTGUserHeight2_cnt/1 -> VBCM_PTGUserHeight2_cnt_Inproc/1  "VBCM_PTGUserHeight2_cnt"
  VBCM_PTGUserHeight2_cnt_Inproc/1 -> UnitConverter320/1
  UnitConverter320/1 -> VOUTP_PTGUserHeight2_cnt/1  "VOUTP_PTGUserHeight2_cnt"
  VBCM_PTGUserHeight3_cnt/1 -> VBCM_PTGUserHeight3_cnt_Inproc/1  "VBCM_PTGUserHeight3_cnt"
  VBCM_PTGUserHeight3_cnt_Inproc/1 -> UnitConverter321/1
  UnitConverter321/1 -> VOUTP_PTGUserHeight3_cnt/1  "VOUTP_PTGUserHeight3_cnt"
  VBCM_PTGUserHeight4_cnt/1 -> VBCM_PTGUserHeight4_cnt_Inproc/1  "VBCM_PTGUserHeight4_cnt"
  VBCM_PTGUserHeight4_cnt_Inproc/1 -> UnitConverter322/1
  UnitConverter322/1 -> VOUTP_PTGUserHeight4_cnt/1  "VOUTP_PTGUserHeight4_cnt"
  VBCM_PTGUserHeight5_cnt/1 -> VBCM_PTGUserHeight5_cnt_Inproc/1  "VBCM_PTGUserHeight5_cnt"
  VBCM_PTGUserHeight5_cnt_Inproc/1 -> UnitConverter323/1
  UnitConverter323/1 -> VOUTP_PTGUserHeight5_cnt/1  "VOUTP_PTGUserHeight5_cnt"
  VBCM_PTGUserHeight7_cnt/1 -> VBCM_PTGUserHeight7_cnt_Inproc/1  "VBCM_PTGUserHeight7_cnt"
  VBCM_PTGUserHeight7_cnt_Inproc/1 -> UnitConverter324/1
  UnitConverter324/1 -> VOUTP_PTGUserHeight7_cnt/1  "VOUTP_PTGUserHeight7_cnt"
  VBCM_PTGOpenHeight12_enum/1 -> VBCM_PTGOpenHeight12_enum_Inproc/1  "VBCM_PTGOpenHeight12_enum"
  VBCM_PTGOpenHeight12_enum_Inproc/1 -> UnitConverter325/1
  UnitConverter325/1 -> VOUTP_PTGOpenHeight12_enum/1  "VOUTP_PTGOpenHeight12_enum"
  VBCM_PTGOpenHeight34_enum/1 -> VBCM_PTGOpenHeight34_enum_Inproc/1  "VBCM_PTGOpenHeight34_enum"
  VBCM_PTGOpenHeight34_enum_Inproc/1 -> UnitConverter326/1
  UnitConverter326/1 -> VOUTP_PTGOpenHeight34_enum/1  "VOUTP_PTGOpenHeight34_enum"
  VBCM_PTGOpenHeight57_enum/1 -> VBCM_PTGOpenHeight57_enum_Inproc/1  "VBCM_PTGOpenHeight57_enum"
  VBCM_PTGOpenHeight57_enum_Inproc/1 -> UnitConverter327/1
  UnitConverter327/1 -> VOUTP_PTGOpenHeight57_enum/1  "VOUTP_PTGOpenHeight57_enum"
  VBCM_SenstivityPosnCmd_enum/1 -> VBCM_SenstivityPosnCmd_enum_Inproc/1  "VBCM_SenstivityPosnCmd_enum"
  VBCM_SenstivityPosnCmd_enum_Inproc/1 -> UnitConverter328/1
  UnitConverter328/1 -> VOUTP_SenstivityPosnCmd_enum/1  "VOUTP_SenstivityPosnCmd_enum"
  VBCM_TimeGapLevelSta_enum/1 -> VBCM_TimeGapLevelSta_enum_Inproc/1  "VBCM_TimeGapLevelSta_enum"
  VBCM_TimeGapLevelSta_enum_Inproc/1 -> UnitConverter329/1
  UnitConverter329/1 -> VOUTP_TimeGapLevelSta_enum/1  "VOUTP_TimeGapLevelSta_enum"
  VBCM_ACCLevelMem12_enum/1 -> VBCM_ACCLevelMem12_enum_Inproc/1  "VBCM_ACCLevelMem12_enum"
  VBCM_ACCLevelMem12_enum_Inproc/1 -> UnitConverter330/1
  UnitConverter330/1 -> VOUTP_ACCLevelMem12_enum/1  "VOUTP_ACCLevelMem12_enum"
  VBCM_ACCLevelMem34_enum/1 -> VBCM_ACCLevelMem34_enum_Inproc/1  "VBCM_ACCLevelMem34_enum"
  VBCM_ACCLevelMem34_enum_Inproc/1 -> UnitConverter331/1
  UnitConverter331/1 -> VOUTP_ACCLevelMem34_enum/1  "VOUTP_ACCLevelMem34_enum"
  VBCM_ACCLevelMem57_enum/1 -> VBCM_ACCLevelMem57_enum_Inproc/1  "VBCM_ACCLevelMem57_enum"
  VBCM_ACCLevelMem57_enum_Inproc/1 -> UnitConverter332/1
  UnitConverter332/1 -> VOUTP_ACCLevelMem57_enum/1  "VOUTP_ACCLevelMem57_enum"
  VBCM_LRightStaCmd_flg/1 -> VBCM_LRightStaCmd_flg_Inproc/1  "VBCM_LRightStaCmd_flg"
  VBCM_LRightStaCmd_flg_Inproc/1 -> UnitConverter333/1
  UnitConverter333/1 -> VOUTP_LRightStaCmd_flg/1  "VOUTP_LRightStaCmd_flg"
  VBCM_LLeftStaCmd_flg/1 -> VBCM_LLeftStaCmd_flg_Inproc/1  "VBCM_LLeftStaCmd_flg"
  VBCM_LLeftStaCmd_flg_Inproc/1 -> UnitConverter334/1
  UnitConverter334/1 -> VOUTP_LLeftStaCmd_flg/1  "VOUTP_LLeftStaCmd_flg"
  VBCM_AutoLockSta_flg/1 -> VBCM_AutoLockSta_flg_Inproc/1  "VBCM_AutoLockSta_flg"
  VBCM_AutoLockSta_flg_Inproc/1 -> UnitConverter335/1
  UnitConverter335/1 -> VOUTP_AutoLockSta_flg/1  "VOUTP_AutoLockSta_flg"
  VBCM_AutoLockMem_enum/1 -> VBCM_AutoLockMem_enum_Inproc/1  "VBCM_AutoLockMem_enum"
  VBCM_AutoLockMem_enum_Inproc/1 -> UnitConverter336/1
  UnitConverter336/1 -> VOUTP_AutoLockMem_enum/1  "VOUTP_AutoLockMem_enum"
  VBCM_AutoUnlockSta_flg/1 -> VBCM_AutoUnlockSta_flg_Inproc/1  "VBCM_AutoUnlockSta_flg"
  VBCM_AutoUnlockSta_flg_Inproc/1 -> UnitConverter337/1
  UnitConverter337/1 -> VOUTP_AutoUnlockSta_flg/1  "VOUTP_AutoUnlockSta_flg"
  VBCM_AutoUnlockMem_enum/1 -> VBCM_AutoUnlockMem_enum_Inproc/1  "VBCM_AutoUnlockMem_enum"
  VBCM_AutoUnlockMem_enum_Inproc/1 -> UnitConverter338/1
  UnitConverter338/1 -> VOUTP_AutoUnlockMem_enum/1  "VOUTP_AutoUnlockMem_enum"
  VBCM_HMIKey1FuncSta_enum/1 -> VBCM_HMIKey1FuncSta_enum_Inproc/1  "VBCM_HMIKey1FuncSta_enum"
  VBCM_HMIKey1FuncSta_enum_Inproc/1 -> UnitConverter339/1
  UnitConverter339/1 -> VOUTP_HMIKey1FuncSta_enum/1  "VOUTP_HMIKey1FuncSta_enum"
  VBCM_HMIKey2FuncSta_enum/1 -> VBCM_HMIKey2FuncSta_enum_Inproc/1  "VBCM_HMIKey2FuncSta_enum"
  VBCM_HMIKey2FuncSta_enum_Inproc/1 -> UnitConverter340/1
  UnitConverter340/1 -> VOUTP_HMIKey2FuncSta_enum/1  "VOUTP_HMIKey2FuncSta_enum"
  VBCM_HMIKey3FuncSta_enum/1 -> VBCM_HMIKey3FuncSta_enum_Inproc/1  "VBCM_HMIKey3FuncSta_enum"
  VBCM_HMIKey3FuncSta_enum_Inproc/1 -> UnitConverter341/1
  UnitConverter341/1 -> VOUTP_HMIKey3FuncSta_enum/1  "VOUTP_HMIKey3FuncSta_enum"
  VBCM_HMIKey4FuncSta_enum/1 -> VBCM_HMIKey4FuncSta_enum_Inproc/1  "VBCM_HMIKey4FuncSta_enum"
  VBCM_HMIKey4FuncSta_enum_Inproc/1 -> UnitConverter342/1
  UnitConverter342/1 -> VOUTP_HMIKey4FuncSta_enum/1  "VOUTP_HMIKey4FuncSta_enum"
  VBCM_HMIKey5FuncSta_enum/1 -> VBCM_HMIKey5FuncSta_enum_Inproc/1  "VBCM_HMIKey5FuncSta_enum"
  VBCM_HMIKey5FuncSta_enum_Inproc/1 -> UnitConverter343/1
  UnitConverter343/1 -> VOUTP_HMIKey5FuncSta_enum/1  "VOUTP_HMIKey5FuncSta_enum"
  VBCM_HMIKey6FuncSta_enum/1 -> VBCM_HMIKey6FuncSta_enum_Inproc/1  "VBCM_HMIKey6FuncSta_enum"
  VBCM_HMIKey6FuncSta_enum_Inproc/1 -> UnitConverter344/1
  UnitConverter344/1 -> VOUTP_HMIKey6FuncSta_enum/1  "VOUTP_HMIKey6FuncSta_enum"
  VBCM_HMIKey7FuncSta_enum/1 -> VBCM_HMIKey7FuncSta_enum_Inproc/1  "VBCM_HMIKey7FuncSta_enum"
  VBCM_HMIKey7FuncSta_enum_Inproc/1 -> UnitConverter345/1
  UnitConverter345/1 -> VOUTP_HMIKey7FuncSta_enum/1  "VOUTP_HMIKey7FuncSta_enum"
  VBCM_HMIKey8FuncSta_enum/1 -> VBCM_HMIKey8FuncSta_enum_Inproc/1  "VBCM_HMIKey8FuncSta_enum"
  VBCM_HMIKey8FuncSta_enum_Inproc/1 -> UnitConverter346/1
  UnitConverter346/1 -> VOUTP_HMIKey8FuncSta_enum/1  "VOUTP_HMIKey8FuncSta_enum"
  VBCM_AutoWipHSpdENSta_flg/1 -> VBCM_AutoWipHSpdENSta_flg_Inproc/1  "VBCM_AutoWipHSpdENSta_flg"
  VBCM_AutoWipHSpdENSta_flg_Inproc/1 -> UnitConverter347/1
  UnitConverter347/1 -> VOUTP_AutoWipHSpdENSta_flg/1  "VOUTP_AutoWipHSpdENSta_flg"
  VBCM_DrvWdwReqAP_enum/1 -> VBCM_DrvWdwReqAP_enum_Inproc/1  "VBCM_DrvWdwReqAP_enum"
  VBCM_DrvWdwReqAP_enum_Inproc/1 -> UnitConverter348/1
  UnitConverter348/1 -> VOUTP_DrvWdwReqAP_enum/1  "VOUTP_DrvWdwReqAP_enum"
  VBCM_PasWdwReqAP_enum/1 -> VBCM_PasWdwReqAP_enum_Inproc/1  "VBCM_PasWdwReqAP_enum"
  VBCM_PasWdwReqAP_enum_Inproc/1 -> UnitConverter349/1
  UnitConverter349/1 -> VOUTP_PasWdwReqAP_enum/1  "VOUTP_PasWdwReqAP_enum"
  VBCM_DrRWdwReqAP_enum/1 -> VBCM_DrRWdwReqAP_enum_Inproc/1  "VBCM_DrRWdwReqAP_enum"
  VBCM_DrRWdwReqAP_enum_Inproc/1 -> UnitConverter350/1
  UnitConverter350/1 -> VOUTP_DrRWdwReqAP_enum/1  "VOUTP_DrRWdwReqAP_enum"
  VBCM_PsRWdwReqAP_enum/1 -> VBCM_PsRWdwReqAP_enum_Inproc/1  "VBCM_PsRWdwReqAP_enum"
  VBCM_PsRWdwReqAP_enum_Inproc/1 -> UnitConverter351/1
  UnitConverter351/1 -> VOUTP_PsRWdwReqAP_enum/1  "VOUTP_PsRWdwReqAP_enum"
  VBCM_CLWinLockDrSta_flg/1 -> VBCM_CLWinLockDrSta_flg_Inproc/1  "VBCM_CLWinLockDrSta_flg"
  VBCM_CLWinLockDrSta_flg_Inproc/1 -> UnitConverter352/1
  UnitConverter352/1 -> VOUTP_CLWinLockDrSta_flg/1  "VOUTP_CLWinLockDrSta_flg"
  VBCM_CLWinLockDrStaMem_enum/1 -> VBCM_CLWinLockDrStaMem_enum_Inproc/1  "VBCM_CLWinLockDrStaMem_enum"
  VBCM_CLWinLockDrStaMem_enum_Inproc/1 -> UnitConverter353/1
  UnitConverter353/1 -> VOUTP_CLWinLockDrStaMem_enum/1  "VOUTP_CLWinLockDrStaMem_enum"
  VBCM_WinLFOpenedSta_pct/1 -> VBCM_WinLFOpenedSta_pct_Inproc/1  "VBCM_WinLFOpenedSta_pct"
  VBCM_WinLFOpenedSta_pct_Inproc/1 -> UnitConverter354/1
  UnitConverter354/1 -> VOUTP_WinLFOpenedSta_pct/1  "VOUTP_WinLFOpenedSta_pct"
  VBCM_WinRFOpenedSta_pct/1 -> VBCM_WinRFOpenedSta_pct_Inproc/1  "VBCM_WinRFOpenedSta_pct"
  VBCM_WinRFOpenedSta_pct_Inproc/1 -> UnitConverter355/1
  UnitConverter355/1 -> VOUTP_WinRFOpenedSta_pct/1  "VOUTP_WinRFOpenedSta_pct"
  VBCM_WinLROpenedSta_pct/1 -> VBCM_WinLROpenedSta_pct_Inproc/1  "VBCM_WinLROpenedSta_pct"
  VBCM_WinLROpenedSta_pct_Inproc/1 -> UnitConverter356/1
  UnitConverter356/1 -> VOUTP_WinLROpenedSta_pct/1  "VOUTP_WinLROpenedSta_pct"
  VBCM_WinRROpenedSta_pct/1 -> VBCM_WinRROpenedSta_pct_Inproc/1  "VBCM_WinRROpenedSta_pct"
  VBCM_WinRROpenedSta_pct_Inproc/1 -> UnitConverter357/1
  UnitConverter357/1 -> VOUTP_WinRROpenedSta_pct/1  "VOUTP_WinRROpenedSta_pct"
  VBCM_FoxPiSwitchSta_enum/1 -> VBCM_FoxPiSwitchSta_enum_Inproc/1  "VBCM_FoxPiSwitchSta_enum"
  VBCM_FoxPiSwitchSta_enum_Inproc/1 -> UnitConverter358/1
  UnitConverter358/1 -> VOUTP_FoxPiSwitchSta_enum/1  "VOUTP_FoxPiSwitchSta_enum"
  VBCM_FoxPiLampSta_enum/1 -> VBCM_FoxPiLampSta_enum_Inproc/1  "VBCM_FoxPiLampSta_enum"
  VBCM_FoxPiLampSta_enum_Inproc/1 -> UnitConverter359/1
  UnitConverter359/1 -> VOUTP_FoxPiLampSta_enum/1  "VOUTP_FoxPiLampSta_enum"
  VDDM_C3BMS6RCDTC_raw32/1 -> VDDM_C3BMS6RCDTC_raw32_Inproc/1  "VDDM_C3BMS6RCDTC_raw32"
  VDDM_C3BMS6RCDTC_raw32_Inproc/1 -> UnitConverter360/1
  UnitConverter360/1 -> VOUTP_C3BMS6RCDTC_raw32/1  "VOUTP_C3BMS6RCDTC_raw32"
  VDDM_C3BMS6CSDTC_raw32/1 -> VDDM_C3BMS6CSDTC_raw32_Inproc/1  "VDDM_C3BMS6CSDTC_raw32"
  VDDM_C3BMS6CSDTC_raw32_Inproc/1 -> UnitConverter361/1
  UnitConverter361/1 -> VOUTP_C3BMS6CSDTC_raw32/1  "VOUTP_C3BMS6CSDTC_raw32"
  VDDM_C3BMS6LCDTC_raw32/1 -> VDDM_C3BMS6LCDTC_raw32_Inproc/1  "VDDM_C3BMS6LCDTC_raw32"
  VDDM_C3BMS6LCDTC_raw32_Inproc/1 -> UnitConverter362/1
  UnitConverter362/1 -> VOUTP_C3BMS6LCDTC_raw32/1  "VOUTP_C3BMS6LCDTC_raw32"
  VDDM_C3BMS1RCDTC_raw32/1 -> VDDM_C3BMS1RCDTC_raw32_Inproc/1  "VDDM_C3BMS1RCDTC_raw32"
  VDDM_C3BMS1RCDTC_raw32_Inproc/1 -> UnitConverter363/1
  UnitConverter363/1 -> VOUTP_C3BMS1RCDTC_raw32/1  "VOUTP_C3BMS1RCDTC_raw32"
  VDDM_C3BMS1CSDTC_raw32/1 -> VDDM_C3BMS1CSDTC_raw32_Inproc/1  "VDDM_C3BMS1CSDTC_raw32"
  VDDM_C3BMS1CSDTC_raw32_Inproc/1 -> UnitConverter364/1
  UnitConverter364/1 -> VOUTP_C3BMS1CSDTC_raw32/1  "VOUTP_C3BMS1CSDTC_raw32"
  VDDM_C3BMS1LCDTC_raw32/1 -> VDDM_C3BMS1LCDTC_raw32_Inproc/1  "VDDM_C3BMS1LCDTC_raw32"
  VDDM_C3BMS1LCDTC_raw32_Inproc/1 -> UnitConverter365/1
  UnitConverter365/1 -> VOUTP_C3BMS1LCDTC_raw32/1  "VOUTP_C3BMS1LCDTC_raw32"
  VDDM_C3CCU1RCDTC_raw32/1 -> VDDM_C3CCU1RCDTC_raw32_Inproc/1  "VDDM_C3CCU1RCDTC_raw32"
  VDDM_C3CCU1RCDTC_raw32_Inproc/1 -> UnitConverter366/1
  UnitConverter366/1 -> VOUTP_C3CCU1RCDTC_raw32/1  "VOUTP_C3CCU1RCDTC_raw32"
  VDDM_C3CCU1CSDTC_raw32/1 -> VDDM_C3CCU1CSDTC_raw32_Inproc/1  "VDDM_C3CCU1CSDTC_raw32"
  VDDM_C3CCU1CSDTC_raw32_Inproc/1 -> UnitConverter367/1
  UnitConverter367/1 -> VOUTP_C3CCU1CSDTC_raw32/1  "VOUTP_C3CCU1CSDTC_raw32"
  VDDM_C3CCU1LCDTC_raw32/1 -> VDDM_C3CCU1LCDTC_raw32_Inproc/1  "VDDM_C3CCU1LCDTC_raw32"
  VDDM_C3CCU1LCDTC_raw32_Inproc/1 -> UnitConverter368/1
  UnitConverter368/1 -> VOUTP_C3CCU1LCDTC_raw32/1  "VOUTP_C3CCU1LCDTC_raw32"
  VDDM_C3CCU2RCDTC_raw32/1 -> VDDM_C3CCU2RCDTC_raw32_Inproc/1  "VDDM_C3CCU2RCDTC_raw32"
  VDDM_C3CCU2RCDTC_raw32_Inproc/1 -> UnitConverter369/1
  UnitConverter369/1 -> VOUTP_C3CCU2RCDTC_raw32/1  "VOUTP_C3CCU2RCDTC_raw32"
  VDDM_C3CCU2CSDTC_raw32/1 -> VDDM_C3CCU2CSDTC_raw32_Inproc/1  "VDDM_C3CCU2CSDTC_raw32"
  VDDM_C3CCU2CSDTC_raw32_Inproc/1 -> UnitConverter370/1
  UnitConverter370/1 -> VOUTP_C3CCU2CSDTC_raw32/1  "VOUTP_C3CCU2CSDTC_raw32"
  VDDM_C3CCU2LCDTC_raw32/1 -> VDDM_C3CCU2LCDTC_raw32_Inproc/1  "VDDM_C3CCU2LCDTC_raw32"
  VDDM_C3CCU2LCDTC_raw32_Inproc/1 -> UnitConverter371/1
  UnitConverter371/1 -> VOUTP_C3CCU2LCDTC_raw32/1  "VOUTP_C3CCU2LCDTC_raw32"
  VDDM_C1ABM1RCDTC_raw32/1 -> VDDM_C1ABM1RCDTC_raw32_Inproc/1  "VDDM_C1ABM1RCDTC_raw32"
  VDDM_C1ABM1RCDTC_raw32_Inproc/1 -> UnitConverter372/1
  UnitConverter372/1 -> VOUTP_C1ABM1RCDTC_raw32/1  "VOUTP_C1ABM1RCDTC_raw32"
  VDDM_C1ABM1CSDTC_raw32/1 -> VDDM_C1ABM1CSDTC_raw32_Inproc/1  "VDDM_C1ABM1CSDTC_raw32"
  VDDM_C1ABM1CSDTC_raw32_Inproc/1 -> UnitConverter373/1
  UnitConverter373/1 -> VOUTP_C1ABM1CSDTC_raw32/1  "VOUTP_C1ABM1CSDTC_raw32"
  VDDM_C1ABM1LCDTC_raw32/1 -> VDDM_C1ABM1LCDTC_raw32_Inproc/1  "VDDM_C1ABM1LCDTC_raw32"
  VDDM_C1ABM1LCDTC_raw32_Inproc/1 -> UnitConverter374/1
  UnitConverter374/1 -> VOUTP_C1ABM1LCDTC_raw32/1  "VOUTP_C1ABM1LCDTC_raw32"
  VDDM_Lv1ErrDTC_raw32/1 -> VDDM_Lv1ErrDTC_raw32_Inproc/1  "VDDM_Lv1ErrDTC_raw32"
  VDDM_Lv1ErrDTC_raw32_Inproc/1 -> UnitConverter375/1
  UnitConverter375/1 -> VOUTP_Lv1ErrDTC_raw32/1  "VOUTP_Lv1ErrDTC_raw32"
  VDDM_Lv2ErrDTC_raw32/1 -> VDDM_Lv2ErrDTC_raw32_Inproc/1  "VDDM_Lv2ErrDTC_raw32"
  VDDM_Lv2ErrDTC_raw32_Inproc/1 -> UnitConverter376/1
  UnitConverter376/1 -> VOUTP_Lv2ErrDTC_raw32/1  "VOUTP_Lv2ErrDTC_raw32"
  VDDM_Lv3ErrDTC_raw32/1 -> VDDM_Lv3ErrDTC_raw32_Inproc/1  "VDDM_Lv3ErrDTC_raw32"
  VDDM_Lv3ErrDTC_raw32_Inproc/1 -> UnitConverter377/1
  UnitConverter377/1 -> VOUTP_Lv3ErrDTC_raw32/1  "VOUTP_Lv3ErrDTC_raw32"
  VDDM_Lv4ErrDTC_raw32/1 -> VDDM_Lv4ErrDTC_raw32_Inproc/1  "VDDM_Lv4ErrDTC_raw32"
  VDDM_Lv4ErrDTC_raw32_Inproc/1 -> UnitConverter378/1
  UnitConverter378/1 -> VOUTP_Lv4ErrDTC_raw32/1  "VOUTP_Lv4ErrDTC_raw32"
  VDDM_BrkSWErrDTC_raw32/1 -> VDDM_BrkSWErrDTC_raw32_Inproc/1  "VDDM_BrkSWErrDTC_raw32"
  VDDM_BrkSWErrDTC_raw32_Inproc/1 -> UnitConverter379/1
  UnitConverter379/1 -> VOUTP_BrkSWErrDTC_raw32/1  "VOUTP_BrkSWErrDTC_raw32"
  VDDM_BrkSWNoBacDTC_raw32/1 -> VDDM_BrkSWNoBacDTC_raw32_Inproc/1  "VDDM_BrkSWNoBacDTC_raw32"
  VDDM_BrkSWNoBacDTC_raw32_Inproc/1 -> UnitConverter380/1
  UnitConverter380/1 -> VOUTP_BrkSWNoBacDTC_raw32/1  "VOUTP_BrkSWNoBacDTC_raw32"
  VDDM_KeyAuthDTC_raw32/1 -> VDDM_KeyAuthDTC_raw32_Inproc/1  "VDDM_KeyAuthDTC_raw32"
  VDDM_KeyAuthDTC_raw32_Inproc/1 -> UnitConverter381/1
  UnitConverter381/1 -> VOUTP_KeyAuthDTC_raw32/1  "VOUTP_KeyAuthDTC_raw32"
  VDDM_ONtoRdyDTC_raw32/1 -> VDDM_ONtoRdyDTC_raw32_Inproc/1  "VDDM_ONtoRdyDTC_raw32"
  VDDM_ONtoRdyDTC_raw32_Inproc/1 -> UnitConverter382/1
  UnitConverter382/1 -> VOUTP_ONtoRdyDTC_raw32/1  "VOUTP_ONtoRdyDTC_raw32"
  VDDM_HVB4PreDTC_raw32/1 -> VDDM_HVB4PreDTC_raw32_Inproc/1  "VDDM_HVB4PreDTC_raw32"
  VDDM_HVB4PreDTC_raw32_Inproc/1 -> UnitConverter383/1
  UnitConverter383/1 -> VOUTP_HVB4PreDTC_raw32/1  "VOUTP_HVB4PreDTC_raw32"
  VDDM_MCU4PreDTC_raw32/1 -> VDDM_MCU4PreDTC_raw32_Inproc/1  "VDDM_MCU4PreDTC_raw32"
  VDDM_MCU4PreDTC_raw32_Inproc/1 -> UnitConverter384/1
  UnitConverter384/1 -> VOUTP_MCU4PreDTC_raw32/1  "VOUTP_MCU4PreDTC_raw32"
  VDDM_DCDC4PreDTC_raw32/1 -> VDDM_DCDC4PreDTC_raw32_Inproc/1  "VDDM_DCDC4PreDTC_raw32"
  VDDM_DCDC4PreDTC_raw32_Inproc/1 -> UnitConverter385/1
  UnitConverter385/1 -> VOUTP_DCDC4PreDTC_raw32/1  "VOUTP_DCDC4PreDTC_raw32"
  VDDM_HVRlyCloDTC_raw32/1 -> VDDM_HVRlyCloDTC_raw32_Inproc/1  "VDDM_HVRlyCloDTC_raw32"
  VDDM_HVRlyCloDTC_raw32_Inproc/1 -> UnitConverter386/1
  UnitConverter386/1 -> VOUTP_HVRlyCloDTC_raw32/1  "VOUTP_HVRlyCloDTC_raw32"
  VDDM_BMSRdyDTC_raw32/1 -> VDDM_BMSRdyDTC_raw32_Inproc/1  "VDDM_BMSRdyDTC_raw32"
  VDDM_BMSRdyDTC_raw32_Inproc/1 -> UnitConverter387/1
  UnitConverter387/1 -> VOUTP_BMSRdyDTC_raw32/1  "VOUTP_BMSRdyDTC_raw32"
  VDDM_DCDCEnaDTC_raw32/1 -> VDDM_DCDCEnaDTC_raw32_Inproc/1  "VDDM_DCDCEnaDTC_raw32"
  VDDM_DCDCEnaDTC_raw32_Inproc/1 -> UnitConverter388/1
  UnitConverter388/1 -> VOUTP_DCDCEnaDTC_raw32/1  "VOUTP_DCDCEnaDTC_raw32"
  VDDM_HiLvSaChkDTC_raw32/1 -> VDDM_HiLvSaChkDTC_raw32_Inproc/1  "VDDM_HiLvSaChkDTC_raw32"
  VDDM_HiLvSaChkDTC_raw32_Inproc/1 -> UnitConverter389/1
  UnitConverter389/1 -> VOUTP_HiLvSaChkDTC_raw32/1  "VOUTP_HiLvSaChkDTC_raw32"
  VDDM_MidLvSaChkDTC_raw32/1 -> VDDM_MidLvSaChkDTC_raw32_Inproc/1  "VDDM_MidLvSaChkDTC_raw32"
  VDDM_MidLvSaChkDTC_raw32_Inproc/1 -> UnitConverter390/1
  UnitConverter390/1 -> VOUTP_MidLvSaChkDTC_raw32/1  "VOUTP_MidLvSaChkDTC_raw32"
  VDDM_MCUDisDTC_raw32/1 -> VDDM_MCUDisDTC_raw32_Inproc/1  "VDDM_MCUDisDTC_raw32"
  VDDM_MCUDisDTC_raw32_Inproc/1 -> UnitConverter391/1
  UnitConverter391/1 -> VOUTP_MCUDisDTC_raw32/1  "VOUTP_MCUDisDTC_raw32"
  VDDM_DCDCDisDTC_raw32/1 -> VDDM_DCDCDisDTC_raw32_Inproc/1  "VDDM_DCDCDisDTC_raw32"
  VDDM_DCDCDisDTC_raw32_Inproc/1 -> UnitConverter392/1
  UnitConverter392/1 -> VOUTP_DCDCDisDTC_raw32/1  "VOUTP_DCDCDisDTC_raw32"
  VDDM_HVRlyOpDTC_raw32/1 -> VDDM_HVRlyOpDTC_raw32_Inproc/1  "VDDM_HVRlyOpDTC_raw32"
  VDDM_HVRlyOpDTC_raw32_Inproc/1 -> UnitConverter393/1
  UnitConverter393/1 -> VOUTP_HVRlyOpDTC_raw32/1  "VOUTP_HVRlyOpDTC_raw32"
  VDDM_MCUActDTC_raw32/1 -> VDDM_MCUActDTC_raw32_Inproc/1  "VDDM_MCUActDTC_raw32"
  VDDM_MCUActDTC_raw32_Inproc/1 -> UnitConverter394/1
  UnitConverter394/1 -> VOUTP_MCUActDTC_raw32/1  "VOUTP_MCUActDTC_raw32"
  VDDM_OBC4PreDTC_raw32/1 -> VDDM_OBC4PreDTC_raw32_Inproc/1  "VDDM_OBC4PreDTC_raw32"
  VDDM_OBC4PreDTC_raw32_Inproc/1 -> UnitConverter395/1
  UnitConverter395/1 -> VOUTP_OBC4PreDTC_raw32/1  "VOUTP_OBC4PreDTC_raw32"
  VDDM_IniLVLoDTC_raw32/1 -> VDDM_IniLVLoDTC_raw32_Inproc/1  "VDDM_IniLVLoDTC_raw32"
  VDDM_IniLVLoDTC_raw32_Inproc/1 -> UnitConverter396/1
  UnitConverter396/1 -> VOUTP_IniLVLoDTC_raw32/1  "VOUTP_IniLVLoDTC_raw32"
  VDDM_LVSupLoDTC_raw32/1 -> VDDM_LVSupLoDTC_raw32_Inproc/1  "VDDM_LVSupLoDTC_raw32"
  VDDM_LVSupLoDTC_raw32_Inproc/1 -> UnitConverter397/1
  UnitConverter397/1 -> VOUTP_LVSupLoDTC_raw32/1  "VOUTP_LVSupLoDTC_raw32"
  VDDM_LVSupHiDTC_raw32/1 -> VDDM_LVSupHiDTC_raw32_Inproc/1  "VDDM_LVSupHiDTC_raw32"
  VDDM_LVSupHiDTC_raw32_Inproc/1 -> UnitConverter398/1
  UnitConverter398/1 -> VOUTP_LVSupHiDTC_raw32/1  "VOUTP_LVSupHiDTC_raw32"
  VDDM_DrStSWDTC_raw32/1 -> VDDM_DrStSWDTC_raw32_Inproc/1  "VDDM_DrStSWDTC_raw32"
  VDDM_DrStSWDTC_raw32_Inproc/1 -> UnitConverter399/1
  UnitConverter399/1 -> VOUTP_DrStSWDTC_raw32/1  "VOUTP_DrStSWDTC_raw32"
  VDDM_FLDoorSWDTC_raw32/1 -> VDDM_FLDoorSWDTC_raw32_Inproc/1  "VDDM_FLDoorSWDTC_raw32"
  VDDM_FLDoorSWDTC_raw32_Inproc/1 -> UnitConverter400/1
  UnitConverter400/1 -> VOUTP_FLDoorSWDTC_raw32/1  "VOUTP_FLDoorSWDTC_raw32"
  VDDM_RLDoorSWDTC_raw32/1 -> VDDM_RLDoorSWDTC_raw32_Inproc/1  "VDDM_RLDoorSWDTC_raw32"
  VDDM_RLDoorSWDTC_raw32_Inproc/1 -> UnitConverter401/1
  UnitConverter401/1 -> VOUTP_RLDoorSWDTC_raw32/1  "VOUTP_RLDoorSWDTC_raw32"
  VDDM_FRDoorSWDTC_raw32/1 -> VDDM_FRDoorSWDTC_raw32_Inproc/1  "VDDM_FRDoorSWDTC_raw32"
  VDDM_FRDoorSWDTC_raw32_Inproc/1 -> UnitConverter402/1
  UnitConverter402/1 -> VOUTP_FRDoorSWDTC_raw32/1  "VOUTP_FRDoorSWDTC_raw32"
  VDDM_RRDoorSWDTC_raw32/1 -> VDDM_RRDoorSWDTC_raw32_Inproc/1  "VDDM_RRDoorSWDTC_raw32"
  VDDM_RRDoorSWDTC_raw32_Inproc/1 -> UnitConverter403/1
  UnitConverter403/1 -> VOUTP_RRDoorSWDTC_raw32/1  "VOUTP_RRDoorSWDTC_raw32"
  VDDM_HoodSWDTC_raw32/1 -> VDDM_HoodSWDTC_raw32_Inproc/1  "VDDM_HoodSWDTC_raw32"
  VDDM_HoodSWDTC_raw32_Inproc/1 -> UnitConverter404/1
  UnitConverter404/1 -> VOUTP_HoodSWDTC_raw32/1  "VOUTP_HoodSWDTC_raw32"
  VDDM_TailgaSWDTC_raw32/1 -> VDDM_TailgaSWDTC_raw32_Inproc/1  "VDDM_TailgaSWDTC_raw32"
  VDDM_TailgaSWDTC_raw32_Inproc/1 -> UnitConverter405/1
  UnitConverter405/1 -> VOUTP_TailgaSWDTC_raw32/1  "VOUTP_TailgaSWDTC_raw32"
  VDDM_EDriveSysErrVCUErr_flg/1 -> VDDM_EDriveSysErrVCUErr_flg_Inproc/1  "VDDM_EDriveSysErrVCUErr_flg"
  VDDM_EDriveSysErrVCUErr_flg_Inproc/1 -> UnitConverter406/1
  UnitConverter406/1 -> VOUTP_EDriveSysErrVCUErr_flg/1  "VOUTP_EDriveSysErrVCUErr_flg"
  VDDM_VehMalfunLevel_enum/1 -> VDDM_VehMalfunLevel_enum_Inproc/1  "VDDM_VehMalfunLevel_enum"
  VDDM_VehMalfunLevel_enum_Inproc/1 -> UnitConverter407/1
  UnitConverter407/1 -> VOUTP_VehMalfunLevel_enum/1  "VOUTP_VehMalfunLevel_enum"
  VDDM_APS1SigOoRDTC_raw32/1 -> VDDM_APS1SigOoRDTC_raw32_Inproc/1  "VDDM_APS1SigOoRDTC_raw32"
  VDDM_APS1SigOoRDTC_raw32_Inproc/1 -> UnitConverter408/1
  UnitConverter408/1 -> VOUTP_APS1SigOoRDTC_raw32/1  "VOUTP_APS1SigOoRDTC_raw32"
  VDDM_APS2SigOoRDTC_raw32/1 -> VDDM_APS2SigOoRDTC_raw32_Inproc/1  "VDDM_APS2SigOoRDTC_raw32"
  VDDM_APS2SigOoRDTC_raw32_Inproc/1 -> UnitConverter409/1
  UnitConverter409/1 -> VOUTP_APS2SigOoRDTC_raw32/1  "VOUTP_APS2SigOoRDTC_raw32"
  VDDM_APSCorrErrDTC_raw32/1 -> VDDM_APSCorrErrDTC_raw32_Inproc/1  "VDDM_APSCorrErrDTC_raw32"
  VDDM_APSCorrErrDTC_raw32_Inproc/1 -> UnitConverter410/1
  UnitConverter410/1 -> VOUTP_APSCorrErrDTC_raw32/1  "VOUTP_APSCorrErrDTC_raw32"
  VDDM_MCUF1NoComDTC_raw32/1 -> VDDM_MCUF1NoComDTC_raw32_Inproc/1  "VDDM_MCUF1NoComDTC_raw32"
  VDDM_MCUF1NoComDTC_raw32_Inproc/1 -> UnitConverter411/1
  UnitConverter411/1 -> VOUTP_MCUF1NoComDTC_raw32/1  "VOUTP_MCUF1NoComDTC_raw32"
  VDDM_MCUR1NoComDTC_raw32/1 -> VDDM_MCUR1NoComDTC_raw32_Inproc/1  "VDDM_MCUR1NoComDTC_raw32"
  VDDM_MCUR1NoComDTC_raw32_Inproc/1 -> UnitConverter412/1
  UnitConverter412/1 -> VOUTP_MCUR1NoComDTC_raw32/1  "VOUTP_MCUR1NoComDTC_raw32"
  VDDM_Shifter1NoComDTC_raw32/1 -> VDDM_Shifter1NoComDTC_raw32_Inproc/1  "VDDM_Shifter1NoComDTC_raw32"
  VDDM_Shifter1NoComDTC_raw32_Inproc/1 -> UnitConverter413/1
  UnitConverter413/1 -> VOUTP_Shifter1NoComDTC_raw32/1  "VOUTP_Shifter1NoComDTC_raw32"
  VDDM_ESC7NoComDTC_raw32/1 -> VDDM_ESC7NoComDTC_raw32_Inproc/1  "VDDM_ESC7NoComDTC_raw32"
  VDDM_ESC7NoComDTC_raw32_Inproc/1 -> UnitConverter414/1
  UnitConverter414/1 -> VOUTP_ESC7NoComDTC_raw32/1  "VOUTP_ESC7NoComDTC_raw32"
  VDDM_ESC1NoComDTC_raw32/1 -> VDDM_ESC1NoComDTC_raw32_Inproc/1  "VDDM_ESC1NoComDTC_raw32"
  VDDM_ESC1NoComDTC_raw32_Inproc/1 -> UnitConverter415/1
  UnitConverter415/1 -> VOUTP_ESC1NoComDTC_raw32/1  "VOUTP_ESC1NoComDTC_raw32"
  VDDM_ESC5NoComDTC_raw32/1 -> VDDM_ESC5NoComDTC_raw32_Inproc/1  "VDDM_ESC5NoComDTC_raw32"
  VDDM_ESC5NoComDTC_raw32_Inproc/1 -> UnitConverter416/1
  UnitConverter416/1 -> VOUTP_ESC5NoComDTC_raw32/1  "VOUTP_ESC5NoComDTC_raw32"
  VDDM_EnterNewOperCyc_flg/1 -> VDDM_EnterNewOperCyc_flg_Inproc/1  "VDDM_EnterNewOperCyc_flg"
  VDDM_EnterNewOperCyc_flg_Inproc/1 -> UnitConverter417/1
  UnitConverter417/1 -> VOUTP_EnterNewOperCyc_flg/1  "VOUTP_EnterNewOperCyc_flg"
  VDDM_DiagHCrashDTC_raw32/1 -> VDDM_DiagHCrashDTC_raw32_Inproc/1  "VDDM_DiagHCrashDTC_raw32"
  VDDM_DiagHCrashDTC_raw32_Inproc/1 -> UnitConverter418/1
  UnitConverter418/1 -> VOUTP_DiagHCrashDTC_raw32/1  "VOUTP_DiagHCrashDTC_raw32"
  VDDM_DiagFLTSDTC_raw32/1 -> VDDM_DiagFLTSDTC_raw32_Inproc/1  "VDDM_DiagFLTSDTC_raw32"
  VDDM_DiagFLTSDTC_raw32_Inproc/1 -> UnitConverter419/1
  UnitConverter419/1 -> VOUTP_DiagFLTSDTC_raw32/1  "VOUTP_DiagFLTSDTC_raw32"
  VDDM_DiagFRTSDTC_raw32/1 -> VDDM_DiagFRTSDTC_raw32_Inproc/1  "VDDM_DiagFRTSDTC_raw32"
  VDDM_DiagFRTSDTC_raw32_Inproc/1 -> UnitConverter420/1
  UnitConverter420/1 -> VOUTP_DiagFRTSDTC_raw32/1  "VOUTP_DiagFRTSDTC_raw32"
  VDDM_DiagRLTSDTC_raw32/1 -> VDDM_DiagRLTSDTC_raw32_Inproc/1  "VDDM_DiagRLTSDTC_raw32"
  VDDM_DiagRLTSDTC_raw32_Inproc/1 -> UnitConverter421/1
  UnitConverter421/1 -> VOUTP_DiagRLTSDTC_raw32/1  "VOUTP_DiagRLTSDTC_raw32"
  VDDM_DiagRRTSDTC_raw32/1 -> VDDM_DiagRRTSDTC_raw32_Inproc/1  "VDDM_DiagRRTSDTC_raw32"
  VDDM_DiagRRTSDTC_raw32_Inproc/1 -> UnitConverter422/1
  UnitConverter422/1 -> VOUTP_DiagRRTSDTC_raw32/1  "VOUTP_DiagRRTSDTC_raw32"
  VDDM_FCLUSSDTC_raw32/1 -> VDDM_FCLUSSDTC_raw32_Inproc/1  "VDDM_FCLUSSDTC_raw32"
  VDDM_FCLUSSDTC_raw32_Inproc/1 -> UnitConverter423/1
  UnitConverter423/1 -> VOUTP_FCLUSSDTC_raw32/1  "VOUTP_FCLUSSDTC_raw32"
  VDDM_FMLUSSDTC_raw32/1 -> VDDM_FMLUSSDTC_raw32_Inproc/1  "VDDM_FMLUSSDTC_raw32"
  VDDM_FMLUSSDTC_raw32_Inproc/1 -> UnitConverter424/1
  UnitConverter424/1 -> VOUTP_FMLUSSDTC_raw32/1  "VOUTP_FMLUSSDTC_raw32"
  VDDM_FMRUSSDTC_raw32/1 -> VDDM_FMRUSSDTC_raw32_Inproc/1  "VDDM_FMRUSSDTC_raw32"
  VDDM_FMRUSSDTC_raw32_Inproc/1 -> UnitConverter425/1
  UnitConverter425/1 -> VOUTP_FMRUSSDTC_raw32/1  "VOUTP_FMRUSSDTC_raw32"
  VDDM_FCRUSSDTC_raw32/1 -> VDDM_FCRUSSDTC_raw32_Inproc/1  "VDDM_FCRUSSDTC_raw32"
  VDDM_FCRUSSDTC_raw32_Inproc/1 -> UnitConverter426/1
  UnitConverter426/1 -> VOUTP_FCRUSSDTC_raw32/1  "VOUTP_FCRUSSDTC_raw32"
  VDDM_RCLUSSDTC_raw32/1 -> VDDM_RCLUSSDTC_raw32_Inproc/1  "VDDM_RCLUSSDTC_raw32"
  VDDM_RCLUSSDTC_raw32_Inproc/1 -> UnitConverter427/1
  UnitConverter427/1 -> VOUTP_RCLUSSDTC_raw32/1  "VOUTP_RCLUSSDTC_raw32"
  VDDM_RMLUSSDTC_raw32/1 -> VDDM_RMLUSSDTC_raw32_Inproc/1  "VDDM_RMLUSSDTC_raw32"
  VDDM_RMLUSSDTC_raw32_Inproc/1 -> UnitConverter428/1
  UnitConverter428/1 -> VOUTP_RMLUSSDTC_raw32/1  "VOUTP_RMLUSSDTC_raw32"
  VDDM_RMRUSSDTC_raw32/1 -> VDDM_RMRUSSDTC_raw32_Inproc/1  "VDDM_RMRUSSDTC_raw32"
  VDDM_RMRUSSDTC_raw32_Inproc/1 -> UnitConverter429/1
  UnitConverter429/1 -> VOUTP_RMRUSSDTC_raw32/1  "VOUTP_RMRUSSDTC_raw32"
  VDDM_RCRUSSDTC_raw32/1 -> VDDM_RCRUSSDTC_raw32_Inproc/1  "VDDM_RCRUSSDTC_raw32"
  VDDM_RCRUSSDTC_raw32_Inproc/1 -> UnitConverter430/1
  UnitConverter430/1 -> VOUTP_RCRUSSDTC_raw32/1  "VOUTP_RCRUSSDTC_raw32"
  VDDM_FLLUSSDTC_raw32/1 -> VDDM_FLLUSSDTC_raw32_Inproc/1  "VDDM_FLLUSSDTC_raw32"
  VDDM_FLLUSSDTC_raw32_Inproc/1 -> UnitConverter431/1
  UnitConverter431/1 -> VOUTP_FLLUSSDTC_raw32/1  "VOUTP_FLLUSSDTC_raw32"
  VDDM_FLRUSSDTC_raw32/1 -> VDDM_FLRUSSDTC_raw32_Inproc/1  "VDDM_FLRUSSDTC_raw32"
  VDDM_FLRUSSDTC_raw32_Inproc/1 -> UnitConverter432/1
  UnitConverter432/1 -> VOUTP_FLRUSSDTC_raw32/1  "VOUTP_FLRUSSDTC_raw32"
  VDDM_RLLUSSDTC_raw32/1 -> VDDM_RLLUSSDTC_raw32_Inproc/1  "VDDM_RLLUSSDTC_raw32"
  VDDM_RLLUSSDTC_raw32_Inproc/1 -> UnitConverter433/1
  UnitConverter433/1 -> VOUTP_RLLUSSDTC_raw32/1  "VOUTP_RLLUSSDTC_raw32"
  VDDM_RLRUSSDTC_raw32/1 -> VDDM_RLRUSSDTC_raw32_Inproc/1  "VDDM_RLRUSSDTC_raw32"
  VDDM_RLRUSSDTC_raw32_Inproc/1 -> UnitConverter434/1
  UnitConverter434/1 -> VOUTP_RLRUSSDTC_raw32/1  "VOUTP_RLRUSSDTC_raw32"
  VDDM_FCM2NoComDTC_raw32/1 -> VDDM_FCM2NoComDTC_raw32_Inproc/1  "VDDM_FCM2NoComDTC_raw32"
  VDDM_FCM2NoComDTC_raw32_Inproc/1 -> UnitConverter435/1
  UnitConverter435/1 -> VOUTP_FCM2NoComDTC_raw32/1  "VOUTP_FCM2NoComDTC_raw32"
  VDDM_FCM2RCErrDTC_raw32/1 -> VDDM_FCM2RCErrDTC_raw32_Inproc/1  "VDDM_FCM2RCErrDTC_raw32"
  VDDM_FCM2RCErrDTC_raw32_Inproc/1 -> UnitConverter436/1
  UnitConverter436/1 -> VOUTP_FCM2RCErrDTC_raw32/1  "VOUTP_FCM2RCErrDTC_raw32"
  VDDM_FCM2CSErrDTC_raw32/1 -> VDDM_FCM2CSErrDTC_raw32_Inproc/1  "VDDM_FCM2CSErrDTC_raw32"
  VDDM_FCM2CSErrDTC_raw32_Inproc/1 -> UnitConverter437/1
  UnitConverter437/1 -> VOUTP_FCM2CSErrDTC_raw32/1  "VOUTP_FCM2CSErrDTC_raw32"
  VDDM_FCM3NoComDTC_raw32/1 -> VDDM_FCM3NoComDTC_raw32_Inproc/1  "VDDM_FCM3NoComDTC_raw32"
  VDDM_FCM3NoComDTC_raw32_Inproc/1 -> UnitConverter438/1
  UnitConverter438/1 -> VOUTP_FCM3NoComDTC_raw32/1  "VOUTP_FCM3NoComDTC_raw32"
  VDDM_FCM3RCErrDTC_raw32/1 -> VDDM_FCM3RCErrDTC_raw32_Inproc/1  "VDDM_FCM3RCErrDTC_raw32"
  VDDM_FCM3RCErrDTC_raw32_Inproc/1 -> UnitConverter439/1
  UnitConverter439/1 -> VOUTP_FCM3RCErrDTC_raw32/1  "VOUTP_FCM3RCErrDTC_raw32"
  VDDM_FCM3CSErrDTC_raw32/1 -> VDDM_FCM3CSErrDTC_raw32_Inproc/1  "VDDM_FCM3CSErrDTC_raw32"
  VDDM_FCM3CSErrDTC_raw32_Inproc/1 -> UnitConverter440/1
  UnitConverter440/1 -> VOUTP_FCM3CSErrDTC_raw32/1  "VOUTP_FCM3CSErrDTC_raw32"
  VDDM_FCM4NoComDTC_raw32/1 -> VDDM_FCM4NoComDTC_raw32_Inproc/1  "VDDM_FCM4NoComDTC_raw32"
  VDDM_FCM4NoComDTC_raw32_Inproc/1 -> UnitConverter441/1
  UnitConverter441/1 -> VOUTP_FCM4NoComDTC_raw32/1  "VOUTP_FCM4NoComDTC_raw32"
  VDDM_FCM4CSErrDTC_raw32/1 -> VDDM_FCM4CSErrDTC_raw32_Inproc/1  "VDDM_FCM4CSErrDTC_raw32"
  VDDM_FCM4CSErrDTC_raw32_Inproc/1 -> UnitConverter442/1
  UnitConverter442/1 -> VOUTP_FCM4CSErrDTC_raw32/1  "VOUTP_FCM4CSErrDTC_raw32"
  VDDM_FCM5NoComDTC_raw32/1 -> VDDM_FCM5NoComDTC_raw32_Inproc/1  "VDDM_FCM5NoComDTC_raw32"
  VDDM_FCM5NoComDTC_raw32_Inproc/1 -> UnitConverter443/1
  UnitConverter443/1 -> VOUTP_FCM5NoComDTC_raw32/1  "VOUTP_FCM5NoComDTC_raw32"
  VDDM_FCM5CSErrDTC_raw32/1 -> VDDM_FCM5CSErrDTC_raw32_Inproc/1  "VDDM_FCM5CSErrDTC_raw32"
  VDDM_FCM5CSErrDTC_raw32_Inproc/1 -> UnitConverter444/1
  UnitConverter444/1 -> VOUTP_FCM5CSErrDTC_raw32/1  "VOUTP_FCM5CSErrDTC_raw32"
  VDDM_ZoneSCPNoComDTC_raw32/1 -> VDDM_ZoneSCPNoComDTC_raw32_Inproc/1  "VDDM_ZoneSCPNoComDTC_raw32"
  VDDM_ZoneSCPNoComDTC_raw32_Inproc/1 -> UnitConverter445/1
  UnitConverter445/1 -> VOUTP_ZoneSCPNoComDTC_raw32/1  "VOUTP_ZoneSCPNoComDTC_raw32"
  VDDM_BMSSigErrDetDTC_raw32/1 -> VDDM_BMSSigErrDetDTC_raw32_Inproc/1  "VDDM_BMSSigErrDetDTC_raw32"
  VDDM_BMSSigErrDetDTC_raw32_Inproc/1 -> UnitConverter446/1
  UnitConverter446/1 -> VOUTP_BMSSigErrDetDTC_raw32/1  "VOUTP_BMSSigErrDetDTC_raw32"
  VDDM_FCMACCSigErrDetDTC_raw32/1 -> VDDM_FCMACCSigErrDetDTC_raw32_Inproc/1  "VDDM_FCMACCSigErrDetDTC_raw32"
  VDDM_FCMACCSigErrDetDTC_raw32_Inproc/1 -> UnitConverter447/1
  UnitConverter447/1 -> VOUTP_FCMACCSigErrDetDTC_raw32/1  "VOUTP_FCMACCSigErrDetDTC_raw32"
  VDDM_FrMCUSigErrDetDTC_raw32/1 -> VDDM_FrMCUSigErrDetDTC_raw32_Inproc/1  "VDDM_FrMCUSigErrDetDTC_raw32"
  VDDM_FrMCUSigErrDetDTC_raw32_Inproc/1 -> UnitConverter448/1
  UnitConverter448/1 -> VOUTP_FrMCUSigErrDetDTC_raw32/1  "VOUTP_FrMCUSigErrDetDTC_raw32"
  VDDM_RrMCUSigErrDetDTC_raw32/1 -> VDDM_RrMCUSigErrDetDTC_raw32_Inproc/1  "VDDM_RrMCUSigErrDetDTC_raw32"
  VDDM_RrMCUSigErrDetDTC_raw32_Inproc/1 -> UnitConverter449/1
  UnitConverter449/1 -> VOUTP_RrMCUSigErrDetDTC_raw32/1  "VOUTP_RrMCUSigErrDetDTC_raw32"
  VDDM_CCUSigErrDetDTC_raw32/1 -> VDDM_CCUSigErrDetDTC_raw32_Inproc/1  "VDDM_CCUSigErrDetDTC_raw32"
  VDDM_CCUSigErrDetDTC_raw32_Inproc/1 -> UnitConverter450/1
  UnitConverter450/1 -> VOUTP_CCUSigErrDetDTC_raw32/1  "VOUTP_CCUSigErrDetDTC_raw32"
  VDDM_ACCAccelCmdErrDetDTC_raw32/1 -> VDDM_ACCAccelCmdErrDetDTC_raw32_Inproc/1  "VDDM_ACCAccelCmdErrDetDTC_raw32"
  VDDM_ACCAccelCmdErrDetDTC_raw32_Inproc/1 -> UnitConverter451/1
  UnitConverter451/1 -> VOUTP_ACCAccelCmdErrDetDTC_raw32/1  "VOUTP_ACCAccelCmdErrDetDTC_raw32"
  VDDM_ACCMalfuncDetDTC_raw32/1 -> VDDM_ACCMalfuncDetDTC_raw32_Inproc/1  "VDDM_ACCMalfuncDetDTC_raw32"
  VDDM_ACCMalfuncDetDTC_raw32_Inproc/1 -> UnitConverter452/1
  UnitConverter452/1 -> VOUTP_ACCMalfuncDetDTC_raw32/1  "VOUTP_ACCMalfuncDetDTC_raw32"
  VDDM_CCMalfuncDetDTC_raw32/1 -> VDDM_CCMalfuncDetDTC_raw32_Inproc/1  "VDDM_CCMalfuncDetDTC_raw32"
  VDDM_CCMalfuncDetDTC_raw32_Inproc/1 -> UnitConverter453/1
  UnitConverter453/1 -> VOUTP_CCMalfuncDetDTC_raw32/1  "VOUTP_CCMalfuncDetDTC_raw32"
  VDDM_MSAMalfuncDetDTC_raw32/1 -> VDDM_MSAMalfuncDetDTC_raw32_Inproc/1  "VDDM_MSAMalfuncDetDTC_raw32"
  VDDM_MSAMalfuncDetDTC_raw32_Inproc/1 -> UnitConverter454/1
  UnitConverter454/1 -> VOUTP_MSAMalfuncDetDTC_raw32/1  "VOUTP_MSAMalfuncDetDTC_raw32"
  VDDM_ISAMalfuncDetDTC_raw32/1 -> VDDM_ISAMalfuncDetDTC_raw32_Inproc/1  "VDDM_ISAMalfuncDetDTC_raw32"
  VDDM_ISAMalfuncDetDTC_raw32_Inproc/1 -> UnitConverter455/1
  UnitConverter455/1 -> VOUTP_ISAMalfuncDetDTC_raw32/1  "VOUTP_ISAMalfuncDetDTC_raw32"
  VDDM_MCUF1RCErrDTC_raw32/1 -> VDDM_MCUF1RCErrDTC_raw32_Inproc/1  "VDDM_MCUF1RCErrDTC_raw32"
  VDDM_MCUF1RCErrDTC_raw32_Inproc/1 -> UnitConverter456/1
  UnitConverter456/1 -> VOUTP_MCUF1RCErrDTC_raw32/1  "VOUTP_MCUF1RCErrDTC_raw32"
  VDDM_MCUR1RCErrDTC_raw32/1 -> VDDM_MCUR1RCErrDTC_raw32_Inproc/1  "VDDM_MCUR1RCErrDTC_raw32"
  VDDM_MCUR1RCErrDTC_raw32_Inproc/1 -> UnitConverter457/1
  UnitConverter457/1 -> VOUTP_MCUR1RCErrDTC_raw32/1  "VOUTP_MCUR1RCErrDTC_raw32"
  VDDM_MCUF1CSErrDTC_raw32/1 -> VDDM_MCUF1CSErrDTC_raw32_Inproc/1  "VDDM_MCUF1CSErrDTC_raw32"
  VDDM_MCUF1CSErrDTC_raw32_Inproc/1 -> UnitConverter458/1
  UnitConverter458/1 -> VOUTP_MCUF1CSErrDTC_raw32/1  "VOUTP_MCUF1CSErrDTC_raw32"
  VDDM_MCUR1CSErrDTC_raw32/1 -> VDDM_MCUR1CSErrDTC_raw32_Inproc/1  "VDDM_MCUR1CSErrDTC_raw32"
  VDDM_MCUR1CSErrDTC_raw32_Inproc/1 -> UnitConverter459/1
  UnitConverter459/1 -> VOUTP_MCUR1CSErrDTC_raw32/1  "VOUTP_MCUR1CSErrDTC_raw32"
  VDDM_Shifter1RCErrDTC_raw32/1 -> VDDM_Shifter1RCErrDTC_raw32_Inproc/1  "VDDM_Shifter1RCErrDTC_raw32"
  VDDM_Shifter1RCErrDTC_raw32_Inproc/1 -> UnitConverter460/1
  UnitConverter460/1 -> VOUTP_Shifter1RCErrDTC_raw32/1  "VOUTP_Shifter1RCErrDTC_raw32"
  VDDM_Shifter1CSErrDTC_raw32/1 -> VDDM_Shifter1CSErrDTC_raw32_Inproc/1  "VDDM_Shifter1CSErrDTC_raw32"
  VDDM_Shifter1CSErrDTC_raw32_Inproc/1 -> UnitConverter461/1
  UnitConverter461/1 -> VOUTP_Shifter1CSErrDTC_raw32/1  "VOUTP_Shifter1CSErrDTC_raw32"
  VDDM_ESC7RCErrDTC_raw32/1 -> VDDM_ESC7RCErrDTC_raw32_Inproc/1  "VDDM_ESC7RCErrDTC_raw32"
  VDDM_ESC7RCErrDTC_raw32_Inproc/1 -> UnitConverter462/1
  UnitConverter462/1 -> VOUTP_ESC7RCErrDTC_raw32/1  "VOUTP_ESC7RCErrDTC_raw32"
  VDDM_ESC7CSErrDTC_raw32/1 -> VDDM_ESC7CSErrDTC_raw32_Inproc/1  "VDDM_ESC7CSErrDTC_raw32"
  VDDM_ESC7CSErrDTC_raw32_Inproc/1 -> UnitConverter463/1
  UnitConverter463/1 -> VOUTP_ESC7CSErrDTC_raw32/1  "VOUTP_ESC7CSErrDTC_raw32"
  VDDM_ESC1RCErrDTC_raw32/1 -> VDDM_ESC1RCErrDTC_raw32_Inproc/1  "VDDM_ESC1RCErrDTC_raw32"
  VDDM_ESC1RCErrDTC_raw32_Inproc/1 -> UnitConverter464/1
  UnitConverter464/1 -> VOUTP_ESC1RCErrDTC_raw32/1  "VOUTP_ESC1RCErrDTC_raw32"
  VDDM_ESC1CSErrDTC_raw32/1 -> VDDM_ESC1CSErrDTC_raw32_Inproc/1  "VDDM_ESC1CSErrDTC_raw32"
  VDDM_ESC1CSErrDTC_raw32_Inproc/1 -> UnitConverter465/1
  UnitConverter465/1 -> VOUTP_ESC1CSErrDTC_raw32/1  "VOUTP_ESC1CSErrDTC_raw32"
  VDDM_ESC5RCErrDTC_raw32/1 -> VDDM_ESC5RCErrDTC_raw32_Inproc/1  "VDDM_ESC5RCErrDTC_raw32"
  VDDM_ESC5RCErrDTC_raw32_Inproc/1 -> UnitConverter466/1
  UnitConverter466/1 -> VOUTP_ESC5RCErrDTC_raw32/1  "VOUTP_ESC5RCErrDTC_raw32"
  VDDM_ESC5CSErrDTC_raw32/1 -> VDDM_ESC5CSErrDTC_raw32_Inproc/1  "VDDM_ESC5CSErrDTC_raw32"
  VDDM_ESC5CSErrDTC_raw32_Inproc/1 -> UnitConverter467/1
  UnitConverter467/1 -> VOUTP_ESC5CSErrDTC_raw32/1  "VOUTP_ESC5CSErrDTC_raw32"
  VDDM_FrMCUTqErrDTC_raw32/1 -> VDDM_FrMCUTqErrDTC_raw32_Inproc/1  "VDDM_FrMCUTqErrDTC_raw32"
  VDDM_FrMCUTqErrDTC_raw32_Inproc/1 -> UnitConverter468/1
  UnitConverter468/1 -> VOUTP_FrMCUTqErrDTC_raw32/1  "VOUTP_FrMCUTqErrDTC_raw32"
  VDDM_RrMCUTqErrDTC_raw32/1 -> VDDM_RrMCUTqErrDTC_raw32_Inproc/1  "VDDM_RrMCUTqErrDTC_raw32"
  VDDM_RrMCUTqErrDTC_raw32_Inproc/1 -> UnitConverter469/1
  UnitConverter469/1 -> VOUTP_RrMCUTqErrDTC_raw32/1  "VOUTP_RrMCUTqErrDTC_raw32"
  VDDM_LFBatwarnDTC_raw32/1 -> VDDM_LFBatwarnDTC_raw32_Inproc/1  "VDDM_LFBatwarnDTC_raw32"
  VDDM_LFBatwarnDTC_raw32_Inproc/1 -> UnitConverter470/1
  UnitConverter470/1 -> VOUTP_LFBatwarnDTC_raw32/1  "VOUTP_LFBatwarnDTC_raw32"
  VDDM_RFBatwarnDTC_raw32/1 -> VDDM_RFBatwarnDTC_raw32_Inproc/1  "VDDM_RFBatwarnDTC_raw32"
  VDDM_RFBatwarnDTC_raw32_Inproc/1 -> UnitConverter471/1
  UnitConverter471/1 -> VOUTP_RFBatwarnDTC_raw32/1  "VOUTP_RFBatwarnDTC_raw32"
  VDDM_LRBatwarnDTC_raw32/1 -> VDDM_LRBatwarnDTC_raw32_Inproc/1  "VDDM_LRBatwarnDTC_raw32"
  VDDM_LRBatwarnDTC_raw32_Inproc/1 -> UnitConverter472/1
  UnitConverter472/1 -> VOUTP_LRBatwarnDTC_raw32/1  "VOUTP_LRBatwarnDTC_raw32"
  VDDM_RRBatwarnDTC_raw32/1 -> VDDM_RRBatwarnDTC_raw32_Inproc/1  "VDDM_RRBatwarnDTC_raw32"
  VDDM_RRBatwarnDTC_raw32_Inproc/1 -> UnitConverter473/1
  UnitConverter473/1 -> VOUTP_RRBatwarnDTC_raw32/1  "VOUTP_RRBatwarnDTC_raw32"
  VDDM_LFPressIndiDTC_raw32/1 -> VDDM_LFPressIndiDTC_raw32_Inproc/1  "VDDM_LFPressIndiDTC_raw32"
  VDDM_LFPressIndiDTC_raw32_Inproc/1 -> UnitConverter474/1
  UnitConverter474/1 -> VOUTP_LFPressIndiDTC_raw32/1  "VOUTP_LFPressIndiDTC_raw32"
  VDDM_RFPressIndiDTC_raw32/1 -> VDDM_RFPressIndiDTC_raw32_Inproc/1  "VDDM_RFPressIndiDTC_raw32"
  VDDM_RFPressIndiDTC_raw32_Inproc/1 -> UnitConverter475/1
  UnitConverter475/1 -> VOUTP_RFPressIndiDTC_raw32/1  "VOUTP_RFPressIndiDTC_raw32"
  VDDM_LRPressIndiDTC_raw32/1 -> VDDM_LRPressIndiDTC_raw32_Inproc/1  "VDDM_LRPressIndiDTC_raw32"
  VDDM_LRPressIndiDTC_raw32_Inproc/1 -> UnitConverter476/1
  UnitConverter476/1 -> VOUTP_LRPressIndiDTC_raw32/1  "VOUTP_LRPressIndiDTC_raw32"
  VDDM_RRPressIndiDTC_raw32/1 -> VDDM_RRPressIndiDTC_raw32_Inproc/1  "VDDM_RRPressIndiDTC_raw32"
  VDDM_RRPressIndiDTC_raw32_Inproc/1 -> UnitConverter477/1
  UnitConverter477/1 -> VOUTP_RRPressIndiDTC_raw32/1  "VOUTP_RRPressIndiDTC_raw32"
  VDDM_LFWheelTmpHighDTC_raw32/1 -> VDDM_LFWheelTmpHighDTC_raw32_Inproc/1  "VDDM_LFWheelTmpHighDTC_raw32"
  VDDM_LFWheelTmpHighDTC_raw32_Inproc/1 -> UnitConverter478/1
  UnitConverter478/1 -> VOUTP_LFWheelTmpHighDTC_raw32/1  "VOUTP_LFWheelTmpHighDTC_raw32"
  VDDM_RFWheelTmpHighDTC_raw32/1 -> VDDM_RFWheelTmpHighDTC_raw32_Inproc/1  "VDDM_RFWheelTmpHighDTC_raw32"
  VDDM_RFWheelTmpHighDTC_raw32_Inproc/1 -> UnitConverter479/1
  UnitConverter479/1 -> VOUTP_RFWheelTmpHighDTC_raw32/1  "VOUTP_RFWheelTmpHighDTC_raw32"
  VDDM_LRWheelTmpHighDTC_raw32/1 -> VDDM_LRWheelTmpHighDTC_raw32_Inproc/1  "VDDM_LRWheelTmpHighDTC_raw32"
  VDDM_LRWheelTmpHighDTC_raw32_Inproc/1 -> UnitConverter480/1
  UnitConverter480/1 -> VOUTP_LRWheelTmpHighDTC_raw32/1  "VOUTP_LRWheelTmpHighDTC_raw32"
  VDDM_RRWheelTmpHighDTC_raw32/1 -> VDDM_RRWheelTmpHighDTC_raw32_Inproc/1  "VDDM_RRWheelTmpHighDTC_raw32"
  VDDM_RRWheelTmpHighDTC_raw32_Inproc/1 -> UnitConverter481/1
  UnitConverter481/1 -> VOUTP_RRWheelTmpHighDTC_raw32/1  "VOUTP_RRWheelTmpHighDTC_raw32"
  VDDM_LFSensorFailDTC_raw32/1 -> VDDM_LFSensorFailDTC_raw32_Inproc/1  "VDDM_LFSensorFailDTC_raw32"
  VDDM_LFSensorFailDTC_raw32_Inproc/1 -> UnitConverter482/1
  UnitConverter482/1 -> VOUTP_LFSensorFailDTC_raw32/1  "VOUTP_LFSensorFailDTC_raw32"
  VDDM_RFSensorFailDTC_raw32/1 -> VDDM_RFSensorFailDTC_raw32_Inproc/1  "VDDM_RFSensorFailDTC_raw32"
  VDDM_RFSensorFailDTC_raw32_Inproc/1 -> UnitConverter483/1
  UnitConverter483/1 -> VOUTP_RFSensorFailDTC_raw32/1  "VOUTP_RFSensorFailDTC_raw32"
  VDDM_LRSensorFailDTC_raw32/1 -> VDDM_LRSensorFailDTC_raw32_Inproc/1  "VDDM_LRSensorFailDTC_raw32"
  VDDM_LRSensorFailDTC_raw32_Inproc/1 -> UnitConverter484/1
  UnitConverter484/1 -> VOUTP_LRSensorFailDTC_raw32/1  "VOUTP_LRSensorFailDTC_raw32"
  VDDM_RRSensorFailDTC_raw32/1 -> VDDM_RRSensorFailDTC_raw32_Inproc/1  "VDDM_RRSensorFailDTC_raw32"
  VDDM_RRSensorFailDTC_raw32_Inproc/1 -> UnitConverter485/1
  UnitConverter485/1 -> VOUTP_RRSensorFailDTC_raw32/1  "VOUTP_RRSensorFailDTC_raw32"
  VDDM_C1EPAS2LCDTC_raw32/1 -> VDDM_C1EPAS2LCDTC_raw32_Inproc/1  "VDDM_C1EPAS2LCDTC_raw32"
  VDDM_C1EPAS2LCDTC_raw32_Inproc/1 -> UnitConverter486/1
  UnitConverter486/1 -> VOUTP_C1EPAS2LCDTC_raw32/1  "VOUTP_C1EPAS2LCDTC_raw32"
  VDDM_5vAPS1PwrErrDTC_raw32/1 -> VDDM_5vAPS1PwrErrDTC_raw32_Inproc/1  "VDDM_5vAPS1PwrErrDTC_raw32"
  VDDM_5vAPS1PwrErrDTC_raw32_Inproc/1 -> UnitConverter487/1
  UnitConverter487/1 -> VOUTP_5vAPS1PwrErrDTC_raw32/1  "VOUTP_5vAPS1PwrErrDTC_raw32"
  VDDM_5vAPS2PwrErrDTC_raw32/1 -> VDDM_5vAPS2PwrErrDTC_raw32_Inproc/1  "VDDM_5vAPS2PwrErrDTC_raw32"
  VDDM_5vAPS2PwrErrDTC_raw32_Inproc/1 -> UnitConverter488/1
  UnitConverter488/1 -> VOUTP_5vAPS2PwrErrDTC_raw32/1  "VOUTP_5vAPS2PwrErrDTC_raw32"
  VDDM_EPBLockTODTC_raw32/1 -> VDDM_EPBLockTODTC_raw32_Inproc/1  "VDDM_EPBLockTODTC_raw32"
  VDDM_EPBLockTODTC_raw32_Inproc/1 -> UnitConverter489/1
  UnitConverter489/1 -> VOUTP_EPBLockTODTC_raw32/1  "VOUTP_EPBLockTODTC_raw32"
  VDDM_EPBUnlockTODTC_raw32/1 -> VDDM_EPBUnlockTODTC_raw32_Inproc/1  "VDDM_EPBUnlockTODTC_raw32"
  VDDM_EPBUnlockTODTC_raw32_Inproc/1 -> UnitConverter490/1
  UnitConverter490/1 -> VOUTP_EPBUnlockTODTC_raw32/1  "VOUTP_EPBUnlockTODTC_raw32"
  VDDM_LimpHomeActTmp_flg/1 -> VDDM_LimpHomeActTmp_flg_Inproc/1  "VDDM_LimpHomeActTmp_flg"
  VDDM_LimpHomeActTmp_flg_Inproc/1 -> UnitConverter491/1
  UnitConverter491/1 -> VOUTP_LimpHomeActTmp_flg/1  "VOUTP_LimpHomeActTmp_flg"
  VDDM_DTCDetect_enum/1 -> VDDM_DTCDetect_enum_Inproc/1  "VDDM_DTCDetect_enum"
  VDDM_DTCDetect_enum_Inproc/1 -> UnitConverter492/1
  UnitConverter492/1 -> VOUTP_DTCDetect_enum/1  "VOUTP_DTCDetect_enum"
  VDDM_EngagePFail_flg/1 -> VDDM_EngagePFail_flg_Inproc/1  "VDDM_EngagePFail_flg"
  VDDM_EngagePFail_flg_Inproc/1 -> UnitConverter493/1
  UnitConverter493/1 -> VOUTP_EngagePFail_flg/1  "VOUTP_EngagePFail_flg"
  VDDM_DisengagePFail_flg/1 -> VDDM_DisengagePFail_flg_Inproc/1  "VDDM_DisengagePFail_flg"
  VDDM_DisengagePFail_flg_Inproc/1 -> UnitConverter494/1
  UnitConverter494/1 -> VOUTP_DisengagePFail_flg/1  "VOUTP_DisengagePFail_flg"
  VDDM_VCURAPSErrLv2_flg/1 -> VDDM_VCURAPSErrLv2_flg_Inproc/1  "VDDM_VCURAPSErrLv2_flg"
  VDDM_VCURAPSErrLv2_flg_Inproc/1 -> UnitConverter495/1
  UnitConverter495/1 -> VOUTP_VCURAPSErrLv2_flg/1  "VOUTP_VCURAPSErrLv2_flg"
  VDDM_VCURAPSErrLv3_flg/1 -> VDDM_VCURAPSErrLv3_flg_Inproc/1  "VDDM_VCURAPSErrLv3_flg"
  VDDM_VCURAPSErrLv3_flg_Inproc/1 -> UnitConverter496/1
  UnitConverter496/1 -> VOUTP_VCURAPSErrLv3_flg/1  "VOUTP_VCURAPSErrLv3_flg"
  VDDM_EDriveSysErrShifterErr_flg/1 -> VDDM_EDriveSysErrShifterErr_flg_Inproc/1  "VDDM_EDriveSysErrShifterErr_flg"
  VDDM_EDriveSysErrShifterErr_flg_Inproc/1 -> UnitConverter497/1
  UnitConverter497/1 -> VOUTP_EDriveSysErrShifterErr_flg/1  "VOUTP_EDriveSysErrShifterErr_flg"
  VDDM_LVSysErrPwrOutErr_flg/1 -> VDDM_LVSysErrPwrOutErr_flg_Inproc/1  "VDDM_LVSysErrPwrOutErr_flg"
  VDDM_LVSysErrPwrOutErr_flg_Inproc/1 -> UnitConverter498/1
  UnitConverter498/1 -> VOUTP_LVSysErrPwrOutErr_flg/1  "VOUTP_LVSysErrPwrOutErr_flg"
  VDDM_HVRlyOpFail_flg/1 -> VDDM_HVRlyOpFail_flg_Inproc/1  "VDDM_HVRlyOpFail_flg"
  VDDM_HVRlyOpFail_flg_Inproc/1 -> UnitConverter499/1
  UnitConverter499/1 -> VOUTP_HVRlyOpFail_flg/1  "VOUTP_HVRlyOpFail_flg"
  VDDM_MCUActDisFail_flg/1 -> VDDM_MCUActDisFail_flg_Inproc/1  "VDDM_MCUActDisFail_flg"
  VDDM_MCUActDisFail_flg_Inproc/1 -> UnitConverter500/1
  UnitConverter500/1 -> VOUTP_MCUActDisFail_flg/1  "VOUTP_MCUActDisFail_flg"
  VDDM_VCUBrkSWSta_enum/1 -> VDDM_VCUBrkSWSta_enum_Inproc/1  "VDDM_VCUBrkSWSta_enum"
  VDDM_VCUBrkSWSta_enum_Inproc/1 -> UnitConverter501/1
  UnitConverter501/1 -> VOUTP_VCUBrkSWSta_enum/1  "VOUTP_VCUBrkSWSta_enum"
  VDDM_VCUFLDoorSta_flg/1 -> VDDM_VCUFLDoorSta_flg_Inproc/1  "VDDM_VCUFLDoorSta_flg"
  VDDM_VCUFLDoorSta_flg_Inproc/1 -> UnitConverter502/1
  UnitConverter502/1 -> VOUTP_VCUFLDoorSta_flg/1  "VOUTP_VCUFLDoorSta_flg"
  VDDM_VCUFRDoorSta_flg/1 -> VDDM_VCUFRDoorSta_flg_Inproc/1  "VDDM_VCUFRDoorSta_flg"
  VDDM_VCUFRDoorSta_flg_Inproc/1 -> UnitConverter503/1
  UnitConverter503/1 -> VOUTP_VCUFRDoorSta_flg/1  "VOUTP_VCUFRDoorSta_flg"
  VDDM_VCURLDoorSta_flg/1 -> VDDM_VCURLDoorSta_flg_Inproc/1  "VDDM_VCURLDoorSta_flg"
  VDDM_VCURLDoorSta_flg_Inproc/1 -> UnitConverter504/1
  UnitConverter504/1 -> VOUTP_VCURLDoorSta_flg/1  "VOUTP_VCURLDoorSta_flg"
  VDDM_VCURRDoorSta_flg/1 -> VDDM_VCURRDoorSta_flg_Inproc/1  "VDDM_VCURRDoorSta_flg"
  VDDM_VCURRDoorSta_flg_Inproc/1 -> UnitConverter505/1
  UnitConverter505/1 -> VOUTP_VCURRDoorSta_flg/1  "VOUTP_VCURRDoorSta_flg"
  VDDM_SysAllowReadySta_flg/1 -> VDDM_SysAllowReadySta_flg_Inproc/1  "VDDM_SysAllowReadySta_flg"
  VDDM_SysAllowReadySta_flg_Inproc/1 -> UnitConverter506/1
  UnitConverter506/1 -> VOUTP_SysAllowReadySta_flg/1  "VOUTP_SysAllowReadySta_flg"
  VDDM_VCUHoodSWSta_flg/1 -> VDDM_VCUHoodSWSta_flg_Inproc/1  "VDDM_VCUHoodSWSta_flg"
  VDDM_VCUHoodSWSta_flg_Inproc/1 -> UnitConverter507/1
  UnitConverter507/1 -> VOUTP_VCUHoodSWSta_flg/1  "VOUTP_VCUHoodSWSta_flg"
  VDDM_VCUTailgateSWSta_flg/1 -> VDDM_VCUTailgateSWSta_flg_Inproc/1  "VDDM_VCUTailgateSWSta_flg"
  VDDM_VCUTailgateSWSta_flg_Inproc/1 -> UnitConverter508/1
  UnitConverter508/1 -> VOUTP_VCUTailgateSWSta_flg/1  "VOUTP_VCUTailgateSWSta_flg"
  VDDM_CAN1BusErrorDTC_raw32/1 -> VDDM_CAN1BusErrorDTC_raw32_Inproc/1  "VDDM_CAN1BusErrorDTC_raw32"
  VDDM_CAN1BusErrorDTC_raw32_Inproc/1 -> UnitConverter509/1
  UnitConverter509/1 -> VOUTP_CAN1BusErrorDTC_raw32/1  "VOUTP_CAN1BusErrorDTC_raw32"
  VDDM_CAN2BusErrorDTC_raw32/1 -> VDDM_CAN2BusErrorDTC_raw32_Inproc/1  "VDDM_CAN2BusErrorDTC_raw32"
  VDDM_CAN2BusErrorDTC_raw32_Inproc/1 -> UnitConverter510/1
  UnitConverter510/1 -> VOUTP_CAN2BusErrorDTC_raw32/1  "VOUTP_CAN2BusErrorDTC_raw32"
  VDDM_CAN3BusErrorDTC_raw32/1 -> VDDM_CAN3BusErrorDTC_raw32_Inproc/1  "VDDM_CAN3BusErrorDTC_raw32"
  VDDM_CAN3BusErrorDTC_raw32_Inproc/1 -> UnitConverter511/1
  UnitConverter511/1 -> VOUTP_CAN3BusErrorDTC_raw32/1  "VOUTP_CAN3BusErrorDTC_raw32"
  VDDM_CAN4BusErrorDTC_raw32/1 -> VDDM_CAN4BusErrorDTC_raw32_Inproc/1  "VDDM_CAN4BusErrorDTC_raw32"
  VDDM_CAN4BusErrorDTC_raw32_Inproc/1 -> UnitConverter512/1
  UnitConverter512/1 -> VOUTP_CAN4BusErrorDTC_raw32/1  "VOUTP_CAN4BusErrorDTC_raw32"
  VDDM_CAN5BusErrorDTC_raw32/1 -> VDDM_CAN5BusErrorDTC_raw32_Inproc/1  "VDDM_CAN5BusErrorDTC_raw32"
  VDDM_CAN5BusErrorDTC_raw32_Inproc/1 -> UnitConverter513/1
  UnitConverter513/1 -> VOUTP_CAN5BusErrorDTC_raw32/1  "VOUTP_CAN5BusErrorDTC_raw32"
  VDDM_CAN6BusErrorDTC_raw32/1 -> VDDM_CAN6BusErrorDTC_raw32_Inproc/1  "VDDM_CAN6BusErrorDTC_raw32"
  VDDM_CAN6BusErrorDTC_raw32_Inproc/1 -> UnitConverter514/1
  UnitConverter514/1 -> VOUTP_CAN6BusErrorDTC_raw32/1  "VOUTP_CAN6BusErrorDTC_raw32"
  VDHP_ActAPSPosn_pct/1 -> VDHP_ActAPSPosn_pct_Inproc/1  "VDHP_ActAPSPosn_pct"
  VDHP_ActAPSPosn_pct_Inproc/1 -> UnitConverter515/1
  UnitConverter515/1 -> VOUTP_ActAPSPosn_pct/1  "VOUTP_ActAPSPosn_pct"
  VDHP_EAPS1MIN_pct/1 -> VDHP_EAPS1MIN_pct_Inproc/1  "VDHP_EAPS1MIN_pct"
  VDHP_EAPS1MIN_pct_Inproc/1 -> UnitConverter516/1
  UnitConverter516/1 -> VOUTP_EAPS1MIN_pct/1  "VOUTP_EAPS1MIN_pct"
  VDHP_EAPS2MIN_pct/1 -> VDHP_EAPS2MIN_pct_Inproc/1  "VDHP_EAPS2MIN_pct"
  VDHP_EAPS2MIN_pct_Inproc/1 -> UnitConverter517/1
  UnitConverter517/1 -> VOUTP_EAPS2MIN_pct/1  "VOUTP_EAPS2MIN_pct"
  VDHP_ResetPedalZeroPosStart_flg/1 -> VDHP_ResetPedalZeroPosStart_flg_Inproc/1  "VDHP_ResetPedalZeroPosStart_flg"
  VDHP_ResetPedalZeroPosStart_flg_Inproc/1 -> UnitConverter518/1
  UnitConverter518/1 -> VOUTP_ResetPedalZeroPosStart_flg/1  "VOUTP_ResetPedalZeroPosStart_flg"
  VDHP_EAPS1NRM_pct/1 -> VDHP_EAPS1NRM_pct_Inproc/1  "VDHP_EAPS1NRM_pct"
  VDHP_EAPS1NRM_pct_Inproc/1 -> UnitConverter519/1
  UnitConverter519/1 -> VOUTP_EAPS1NRM_pct/1  "VOUTP_EAPS1NRM_pct"
  VDHP_EAPS2NRM_pct/1 -> VDHP_EAPS2NRM_pct_Inproc/1  "VDHP_EAPS2NRM_pct"
  VDHP_EAPS2NRM_pct_Inproc/1 -> UnitConverter520/1
  UnitConverter520/1 -> VOUTP_EAPS2NRM_pct/1  "VOUTP_EAPS2NRM_pct"
  VDKC_DKCTimeSN_cnt/1 -> VDKC_DKCTimeSN_cnt_Inproc/1  "VDKC_DKCTimeSN_cnt"
  VDKC_DKCTimeSN_cnt_Inproc/1 -> UnitConverter521/1
  UnitConverter521/1 -> VOUTP_DKCTimeSN_cnt/1  "VOUTP_DKCTimeSN_cnt"
  VDKC_DKCAuthSta_enum/1 -> VDKC_DKCAuthSta_enum_Inproc/1  "VDKC_DKCAuthSta_enum"
  VDKC_DKCAuthSta_enum_Inproc/1 -> UnitConverter522/1
  UnitConverter522/1 -> VOUTP_DKCAuthSta_enum/1  "VOUTP_DKCAuthSta_enum"
  VDKC_TimeSNDKCFbk_cnt/1 -> VDKC_TimeSNDKCFbk_cnt_Inproc/1  "VDKC_TimeSNDKCFbk_cnt"
  VDKC_TimeSNDKCFbk_cnt_Inproc/1 -> UnitConverter523/1
  UnitConverter523/1 -> VOUTP_TimeSNDKCFbk_cnt/1  "VOUTP_TimeSNDKCFbk_cnt"
  VDKC_KeyMissSta_flg/1 -> VDKC_KeyMissSta_flg_Inproc/1  "VDKC_KeyMissSta_flg"
  VDKC_KeyMissSta_flg_Inproc/1 -> UnitConverter524/1
  UnitConverter524/1 -> VOUTP_KeyMissSta_flg/1  "VOUTP_KeyMissSta_flg"
  VDKC_KeyModeSta_enum/1 -> VDKC_KeyModeSta_enum_Inproc/1  "VDKC_KeyModeSta_enum"
  VDKC_KeyModeSta_enum_Inproc/1 -> UnitConverter525/1
  UnitConverter525/1 -> VOUTP_KeyModeSta_enum/1  "VOUTP_KeyModeSta_enum"
  VDKC_DkeyShowIVISta_enum/1 -> VDKC_DkeyShowIVISta_enum_Inproc/1  "VDKC_DkeyShowIVISta_enum"
  VDKC_DkeyShowIVISta_enum_Inproc/1 -> UnitConverter526/1
  UnitConverter526/1 -> VOUTP_DkeyShowIVISta_enum/1  "VOUTP_DkeyShowIVISta_enum"
  VDKC_KeyAreaPS_enum/1 -> VDKC_KeyAreaPS_enum_Inproc/1  "VDKC_KeyAreaPS_enum"
  VDKC_KeyAreaPS_enum_Inproc/1 -> UnitConverter527/1
  UnitConverter527/1 -> VOUTP_KeyAreaPS_enum/1  "VOUTP_KeyAreaPS_enum"
  VDKC_KeyAreaLockUnlock_enum/1 -> VDKC_KeyAreaLockUnlock_enum_Inproc/1  "VDKC_KeyAreaLockUnlock_enum"
  VDKC_KeyAreaLockUnlock_enum_Inproc/1 -> UnitConverter528/1
  UnitConverter528/1 -> VOUTP_KeyAreaLockUnlock_enum/1  "VOUTP_KeyAreaLockUnlock_enum"
